simulink library "outp"  (R2021b)
settings: Solver=VariableStepAuto  StartTime=0.0  StopTime=10.0  RelTol=1e-3
undefined symbols (not defined in the file or in its folder): ENUM_PMMMODE_CHARGE, ENUM_PMMMODE_IDLE, ENUM_PMMMODE_INITIALIZE, ENUM_PMMMODE_POWERDOWN, ENUM_PMMMODE_SLEEP, Left, outp, slcm, TRUE
libraries: FVT_lib x736, hcu_lib x4, simulink x1
(part 2 of 8)

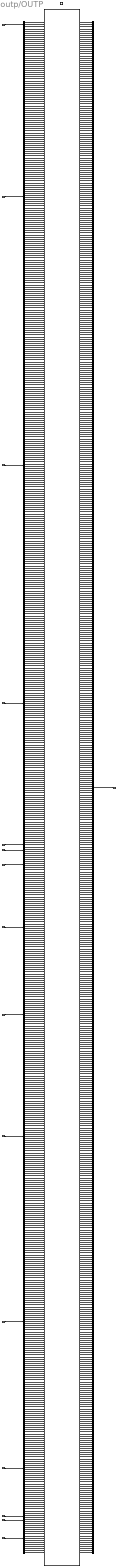
== system outp/OUTP ==
  BACC_outputs : Inport  OutDataTypeStr=Bus: BACC_outputs
  BAPM_outputs : Inport  Port=2  OutDataTypeStr=Bus: BAPM_outputs
  BBCM_outputs : Inport  Port=3  OutDataTypeStr=Bus: BBCM_outputs
  BDDM_outputs : Inport  Port=4  OutDataTypeStr=Bus: BDDM_outputs
  BDHP_outputs : Inport  Port=5  OutDataTypeStr=Bus: BDHP_outputs
  BDKC_outputs : Inport  Port=6  OutDataTypeStr=Bus: BDKC_outputs
  BNMM_outputs : Inport  Port=7  OutDataTypeStr=Bus: BNMM_outputs
  BPMM_outputs : Inport  Port=8  OutDataTypeStr=Bus: BPMM_outputs
  BSYS_outputs : Inport  Port=9  OutDataTypeStr=Bus: BSYS_outputs
  BTHC_outputs : Inport  Port=10  OutDataTypeStr=Bus: BTHC_outputs
  BTPM_outputs : Inport  Port=11  OutDataTypeStr=Bus: BTPM_outputs
  BTQD_outputs : Inport  Port=12  OutDataTypeStr=Bus: BTQD_outputs
  BTQR_outputs : Inport  Port=13  OutDataTypeStr=Bus: BTQR_outputs
  BV2L_outputs : Inport  Port=14  OutDataTypeStr=Bus: BV2L_outputs
  BVMC_outputs : Inport  Port=15  OutDataTypeStr=Bus: BVMC_outputs
  trig_OUTP : TriggerPort  TriggerType=function-call  VariantControl=(inherit)
  bus_creator : BusCreator  Inputs=736
  bus_selector1 : BusSelector  OutputSignals=VACC_HVTHCMSysAvail_enum,VACC_LVBattVoltSta_enum,VACC_VehHVPwrAvail4THCM_W
  bus_selector10 : BusSelector  OutputSignals=VTHC_FDCompCmd_rpm,VTHC_FDSOV1Cmd_flg,VTHC_FDSOV2Cmd_flg,VTHC_FDSOV3Cmd_flg,VTHC_FDEXV1Cmd_step,VTHC_FDEXV2Cmd_step,VTHC_FDSOTXVCmd_flg,VTHC_FDFWVCmd_flg,VTHC_FDTWVCmd_pct,VTHC_FDFrWPTCHeatPwrCmd_W,VTHC_CoolgFanActDuty_pct,VTHC_FDAGSCmd_enum,VTHC_FDEWP1Cmd_enum,VTHC_FDEWP2Cmd_enum,VTHC_FDEWP3Cmd_enum,VTHC_FDFrLeAPTCHeatPwrCmd_W,VTHC_FDFrRiAPTCHeatPwrCmd_W,VTHC_FDRrAPTCHeatPwrCmd_W,VTHC_FDBlowerCmd_pct,VTHC_BatteryMode_enum,VTHC_EDriveMode_enum,VTHC_CabinMode_enum,VTHC_CCUACLampSts_flg,VTHC_CCUAutoLampSts_flg,VTHC_CCUACMaxLampSts_flg,VTHC_CCUSyncLampSts_flg,VTHC_sigAirIntenZon1St_enum,VTHC_sigWindDirZon1St_enum,VTHC_sigRecircSt_flg,VTHC_sigSetTempZon1St_C,VTHC_sigSetTempZon2St_C,VTHC_sigClntTHvBattOut_C,VTHC_sigCbnSolarLeft_W,VTHC_sigClntTHvBattIn_C,VTHC_sigCbnSolarRight_W,VTHC_sigAmbAirT_C,VTHC_sigCbnAirT_C,VTHC_ACSubMode_enum,VTHC_FDRecyAutoCmd_enum,VTHC_ACModeMem_enum,VTHC_Face_flg,VTHC_Foot_flg,VTHC_Frost_flg,VTHC_FaceM_flg,VTHC_FootM_flg,VTHC_CCUSyncSts_flg,VTHC_ACForceOFF_flg,VTHC_RecAutoFlg_flg,VTHC_AirIntenZone1M_enum,VTHC_fdefog_flg,VTHC_sigSetTempZon2StM_C,VTHC_sigDfrstSt_flg,VTHC_FDCTHCAirIntZ3Sta_enum,VTHC_FDCTHCDrEVentModeSta_enum,VTHC_FDCTHCPsEVentModeSta_enum,VTHC_FDCTHCDrEVentZSta_enum,VTHC_FDCTHCCLEVentZSta_enum,VTHC_FDCTHCPsEVentZSta_enum,VTHC_FDCTHCCREVentZSta_enum,VTHC_FDCTHCDrEVentYSta_enum,VTHC_FDCTHCDrVentENSta_flg,VTHC_FDCTHCCLEVentYSta_enum,VTHC_FDCTHCCLVentENSta_flg,VTHC_FDCTHCPsEVentYSta_enum,VTHC_FDCTHCPsVentENSta_flg,VTHC_FDCTHCCREVentYSta_enum,VTHC_FDCTHCCRVentENSta_flg,VTHC_FDCTHCMAPTCForceOFFSta_flg,VTHC_DrVentEN_flg,VTHC_CLVentEN_flg,VTHC_PsVentEN_flg,VTHC_CRVentEN_flg,VTHC_FDCFGSAirIntSta_enum,VTHC_FDCFGSChSta_enum,VTHC_FDCFGSAirIntCmd_enum,VTHC_FDCFGSFuncSta_flg,VTHC_FDCFGSChCmd_enum,VTHC_FDCFGSIONSWSta_flg,VTHC_FDCFGSIONCmd_flg,VTHC_FDCFGSLearnCmd_enum,VTHC_FDCTHCMPreWPTCHeatSta_enum
  bus_selector11 : BusSelector  OutputSignals=VTPM_LFBatWarn_flg,VTPM_RFBatWarn_flg,VTPM_LRBatWarn_flg,VTPM_RRBatWarn_flg,VTPM_LFWheelPress_raw8,VTPM_RFWheelPress_raw8,VTPM_LRWheelPress_raw8,VTPM_RRWheelPress_raw8,VTPM_LFWheelTemp_C,VTPM_RFWheelTemp_C,VTPM_LRWheelTemp_C,VTPM_RRWheelTemp_C,VTPM_LFSensorFail_flg,VTPM_RFSensorFail_flg,VTPM_LRSensorFail_flg,VTPM_RRSensorFail_flg,VTPM_LFWheelDebug_flg,VTPM_LRWheelDebug_flg,VTPM_RFWheelDebug_flg,VTPM_RRWheelDebug_flg,VTPM_TPMSResButtAllow_flg,VTPM_TPMSCaliButtAllow_flg,VTPM_LFPressIndi_enum,VTPM_RFPressIndi_enum,VTPM_LRPressIndi_enum,VTPM_RRPressIndi_enum,VTPM_TPMSWarnIndi_enum,VTPM_LFWheelTmpIndi_flg,VTPM_RFWheelTmpIndi_flg,VTPM_LRWheelTmpIndi_flg,VTPM_RRWheelTmpIndi_flg,VTPM_LFWheelPSW_raw8,VTPM_LRWheelPSW_raw8,VTPM_RFWheelPSW_raw8,VTPM_RRWheelPSW_raw8,VTPM_CWheelTips_enum,VTPM_AutoLTips_enum,VTPM_LFSensorMode_flg,VTPM_RFSensorMode_flg,VTPM_LRSensorMode_flg,VTPM_RRSensorMode_flg,VTPM_S1ID_raw32,VTPM_S2ID_raw32,VTPM_S3ID_raw32,VTPM_S4ID_raw32,VTPM_S1L_enum,VTPM_S2L_enum,VTPM_S3L_enum,VTPM_S4L_enum,VTPM_ALFin_flg,VTPM_LFP20_raw8,VTPM_RFP20_raw8,VTPM_LRP20_raw8,VTPM_RRP20_raw8,VTPM_FAT_flg,VTPM_IDin_raw32,VTPM_S1WheelDebugALTU_pct,VTPM_S2WheelDebugALTU_pct,VTPM_S3WheelDebugALTU_pct,VTPM_S4WheelDebugALTU_pct,VTPM_ID1messageALTU_raw8,VTPM_ID2messageALTU_raw8,VTPM_ID3messageALTU_raw8,VTPM_ID4messageALTU_raw8,VTPM_Chkfin_flg,VTPM_SetIDLoc_flg,VTPM_TPMSStorge_flg,VTPM_ChkStorge_flg,VTPM_TPMSResButt_flg,VTPM_LFPindi_enum,VTPM_RFPind_enum,VTPM_LRPindi_enum,VTPM_RRPindi_enum,VTPM_WriteChkLFID_raw,VTPM_WriteChkRFID_raw,VTPM_WriteChkLRID_raw,VTPM_WriteChkRRID_raw,VTPM_WriteChkfinLFID_raw,VTPM_WriteChkfinRFID_raw,VTPM_WriteChkfinLRID_raw,VTPM_WriteChkfinRRID_raw,VTPM_Flashchkdatavalid_enum,VTPM_Flashdatavalid_enum,VTPM_unlearnSfali_flg,VTPM_unlearnSfailvalid_enum,VTPM_Prepresstempvalid_enum,VTPM_FlashS1ID_raw,VTPM_FlashS2ID_raw,VTPM_FlashS3ID_raw,VTPM_FlashS4ID_raw,VTPM_FlashIDvalid_enum,VTPM_WritingCnt_enum,VTPM_TPMSTLCmd_flg,VTPM_LProgress_enum,VTPM_TPMSSensorIDRegStart_flg,VTPM_ModelVersion_raw,VTPM_ModelVersionChksum_raw
  bus_selector12 : BusSelector  OutputSignals=VTQD_ParkRequest_flg,VTQD_TqSourceFr_enum,VTQD_TqSourceRr_enum,VTQD_FrEDUAvailBrkRgnTq_Nm,VTQD_RrEDUAvailBrkRgnTq_Nm,VTQD_EVDriveMode_enum,VTQD_ShiftGearPosn_enum,VTQD_PButtonSta_enum,VTQD_FrActvDmpDisabReq_flg,VTQD_RrActvDmpDisabReq_flg,VTQD_FrRgnDecrSta_flg,VTQD_RrRgnDecrSta_flg,VTQD_DriverWhlTqDemFr_Nm,VTQD_DriverWhlTqDemRr_Nm,VTQD_FrEDUActTq_Nm,VTQD_RrEDUActTq_Nm,VTQD_FrEDURolRgnTq_Nm,VTQD_RrEDURolRgnTq_Nm,VTQD_FrEDUSpd_rpm,VTQD_RrEDUSpd_rpm,VTQD_FrEDUSpdValid_flg,VTQD_FrEDUAvailBrkRgnTqV_flg,VTQD_RrEDUSpdValid_flg,VTQD_RrEDUAvailBrkRgnTqV_flg,VTQD_RgnAbnorSta_flg,VTQD_PTCSPermSta_flg,VTQD_FrRgnPermSta_flg,VTQD_RrRgnPermSta_flg,VTQD_FrIdcMin_A,VTQD_FrIdcMax_A,VTQD_FrUdcMin_V,VTQD_FrUdcMax_V,VTQD_RrIdcMin_A,VTQD_RrIdcMax_A,VTQD_RrUdcMin_V,VTQD_RrUdcMax_V,VTQD_ReBrakeLPReq_flg,VTQD_CreepON_flg,VTQD_EquivAccPedalSWSta_flg,VTQD_DriveProtEn_flg,VTQD_ActParkRequest_flg,VTQD_IVIPwrLockSta_enum,VTQD_OPDHoldLamp_flg,VTQD_VehActSpd_kph
  bus_selector13 : BusSelector  OutputSignals=VTQR_FrTMTqReq_Nm,VTQR_RrTMTqReq_Nm
  bus_selector14 : BusSelector  OutputSignals=VV2L_ReqOBCV2LEna_enum,VV2L_ReqV2LIVIPopup_enum
  bus_selector15 : BusSelector  OutputSignals=VVMC_ACCCtrlAvail_flg,VVMC_ACCPedalOvrd_flg,VVMC_CCCtrlSta_enum,VVMC_CCMSASpdWar_flg,VVMC_MSACtrlSta_enum,VVMC_APSCtrlAvail_flg,VVMC_APSActive_flg,VVMC_APSStaSys_enum,VVMC_APSDecReqA_flg,VVMC_APSDecReq_mps2,VVMC_APSReq_enum,VVMC_IMUEnaCmd_flg,VVMC_CAASCtrlAvail_flg,VVMC_CAASActive_flg,VVMC_ExtraMSACtrlSta_enum
  bus_selector2 : BusSelector  OutputSignals=VAPM_VehSpeed_kph,VAPM_VehSpeedTimeOut_flg,VAPM_FSOffSw_enum,VAPM_FSOffSwTimeOut_flg,VAPM_ChrgPlugSta_enum,VAPM_PASDRMR_cm,VAPM_PASDRML_cm,VAPM_PASDRCR_cm,VAPM_PASDRCL_cm,VAPM_PASDFMR_cm,VAPM_PASDFML_cm,VAPM_PASDFCR_cm,VAPM_PASDFCL_cm,VAPM_APSDRLR_cm,VAPM_APSDRLL_cm,VAPM_APSDFLR_cm,VAPM_APSDFLL_cm,VAPM_PASAFCL_enum,VAPM_PASARMR_enum,VAPM_PASARML_enum,VAPM_PASARCR_enum,VAPM_PASARCL_enum,VAPM_PASAFMR_enum,VAPM_PASAFML_enum,VAPM_PASAFCR_enum,VAPM_USSStaRMR_flg,VAPM_USSStaRML_flg,VAPM_USSStaRLR_flg,VAPM_USSStaRLL_flg,VAPM_USSStaRCR_flg,VAPM_USSStaRCL_flg,VAPM_USSStaFMR_flg,VAPM_USSStaFML_flg,VAPM_USSStaFLR_flg,VAPM_USSStaFLL_flg,VAPM_USSStaFCR_flg,VAPM_USSStaFCL_flg,VAPM_Chime_enum,VAPM_SNSRLayout_enum,VAPM_StaFSya_flg,VAPM_ModOperation_enum,VAPM_BrkPedalPos_pct,VAPM_BrkPedalPosTimeOut_flg,VAPM_LFRawWhlSpeed_kph,VAPM_LFRawWhlSpeedTimeOut_flg,VAPM_RFRawWhlSpeed_kph,VAPM_RFRawWhlSpeedTimeOut_flg,VAPM_LRRawWhlSpeed_kph,VAPM_LRRawWhlSpeedTimeOut_flg,VAPM_RRRawWhlSpeed_kph,VAPM_RRRawWhlSpeedTimeOut_flg,VAPM_LFRawWhlSpeedV_flg,VAPM_LFRawWhlSpeedVTimeOut_flg,VAPM_RFRawWhlSpeedV_flg,VAPM_RFRawWhlSpeedVTimeOut_flg,VAPM_LRRawWhlSpeedV_flg,VAPM_LRRawWhlSpeedVTimeOut_flg,VAPM_RRRawWhlSpeedV_flg,VAPM_RRRawWhlSpeedVTimeOut_flg,VAPM_LFWhlRotDir_enum,VAPM_LFWhlRotDirTimeOut_flg,VAPM_RFWhlRotDir_enum,VAPM_RFWhlRotDirTimeOut_flg,VAPM_LRWhlRotDir_enum,VAPM_LRWhlRotDirTimeOut_flg,VAPM_RRWhlRotDir_enum,VAPM_RRWhlRotDirTimeOut_flg,VAPM_LFPulseCountV_flg,VAPM_LFPulseCountVTimeOut_flg,VAPM_RFPulseCountV_flg,VAPM_RFPulseCountVTimeOut_flg,VAPM_LRPulseCountV_flg,VAPM_LRPulseCountVTimeOut_flg,VAPM_RRPulseCountV_flg,VAPM_RRPulseCountVTimeOut_flg,VAPM_LFPulseCount_enum,VAPM_LFPulseCountTimeOut_flg,VAPM_RFPulseCount_enum,VAPM_RFPulseCountTimeOut_flg,VAPM_LRPulseCount_enum,VAPM_LRPulseCountTimeOut_flg,VAPM_RRPulseCount_enum,VAPM_RRPulseCountTimeOut_flg,VAPM_ShifterHandleCmd_enum,VAPM_ShifterHandleCmdTimeOut_flg,VAPM_DriIntend_enum,VAPM_DriIntendTimeOut_flg,VAPM_EPSAOIControl_enum,VAPM_EPSAOIControlTimeOut_flg,VAPM_SASAngle_Deg,VAPM_SASAngleTimeOut_flg,VAPM_SASSpeed_degps,VAPM_SASSpeedTimeOut_flg,VAPM_SASSpeedValid_flg,VAPM_SASSpeedValidTimeOut_flg,VAPM_SASCAL_flg,VAPM_SASCALTimeOut_flg,VAPM_SASV_flg,VAPM_SASVTimeOut_flg,VAPM_GRADE_Deg,VAPM_GRADETimeOut_flg,VAPM_YawRate_degps,VAPM_YawRateTimeOut_flg,VAPM_LatAccel_Gps,VAPM_LatAccelTimeOut_flg,VAPM_LongAccel_Gps,VAPM_LongAccelTimeOut_flg,VAPM_MCPressure_bar,VAPM_MCPressureTimeOut_flg,VAPM_YawRateV_flg,VAPM_YawRateVTimeOut_flg,VAPM_LatAccelV_flg,VAPM_LatAccelVTimeOut_flg,VAPM_LongAccelV_flg,VAPM_LongAccelVTimeOut_flg,VAPM_MCPressureV_bar,VAPM_MCPressureVTimeOut_flg,VAPM_BrkSwSta_flg,VAPM_BrkSwStaTimeOut_flg,VAPM_BrkSwV_flg,VAPM_BrkSwVTimeOut_flg,VAPM_ESCStandstill_flg,VAPM_ESCStandstillTimeOut_flg,VAPM_ESCAPSSta_enum,VAPM_ESCAPSStaTimeOut_flg,VAPM_EPBExtReleaseAvail_flg,VAPM_EPBExtReleaseAvailTimeOut_flg,VAPM_EPBExtApplyAvail_flg,VAPM_EPBExtApplyAvailTimeOut_flg,VAPM_EPBErrSta_enum,VAPM_EPBErrStaTimeOut_flg,VAPM_EPBSta_enum,VAPM_EPBStaTimeOut_flg,VAPM_AVMparkingcancel_enum,VAPM_AVMparkingcancelTimeOut_flg,VAPM_AVMparkingexcute_enum,VAPM_AVMparkingexcuteTimeOut_flg,VAPM_AVMParkingmode_enum,VAPM_AVMParkingmodeTimeOut_flg,VAPM_AVMErrSTA_flg,VAPM_AVMErrSTATimeOut_flg,VAPM_IVIStatus_flg,VAPM_IVIStatusTimeOut_flg,VAPM_CAASSw_enum,VAPM_CAASSwTimeOut_flg,VAPM_IVIScreen_enum,VAPM_IVIScreenTimeOut_flg,VAPM_ABSActive_flg,VAPM_ABSActiveTimeOut_flg,VAPM_TCSActive_flg,VAPM_TCSActiveTimeOut_flg,VAPM_DriverSeatBeltCmd_flg,VAPM_DriverSeatBeltCmdTimeOut_flg,VAPM_APSProgressPCT_pct,VAPM_APSRQDisplay_enum,VAPM_APSSWVer_enum,VAPM_APSHWVer_enum,VAPM_APSExitCondition_enum,VAPM_APSAngleTarget_Deg,VAPM_APSVRqEPASCtrl_flg,VAPM_APSRqEPASCtrl_flg,VAPM_CAASSta_enum
  bus_selector3 : BusSelector  OutputSignals=VBCM_AntitheftSta_enum,VBCM_TailgateRemote_enum,VBCM_HornCtrl_flg,VBCM_AllDoorSW_flg,VBCM_BCMDoorLockSta_flg,VBCM_AntitheftSeatFlod_flg,VBCM_HoodSW_flg,VBCM_TailgateSW_flg,VBCM_DrDoorSW_flg,VBCM_PsDoorSW_flg,VBCM_RLDoorSW_flg,VBCM_RRDoorSW_flg,VBCM_LockSetting_flg,VBCM_FrChargingDoorCtrl_enum,VBCM_RrChargingDoorCtrl_enum,VBCM_CrashDetd_flg,VBCM_CTDCtrl_enum,VBCM_DoorLockIND_flg,VBCM_CTDLockSW_flg,VBCM_Dimmer_pct,VBCM_DimmerEN_flg,VBCM_PosLamp_flg,VBCM_LBeam_flg,VBCM_HBeam_flg,VBCM_RrFogLamp_flg,VBCM_BrakeLamp_flg,VBCM_ReverseLamp_flg,VBCM_LDRL_flg,VBCM_RDRL_flg,VBCM_LBSD_flg,VBCM_RBSD_flg,VBCM_HazardSW_flg,VBCM_LTurnLP_flg,VBCM_RTurnLP_flg,VBCM_BCMBuzzerReq_flg,VBCM_MirrorCtrl_enum,VBCM_MirrorDefog_flg,VBCM_RrDefog_flg,VBCM_RoomLampH_flg,VBCM_RoomLampL_flg,VBCM_TrunkRel_flg,VBCM_TailgateHDSW_flg,VBCM_FrWiperL_flg,VBCM_FrWiperH_flg,VBCM_RrWiper_flg,VBCM_WasherCtrl_enum,VBCM_WiperFixMode_flg,VBCM_User1DrAmbLightBrightness_enum,VBCM_User1IPAmbLightBrightness_enum,VBCM_User2DrAmbLightBrightness_enum,VBCM_User2IPAmbLightBrightness_enum,VBCM_User3DrAmbLightBrightness_enum,VBCM_User3IPAmbLightBrightness_enum,VBCM_User4DrAmbLightBrightness_enum,VBCM_User4IPAmbLightBrightness_enum,VBCM_User5DrAmbLightBrightness_enum,VBCM_User5IPAmbLightBrightness_enum,VBCM_User6DrAmbLightBrightness_enum,VBCM_User6IPAmbLightBrightness_enum,VBCM_User1AmbLightColor_enum,VBCM_User2AmbLightColor_enum,VBCM_User3AmbLightColor_enum,VBCM_User4AmbLightColor_enum,VBCM_User5AmbLightColor_enum,VBCM_User6AmbLightColor_enum,VBCM_AmbLightBreath1_flg,VBCM_AmbLightBreath2_flg,VBCM_AmbLightBreath3_flg,VBCM_AmbLightBrightness1_enum,VBCM_AmbLightBrightness2_enum,VBCM_AmbLightBrightness3_enum,VBCM_AmbLightColor1_enum,VBCM_AmbLightColor2_enum,VBCM_AmbLightColor3_enum,VBCM_LampPwr_flg,VBCM_SPTGDet_flg,VBCM_APSOpenPTG_flg,VBCM_FollowMe_flg,VBCM_IVIRST_flg,VBCM_CountAlarm_enum,VBCM_MFSWTri_flg,VBCM_MirrorFlodPos_flg,VBCM_FuelDoorPos_flg,VBCM_MFRDNBrightReq_pct,VBCM_RoomLampMode_flg,VBCM_IVIPTGUSStaSW_flg,VBCM_PTGInnerSW2_enum,VBCM_LDrvCtrlCmd_pct,VBCM_LPasCtrlCmd_pct,VBCM_LRLDCtrlCmd_pct,VBCM_LRRDCtrlCmd_pct,VBCM_APMDoorControlSta_flg,VBCM_LockAlarm_enum,VBCM_ATCtrl_enum,VBCM_fUnlockSingle_flg,VBCM_OutMode_enum
  bus_selector4 : BusSelector  OutputSignals=VDDM_C3BMS6RCDTC_raw32,VDDM_C3BMS6CSDTC_raw32,VDDM_C3BMS6LCDTC_raw32,VDDM_C3BMS1RCDTC_raw32,VDDM_C3BMS1CSDTC_raw32,VDDM_C3BMS1LCDTC_raw32,VDDM_C3CCU1RCDTC_raw32,VDDM_C3CCU1CSDTC_raw32,VDDM_C3CCU1LCDTC_raw32,VDDM_C3CCU2RCDTC_raw32,VDDM_C3CCU2CSDTC_raw32,VDDM_C3CCU2LCDTC_raw32,VDDM_C1ABM1RCDTC_raw32,VDDM_C1ABM1CSDTC_raw32,VDDM_C1ABM1LCDTC_raw32,VDDM_Lv1ErrDTC_raw32,VDDM_Lv2ErrDTC_raw32,VDDM_Lv3ErrDTC_raw32,VDDM_Lv4ErrDTC_raw32,VDDM_BrkSWErrDTC_raw32,VDDM_BrkSWNoBacDTC_raw32,VDDM_KeyAuthDTC_raw32,VDDM_ONtoRdyDTC_raw32,VDDM_HVB4PreDTC_raw32,VDDM_MCU4PreDTC_raw32,VDDM_DCDC4PreDTC_raw32,VDDM_HVRlyCloDTC_raw32,VDDM_BMSRdyDTC_raw32,VDDM_DCDCEnaDTC_raw32,VDDM_HiLvSaChkDTC_raw32,VDDM_MidLvSaChkDTC_raw32,VDDM_MCUDisDTC_raw32,VDDM_DCDCDisDTC_raw32,VDDM_HVRlyOpDTC_raw32,VDDM_MCUActDTC_raw32,VDDM_OBC4PreDTC_raw32,VDDM_IniLVLoDTC_raw32,VDDM_LVSupLoDTC_raw32,VDDM_LVSupHiDTC_raw32,VDDM_DrStSWDTC_raw32,VDDM_FLDoorSWDTC_raw32,VDDM_RLDoorSWDTC_raw32,VDDM_FRDoorSWDTC_raw32,VDDM_RRDoorSWDTC_raw32,VDDM_HoodSWDTC_raw32,VDDM_TailgaSWDTC_raw32,VDDM_VehMalfunLevel_enum,VDDM_APS1SigOoRDTC_raw32,VDDM_APS2SigOoRDTC_raw32,VDDM_APSCorrErrDTC_raw32,VDDM_MCUF1NoComDTC_raw32,VDDM_MCUR1NoComDTC_raw32,VDDM_Shifter1NoComDTC_raw32,VDDM_ESC7NoComDTC_raw32,VDDM_ESC1NoComDTC_raw32,VDDM_ESC5NoComDTC_raw32,VDDM_EnterNewOperCyc_flg,VDDM_DiagHCrashDTC_raw32,VDDM_DiagFLTSDTC_raw32,VDDM_DiagFRTSDTC_raw32,VDDM_DiagRLTSDTC_raw32,VDDM_DiagRRTSDTC_raw32,VDDM_FCLUSSDTC_raw32,VDDM_FMLUSSDTC_raw32,VDDM_FMRUSSDTC_raw32,VDDM_FCRUSSDTC_raw32,VDDM_RCLUSSDTC_raw32,VDDM_RMLUSSDTC_raw32,VDDM_RMRUSSDTC_raw32,VDDM_RCRUSSDTC_raw32,VDDM_FLLUSSDTC_raw32,VDDM_FLRUSSDTC_raw32,VDDM_RLLUSSDTC_raw32,VDDM_RLRUSSDTC_raw32,VDDM_FCM2NoComDTC_raw32,VDDM_FCM2RCErrDTC_raw32,VDDM_FCM2CSErrDTC_raw32,VDDM_FCM3NoComDTC_raw32,VDDM_FCM3RCErrDTC_raw32,VDDM_FCM3CSErrDTC_raw32,VDDM_FCM4NoComDTC_raw32,VDDM_FCM4CSErrDTC_raw32,VDDM_FCM5NoComDTC_raw32,VDDM_FCM5CSErrDTC_raw32,VDDM_ZoneSCPNoComDTC_raw32,VDDM_BMSSigErrDetDTC_raw32,VDDM_FCMACCSigErrDetDTC_raw32,VDDM_FrMCUSigErrDetDTC_raw32,VDDM_RrMCUSigErrDetDTC_raw32,VDDM_CCUSigErrDetDTC_raw32,VDDM_ACCAccelCmdErrDetDTC_raw32,VDDM_ACCMalfuncDetDTC_raw32,VDDM_CCMalfuncDetDTC_raw32,VDDM_MSAMalfuncDetDTC_raw32,VDDM_ISAMalfuncDetDTC_raw32,VDDM_MCUF1RCErrDTC_raw32,VDDM_MCUR1RCErrDTC_raw32,VDDM_MCUF1CSErrDTC_raw32,VDDM_MCUR1CSErrDTC_raw32,VDDM_Shifter1RCErrDTC_raw32,VDDM_Shifter1CSErrDTC_raw32,VDDM_ESC7RCErrDTC_raw32,VDDM_ESC7CSErrDTC_raw32,VDDM_ESC1RCErrDTC_raw32,VDDM_ESC1CSErrDTC_raw32,VDDM_ESC5RCErrDTC_raw32,VDDM_ESC5CSErrDTC_raw32,VDDM_FrMCUTqErrDTC_raw32,VDDM_RrMCUTqErrDTC_raw32,VDDM_LFBatwarnDTC_raw32,VDDM_RFBatwarnDTC_raw32,VDDM_LRBatwarnDTC_raw32,VDDM_RRBatwarnDTC_raw32,VDDM_LFPressIndiDTC_raw32,VDDM_RFPressIndiDTC_raw32,VDDM_LRPressIndiDTC_raw32,VDDM_RRPressIndiDTC_raw32,VDDM_LFWheelTmpHighDTC_raw32,VDDM_RFWheelTmpHighDTC_raw32,VDDM_LRWheelTmpHighDTC_raw32,VDDM_RRWheelTmpHighDTC_raw32,VDDM_LFSensorFailDTC_raw32,VDDM_RFSensorFailDTC_raw32,VDDM_LRSensorFailDTC_raw32,VDDM_RRSensorFailDTC_raw32,VDDM_C1EPAS2LCDTC_raw32,VDDM_5vAPS1PwrErrDTC_raw32,VDDM_5vAPS2PwrErrDTC_raw32,VDDM_EPBLockTODTC_raw32,VDDM_EPBUnlockTODTC_raw32,VDDM_THCMAPTCWarning_raw32,VDDM_LimpHomeActTmp_flg,VDDM_EDriveSysErr_VCUErrTmp_flg
  bus_selector5 : BusSelector  OutputSignals=VDHP_ActAPSPosn_pct,VDHP_EAPS1MIN_pct,VDHP_EAPS2MIN_pct
  bus_selector6 : BusSelector  OutputSignals=VDKC_DKCTimeSN_cnt,VDKC_DKCAuthSta_enum
  bus_selector7 : BusSelector  OutputSignals=VNMM_AllCANTxReq_flg,VNMM_NMmTxReq_flg,VNMM_Awake_enum,VNMM_CSB_flg,VNMM_ErrorState_enum,VNMM_NodeID_enum,VNMM_PNI_flg,VNMM_RptMsgReq_flg,VNMM_WakeUp_enum,VNMM_ActiveWU_flg,VNMM_SysNMmSta_enum,VNMM_NetworkReq_flg
  bus_selector8 : BusSelector  OutputSignals=VPMM_PowerUpState_enum,VPMM_PowerDownState_enum,VPMM_PowerUpFault_enum,VPMM_PowerDownFault_enum,VPMM_ActiveDischargeReq_flg,VPMM_DCDCEnaReq_flg,VPMM_DCDCVoltSetpoint_V,VPMM_HVBatCnctReq_flg,VPMM_HVSysReadyToCharge_enum,VPMM_PowerSta_enum,VPMM_LVPwrSta_flg,VPMM_HVPwrSta_flg,VPMM_SysPowerMode_enum,VPMM_FrMCUEnaReq_flg,VPMM_RrMCUEnaReq_flg,VPMM_DrivetrainSelect_enum,VPMM_DrSeatSta_enum,VPMM_PwrStaSelect_enum,VPMM_PwrStaConstraint_enum,VPMM_TCountSta_enum,VPMM_PwrUpReq_enum,VPMM_PwrDownReq_enum,VPMM_LowSOCWarn_enum,VPMM_ReVehThdChkSta_enum,VPMM_LVSysErrPwrOutErr_flg,VPMM_EvccAplusPwrUpReq_flg,VPMM_PwrStaONTOPopReq_flg,VPMM_IVIPwrStaONTOPopT_s,VPMM_LVChrgHoldTtimer_s,VPMM_LVBattChrgTimeCnt_s,VPMM_SilentChkAllowSleep_flg,VPMM_TimerAllowSleep_flg,VPMM_FDADC12VDetAvg_mV,VPMM_PMMAllowECUSleep_flg,VPMM_LVSilentChrgSta_enum,VPMM_LVSilentChrgReq_flg,VPMM_LVSilentChrgLv_enum,VPMM_CtrlFrPwrStbA1P_flg,VPMM_CtrlFrRC1_flg,VPMM_CtrlFrBMSCCUCIR_flg,VPMM_CtrlFrEDUINVERTER_flg,VPMM_HWResetSta_enum,VPMM_CtrlDrPwrStbA2_flg,VPMM_PwrStaTOSta_enum,VPMM_Sched_ChgTOSta_enum,VPMM_PwrReq_OTA_enum,VPMM_OTAPwrReqOFFChkSta_enum,VPMM_OTAPwrReqStdChkSta_enum
  bus_selector9 : BusSelector  OutputSignals=VSYS_HWVer1_cnt,VSYS_HWVer2_cnt,VSYS_HWVer3_cnt,VSYS_CarModel1_cnt,VSYS_CarModel2_cnt,VSYS_CarModel3_cnt,VSYS_ECU1_cnt,VSYS_ECU2_cnt,VSYS_Major1_cnt,VSYS_Major2_cnt,VSYS_Minor1_cnt,VSYS_Minor2_cnt,VSYS_Patch1_cnt,VSYS_Patch2_cnt,VSYS_Country1_cnt,VSYS_Country2_cnt,VSYS_Variation_cnt,VSYS_Dash1_cnt,VSYS_Change1_cnt,VSYS_Change2_cnt,VSYS_Dash2_cnt,VSYS_SHA1_cnt,VSYS_SHA2_cnt,VSYS_SHA3_cnt,VSYS_SHA4_cnt,VSYS_SHA5_cnt,VSYS_SHA6_cnt,VSYS_SHA7_cnt,VSYS_SHA8_cnt,VSYS_NvWriteReqRisingEdge_flg,VSYS_FdcSlpReqRisingEdge_flg,VSYS_FdcSlpTime_sec,VSYS_PmicBootReason_enum,VSYS_WisrBootReason_raw32,VSYS_AcoreRebootCmdACK_flg,VSYS_CurrentNmState_enum
  outpmodule : Subsystem
  BOUTP_outputs : Outport  OutDataTypeStr=Bus: BOUTP_outputs
  wires:
  outpmodule/279(VOUTP_Lv3ErrDTC_raw32) -> bus_creator/279
  outpmodule/275(VOUTP_C1ABM1CSDTC_raw32) -> bus_creator/275
  outpmodule/274(VOUTP_C1ABM1RCDTC_raw32) -> bus_creator/274
  outpmodule/272(VOUTP_C3CCU2CSDTC_raw32) -> bus_creator/272
  outpmodule/269(VOUTP_C3CCU1CSDTC_raw32) -> bus_creator/269
  outpmodule/266(VOUTP_C3BMS1CSDTC_raw32) -> bus_creator/266
  outpmodule/265(VOUTP_C3BMS1RCDTC_raw32) -> bus_creator/265
  outpmodule/263(VOUTP_C3BMS6CSDTC_raw32) -> bus_creator/263
  outpmodule/260(VOUTP_fUnlockSingle_flg) -> bus_creator/260
  outpmodule/261(VOUTP_OutMode_enum) -> bus_creator/261
  outpmodule/259(VOUTP_ATCtrl_enum) -> bus_creator/259
  outpmodule/258(VOUTP_LockAlarm_enum) -> bus_creator/258
  outpmodule/257(VOUTP_APMDoorControlSta_flg) -> bus_creator/257
  outpmodule/256(VOUTP_LRRDCtrlCmd_pct) -> bus_creator/256
  outpmodule/255(VOUTP_LRLDCtrlCmd_pct) -> bus_creator/255
  outpmodule/251(VOUTP_IVIPTGUSStaSW_flg) -> bus_creator/251
  outpmodule/253(VOUTP_LDrvCtrlCmd_pct) -> bus_creator/253
  outpmodule/252(VOUTP_PTGInnerSW2_enum) -> bus_creator/252
  outpmodule/249(VOUTP_MFRDNBrightReq_pct) -> bus_creator/249
  outpmodule/246(VOUTP_MFSWTri_flg) -> bus_creator/246
  outpmodule/243(VOUTP_FollowMe_flg) -> bus_creator/243
  outpmodule/242(VOUTP_APSOpenPTG_flg) -> bus_creator/242
  outpmodule/241(VOUTP_SPTGDet_flg) -> bus_creator/241
  outpmodule/238(VOUTP_AmbLightColor2_enum) -> bus_creator/238
  outpmodule/237(VOUTP_AmbLightColor1_enum) -> bus_creator/237
  outpmodule/236(VOUTP_AmbLightBrightness3_enum) -> bus_creator/236
  outpmodule/234(VOUTP_AmbLightBrightness1_enum) -> bus_creator/234
  outpmodule/232(VOUTP_AmbLightBreath2_flg) -> bus_creator/232
  bus_selector2/54 -> outpmodule/57(VAPM_RFRawWhlSpeedV_flg)  "<VAPM_RFRawWhlSpeedV_flg>"
  bus_selector2/33 -> outpmodule/36(VAPM_USSStaFML_flg)  "<VAPM_USSStaFML_flg>"
  bus_selector2/47 -> outpmodule/50(VAPM_RFRawWhlSpeedTimeOut_flg)  "<VAPM_RFRawWhlSpeedTimeOut_flg>"
  bus_selector2/41 -> outpmodule/44(VAPM_ModOperation_enum)  "<VAPM_ModOperation_enum>"
  bus_selector3/14 -> outpmodule/179(VBCM_FrChargingDoorCtrl_enum)  "<VBCM_FrChargingDoorCtrl_enum>"
  bus_selector3/15 -> outpmodule/180(VBCM_RrChargingDoorCtrl_enum)  "<VBCM_RrChargingDoorCtrl_enum>"
  bus_selector3/11 -> outpmodule/176(VBCM_RLDoorSW_flg)  "<VBCM_RLDoorSW_flg>"
  bus_selector3/9 -> outpmodule/174(VBCM_DrDoorSW_flg)  "<VBCM_DrDoorSW_flg>"
  bus_selector3/8 -> outpmodule/173(VBCM_TailgateSW_flg)  "<VBCM_TailgateSW_flg>"
  bus_selector3/10 -> outpmodule/175(VBCM_PsDoorSW_flg)  "<VBCM_PsDoorSW_flg>"
  bus_selector3/7 -> outpmodule/172(VBCM_HoodSW_flg)  "<VBCM_HoodSW_flg>"
  bus_selector3/2 -> outpmodule/167(VBCM_TailgateRemote_enum)  "<VBCM_TailgateRemote_enum>"
  bus_selector3/4 -> outpmodule/169(VBCM_AllDoorSW_flg)  "<VBCM_AllDoorSW_flg>"
  bus_selector3/5 -> outpmodule/170(VBCM_BCMDoorLockSta_flg)  "<VBCM_BCMDoorLockSta_flg>"
  bus_selector3/3 -> outpmodule/168(VBCM_HornCtrl_flg)  "<VBCM_HornCtrl_flg>"
  bus_selector4/115 -> outpmodule/376(VDDM_RFPressIndiDTC_raw32)  "<VDDM_RFPressIndiDTC_raw32>"
  bus_selector3/72 -> outpmodule/237(VBCM_AmbLightColor1_enum)  "<VBCM_AmbLightColor1_enum>"
  bus_selector3/66 -> outpmodule/231(VBCM_AmbLightBreath1_flg)  "<VBCM_AmbLightBreath1_flg>"
  bus_selector3/61 -> outpmodule/226(VBCM_User2AmbLightColor_enum)  "<VBCM_User2AmbLightColor_enum>"
  bus_selector3/59 -> outpmodule/224(VBCM_User6IPAmbLightBrightness_enum)  "<VBCM_User6IPAmbLightBrightness_enum>"
  bus_selector3/52 -> outpmodule/217(VBCM_User3DrAmbLightBrightness_enum)  "<VBCM_User3DrAmbLightBrightness_enum>"
  bus_selector3/51 -> outpmodule/216(VBCM_User2IPAmbLightBrightness_enum)  "<VBCM_User2IPAmbLightBrightness_enum>"
  bus_selector3/50 -> outpmodule/215(VBCM_User2DrAmbLightBrightness_enum)  "<VBCM_User2DrAmbLightBrightness_enum>"
  bus_selector3/47 -> outpmodule/212(VBCM_WiperFixMode_flg)  "<VBCM_WiperFixMode_flg>"
  bus_selector3/46 -> outpmodule/211(VBCM_WasherCtrl_enum)  "<VBCM_WasherCtrl_enum>"
  bus_selector3/48 -> outpmodule/213(VBCM_User1DrAmbLightBrightness_enum)  "<VBCM_User1DrAmbLightBrightness_enum>"
  bus_selector3/44 -> outpmodule/209(VBCM_FrWiperH_flg)  "<VBCM_FrWiperH_flg>"
  bus_selector3/42 -> outpmodule/207(VBCM_TailgateHDSW_flg)  "<VBCM_TailgateHDSW_flg>"
  bus_selector3/41 -> outpmodule/206(VBCM_TrunkRel_flg)  "<VBCM_TrunkRel_flg>"
  bus_selector3/39 -> outpmodule/204(VBCM_RoomLampH_flg)  "<VBCM_RoomLampH_flg>"
  bus_selector3/40 -> outpmodule/205(VBCM_RoomLampL_flg)  "<VBCM_RoomLampL_flg>"
  bus_selector3/37 -> outpmodule/202(VBCM_MirrorDefog_flg)  "<VBCM_MirrorDefog_flg>"
  bus_selector3/35 -> outpmodule/200(VBCM_BCMBuzzerReq_flg)  "<VBCM_BCMBuzzerReq_flg>"
  bus_selector3/36 -> outpmodule/201(VBCM_MirrorCtrl_enum)  "<VBCM_MirrorCtrl_enum>"
  bus_selector3/32 -> outpmodule/197(VBCM_HazardSW_flg)  "<VBCM_HazardSW_flg>"
  bus_selector3/30 -> outpmodule/195(VBCM_LBSD_flg)  "<VBCM_LBSD_flg>"
  bus_selector3/29 -> outpmodule/194(VBCM_RDRL_flg)  "<VBCM_RDRL_flg>"
  bus_selector3/26 -> outpmodule/191(VBCM_BrakeLamp_flg)  "<VBCM_BrakeLamp_flg>"
  bus_selector3/25 -> outpmodule/190(VBCM_RrFogLamp_flg)  "<VBCM_RrFogLamp_flg>"
  bus_selector3/24 -> outpmodule/189(VBCM_HBeam_flg)  "<VBCM_HBeam_flg>"
  bus_selector3/18 -> outpmodule/183(VBCM_DoorLockIND_flg)  "<VBCM_DoorLockIND_flg>"
  bus_selector3/22 -> outpmodule/187(VBCM_PosLamp_flg)  "<VBCM_PosLamp_flg>"
  bus_selector3/23 -> outpmodule/188(VBCM_LBeam_flg)  "<VBCM_LBeam_flg>"
  bus_selector3/16 -> outpmodule/181(VBCM_CrashDetd_flg)  "<VBCM_CrashDetd_flg>"
  bus_selector2/133 -> outpmodule/136(VAPM_EPBStaTimeOut_flg)  "<VAPM_EPBStaTimeOut_flg>"
  bus_selector2/61 -> outpmodule/64(VAPM_LFWhlRotDirTimeOut_flg)  "<VAPM_LFWhlRotDirTimeOut_flg>"
  bus_selector2/48 -> outpmodule/51(VAPM_LRRawWhlSpeed_kph)  "<VAPM_LRRawWhlSpeed_kph>"
  bus_selector2/60 -> outpmodule/63(VAPM_LFWhlRotDir_enum)  "<VAPM_LFWhlRotDir_enum>"
  outpmodule/553(VOUTP_FDCTHCPsEVentZSta_enum) -> bus_creator/553
  bus_selector3/53 -> outpmodule/218(VBCM_User3IPAmbLightBrightness_enum)  "<VBCM_User3IPAmbLightBrightness_enum>"
  outpmodule/552(VOUTP_FDCTHCCLEVentZSta_enum) -> bus_creator/552
  outpmodule/548(VOUTP_FDCTHCAirIntZ3Sta_enum) -> bus_creator/548
  outpmodule/549(VOUTP_FDCTHCDrEVentModeSta_enum) -> bus_creator/549
  outpmodule/547(VOUTP_sigDfrstSt_flg) -> bus_creator/547
  outpmodule/546(VOUTP_sigSetTempZon2StM_C) -> bus_creator/546
  outpmodule/544(VOUTP_AirIntenZone1M_enum) -> bus_creator/544
  outpmodule/542(VOUTP_ACForceOFF_flg) -> bus_creator/542
  outpmodule/539(VOUTP_FaceM_flg) -> bus_creator/539
  outpmodule/537(VOUTP_Foot_flg) -> bus_creator/537
  outpmodule/536(VOUTP_Face_flg) -> bus_creator/536
  outpmodule/535(VOUTP_ACModeMem_enum) -> bus_creator/535
  outpmodule/532(VOUTP_sigCbnAirT_C) -> bus_creator/532
  outpmodule/527(VOUTP_sigClntTHvBattOut_C) -> bus_creator/527
  outpmodule/524(VOUTP_sigRecircSt_flg) -> bus_creator/524
  outpmodule/523(VOUTP_sigWindDirZon1St_enum) -> bus_creator/523
  outpmodule/560(VOUTP_FDCTHCPsVentENSta_flg) -> bus_creator/560
  outpmodule/556(VOUTP_FDCTHCDrVentENSta_flg) -> bus_creator/556
  bus_selector8/42 -> outpmodule/453(VPMM_HWResetSta_enum)  "<VPMM_HWResetSta_enum>"
  bus_selector8/44 -> outpmodule/455(VPMM_PwrStaTOSta_enum)  "<VPMM_PwrStaTOSta_enum>"
  bus_selector8/40 -> outpmodule/451(VPMM_CtrlFrBMSCCUCIR_flg)  "<VPMM_CtrlFrBMSCCUCIR_flg>"
  bus_selector8/38 -> outpmodule/449(VPMM_CtrlFrPwrStbA1P_flg)  "<VPMM_CtrlFrPwrStbA1P_flg>"
  bus_selector8/34 -> outpmodule/445(VPMM_PMMAllowECUSleep_flg)  "<VPMM_PMMAllowECUSleep_flg>"
  bus_selector8/29 -> outpmodule/440(VPMM_LVChrgHoldTtimer_s)  "<VPMM_LVChrgHoldTtimer_s>"
  bus_selector8/21 -> outpmodule/432(VPMM_PwrUpReq_enum)  "<VPMM_PwrUpReq_enum>"
  bus_selector8/18 -> outpmodule/429(VPMM_PwrStaSelect_enum)  "<VPMM_PwrStaSelect_enum>"
  bus_selector3/54 -> outpmodule/219(VBCM_User4DrAmbLightBrightness_enum)  "<VBCM_User4DrAmbLightBrightness_enum>"
  bus_selector8/17 -> outpmodule/428(VPMM_DrSeatSta_enum)  "<VPMM_DrSeatSta_enum>"
  BPMM_outputs/1 -> bus_selector8/1
  bus_selector8/10 -> outpmodule/421(VPMM_PowerSta_enum)  "<VPMM_PowerSta_enum>"
  bus_selector8/11 -> outpmodule/422(VPMM_LVPwrSta_flg)  "<VPMM_LVPwrSta_flg>"
  outpmodule/399(VOUTP_DKCAuthSta_enum) -> bus_creator/399
  outpmodule/395(VOUTP_ActAPSPosn_pct) -> bus_creator/395
  bus_selector8/33 -> outpmodule/444(VPMM_FDADC12VDetAvg_mV)  "<VPMM_FDADC12VDetAvg_mV>"
  outpmodule/525(VOUTP_sigSetTempZon1St_C) -> bus_creator/525
  outpmodule/396(VOUTP_EAPS1MIN_pct) -> bus_creator/396
  bus_selector8/28 -> outpmodule/439(VPMM_IVIPwrStaONTOPopT_s)  "<VPMM_IVIPwrStaONTOPopT_s>"
  outpmodule/394(VOUTP_EDriveSysErr_VCUErrTmp_flg) -> bus_creator/394
  outpmodule/411(VOUTP_NetworkReq_flg) -> bus_creator/411
  outpmodule/231(VOUTP_AmbLightBreath1_flg) -> bus_creator/231
  outpmodule/228(VOUTP_User4AmbLightColor_enum) -> bus_creator/228
  outpmodule/264(VOUTP_C3BMS6LCDTC_raw32) -> bus_creator/264
  outpmodule/227(VOUTP_User3AmbLightColor_enum) -> bus_creator/227
  bus_selector3/21 -> outpmodule/186(VBCM_DimmerEN_flg)  "<VBCM_DimmerEN_flg>"
  outpmodule/226(VOUTP_User2AmbLightColor_enum) -> bus_creator/226
  bus_selector3/6 -> outpmodule/171(VBCM_AntitheftSeatFlod_flg)  "<VBCM_AntitheftSeatFlod_flg>"
  outpmodule/224(VOUTP_User6IPAmbLightBrightness_enum) -> bus_creator/224
  bus_selector3/56 -> outpmodule/221(VBCM_User5DrAmbLightBrightness_enum)  "<VBCM_User5DrAmbLightBrightness_enum>"
  outpmodule/223(VOUTP_User6DrAmbLightBrightness_enum) -> bus_creator/223
  outpmodule/225(VOUTP_User1AmbLightColor_enum) -> bus_creator/225
  bus_selector2/56 -> outpmodule/59(VAPM_LRRawWhlSpeedV_flg)  "<VAPM_LRRawWhlSpeedV_flg>"
  bus_selector2/95 -> outpmodule/98(VAPM_SASSpeedValidTimeOut_flg)  "<VAPM_SASSpeedValidTimeOut_flg>"
  bus_selector14/2 -> outpmodule/721(VV2L_ReqV2LIVIPopup_enum)  "<VV2L_ReqV2LIVIPopup_enum>"
  bus_selector14/1 -> outpmodule/720(VV2L_ReqOBCV2LEna_enum)  "<VV2L_ReqOBCV2LEna_enum>"
  bus_selector2/110 -> outpmodule/113(VAPM_YawRateV_flg)  "<VAPM_YawRateV_flg>"
  bus_selector2/109 -> outpmodule/112(VAPM_MCPressureTimeOut_flg)  "<VAPM_MCPressureTimeOut_flg>"
  bus_selector2/121 -> outpmodule/124(VAPM_BrkSwVTimeOut_flg)  "<VAPM_BrkSwVTimeOut_flg>"
  bus_selector2/106 -> outpmodule/109(VAPM_LongAccel_Gps)  "<VAPM_LongAccel_Gps>"
  bus_selector2/108 -> outpmodule/111(VAPM_MCPressure_bar)  "<VAPM_MCPressure_bar>"
  bus_selector2/115 -> outpmodule/118(VAPM_LongAccelVTimeOut_flg)  "<VAPM_LongAccelVTimeOut_flg>"
  bus_selector2/111 -> outpmodule/114(VAPM_YawRateVTimeOut_flg)  "<VAPM_YawRateVTimeOut_flg>"
  bus_selector2/113 -> outpmodule/116(VAPM_LatAccelVTimeOut_flg)  "<VAPM_LatAccelVTimeOut_flg>"
  outpmodule/245(VOUTP_CountAlarm_enum) -> bus_creator/245
  bus_selector11/67 -> outpmodule/643(VTPM_TPMSStorge_flg)  "<VTPM_TPMSStorge_flg>"
  bus_selector2/131 -> outpmodule/134(VAPM_EPBErrStaTimeOut_flg)  "<VAPM_EPBErrStaTimeOut_flg>"
  bus_selector2/129 -> outpmodule/132(VAPM_EPBExtApplyAvailTimeOut_flg)  "<VAPM_EPBExtApplyAvailTimeOut_flg>"
  bus_selector2/159 -> outpmodule/162(VAPM_APSAngleTarget_Deg)  "<VAPM_APSAngleTarget_Deg>"
  bus_selector2/154 -> outpmodule/157(VAPM_APSProgressPCT_pct)  "<VAPM_APSProgressPCT_pct>"
  bus_selector3/79 -> outpmodule/244(VBCM_IVIRST_flg)  "<VBCM_IVIRST_flg>"
  bus_selector3/78 -> outpmodule/243(VBCM_FollowMe_flg)  "<VBCM_FollowMe_flg>"
  bus_selector3/77 -> outpmodule/242(VBCM_APSOpenPTG_flg)  "<VBCM_APSOpenPTG_flg>"
  outpmodule/543(VOUTP_RecAutoFlg_flg) -> bus_creator/543
  bus_selector3/76 -> outpmodule/241(VBCM_SPTGDet_flg)  "<VBCM_SPTGDet_flg>"
  bus_selector3/75 -> outpmodule/240(VBCM_LampPwr_flg)  "<VBCM_LampPwr_flg>"
  bus_selector2/160 -> outpmodule/163(VAPM_APSVRqEPASCtrl_flg)  "<VAPM_APSVRqEPASCtrl_flg>"
  bus_selector4/21 -> outpmodule/282(VDDM_BrkSWNoBacDTC_raw32)  "<VDDM_BrkSWNoBacDTC_raw32>"
  bus_selector4/17 -> outpmodule/278(VDDM_Lv2ErrDTC_raw32)  "<VDDM_Lv2ErrDTC_raw32>"
  bus_selector4/19 -> outpmodule/280(VDDM_Lv4ErrDTC_raw32)  "<VDDM_Lv4ErrDTC_raw32>"
  bus_selector4/25 -> outpmodule/286(VDDM_MCU4PreDTC_raw32)  "<VDDM_MCU4PreDTC_raw32>"
  bus_selector8/20 -> outpmodule/431(VPMM_TCountSta_enum)  "<VPMM_TCountSta_enum>"
  bus_selector4/22 -> outpmodule/283(VDDM_KeyAuthDTC_raw32)  "<VDDM_KeyAuthDTC_raw32>"
  bus_selector2/45 -> outpmodule/48(VAPM_LFRawWhlSpeedTimeOut_flg)  "<VAPM_LFRawWhlSpeedTimeOut_flg>"
  bus_selector2/101 -> outpmodule/104(VAPM_GRADETimeOut_flg)  "<VAPM_GRADETimeOut_flg>"
  bus_selector2/91 -> outpmodule/94(VAPM_SASAngleTimeOut_flg)  "<VAPM_SASAngleTimeOut_flg>"
  bus_selector2/93 -> outpmodule/96(VAPM_SASSpeedTimeOut_flg)  "<VAPM_SASSpeedTimeOut_flg>"
  bus_selector2/86 -> outpmodule/89(VAPM_DriIntend_enum)  "<VAPM_DriIntend_enum>"
  bus_selector2/89 -> outpmodule/92(VAPM_EPSAOIControlTimeOut_flg)  "<VAPM_EPSAOIControlTimeOut_flg>"
  bus_selector2/84 -> outpmodule/87(VAPM_ShifterHandleCmd_enum)  "<VAPM_ShifterHandleCmd_enum>"
  bus_selector2/80 -> outpmodule/83(VAPM_LRPulseCount_enum)  "<VAPM_LRPulseCount_enum>"
  bus_selector2/75 -> outpmodule/78(VAPM_RRPulseCountVTimeOut_flg)  "<VAPM_RRPulseCountVTimeOut_flg>"
  bus_selector2/78 -> outpmodule/81(VAPM_RFPulseCount_enum)  "<VAPM_RFPulseCount_enum>"
  bus_selector2/77 -> outpmodule/80(VAPM_LFPulseCountTimeOut_flg)  "<VAPM_LFPulseCountTimeOut_flg>"
  bus_selector2/76 -> outpmodule/79(VAPM_LFPulseCount_enum)  "<VAPM_LFPulseCount_enum>"
  bus_selector2/72 -> outpmodule/75(VAPM_LRPulseCountV_flg)  "<VAPM_LRPulseCountV_flg>"
  bus_selector2/71 -> outpmodule/74(VAPM_RFPulseCountVTimeOut_flg)  "<VAPM_RFPulseCountVTimeOut_flg>"
  outpmodule/529(VOUTP_sigClntTHvBattIn_C) -> bus_creator/529
  bus_selector2/70 -> outpmodule/73(VAPM_RFPulseCountV_flg)  "<VAPM_RFPulseCountV_flg>"
  bus_selector2/69 -> outpmodule/72(VAPM_LFPulseCountVTimeOut_flg)  "<VAPM_LFPulseCountVTimeOut_flg>"
  bus_selector2/67 -> outpmodule/70(VAPM_RRWhlRotDirTimeOut_flg)  "<VAPM_RRWhlRotDirTimeOut_flg>"
  bus_selector2/68 -> outpmodule/71(VAPM_LFPulseCountV_flg)  "<VAPM_LFPulseCountV_flg>"
  bus_selector2/64 -> outpmodule/67(VAPM_LRWhlRotDir_enum)  "<VAPM_LRWhlRotDir_enum>"
  bus_selector10/63 -> outpmodule/558(VTHC_FDCTHCCLVentENSta_flg)  "<VTHC_FDCTHCCLVentENSta_flg>"
  bus_selector10/62 -> outpmodule/557(VTHC_FDCTHCCLEVentYSta_enum)  "<VTHC_FDCTHCCLEVentYSta_enum>"
  bus_selector10/59 -> outpmodule/554(VTHC_FDCTHCCREVentZSta_enum)  "<VTHC_FDCTHCCREVentZSta_enum>"
  bus_selector10/61 -> outpmodule/556(VTHC_FDCTHCDrVentENSta_flg)  "<VTHC_FDCTHCDrVentENSta_flg>"
  bus_selector10/55 -> outpmodule/550(VTHC_FDCTHCPsEVentModeSta_enum)  "<VTHC_FDCTHCPsEVentModeSta_enum>"
  bus_selector10/56 -> outpmodule/551(VTHC_FDCTHCDrEVentZSta_enum)  "<VTHC_FDCTHCDrEVentZSta_enum>"
  outpmodule/562(VOUTP_FDCTHCCRVentENSta_flg) -> bus_creator/562
  bus_selector10/57 -> outpmodule/552(VTHC_FDCTHCCLEVentZSta_enum)  "<VTHC_FDCTHCCLEVentZSta_enum>"
  bus_selector10/51 -> outpmodule/546(VTHC_sigSetTempZon2StM_C)  "<VTHC_sigSetTempZon2StM_C>"
  bus_selector10/54 -> outpmodule/549(VTHC_FDCTHCDrEVentModeSta_enum)  "<VTHC_FDCTHCDrEVentModeSta_enum>"
  bus_selector8/45 -> outpmodule/456(VPMM_Sched_ChgTOSta_enum)  "<VPMM_Sched_ChgTOSta_enum>"
  bus_selector10/53 -> outpmodule/548(VTHC_FDCTHCAirIntZ3Sta_enum)  "<VTHC_FDCTHCAirIntZ3Sta_enum>"
  bus_selector10/50 -> outpmodule/545(VTHC_fdefog_flg)  "<VTHC_fdefog_flg>"
  bus_selector10/46 -> outpmodule/541(VTHC_CCUSyncSts_flg)  "<VTHC_CCUSyncSts_flg>"
  bus_selector10/48 -> outpmodule/543(VTHC_RecAutoFlg_flg)  "<VTHC_RecAutoFlg_flg>"
  bus_selector10/45 -> outpmodule/540(VTHC_FootM_flg)  "<VTHC_FootM_flg>"
  outpmodule/271(VOUTP_C3CCU2RCDTC_raw32) -> bus_creator/271
  bus_selector10/42 -> outpmodule/537(VTHC_Foot_flg)  "<VTHC_Foot_flg>"
  bus_selector10/43 -> outpmodule/538(VTHC_Frost_flg)  "<VTHC_Frost_flg>"
  bus_selector10/40 -> outpmodule/535(VTHC_ACModeMem_enum)  "<VTHC_ACModeMem_enum>"
  bus_selector10/41 -> outpmodule/536(VTHC_Face_flg)  "<VTHC_Face_flg>"
  outpmodule/248(VOUTP_FuelDoorPos_flg) -> bus_creator/248
  bus_selector10/36 -> outpmodule/531(VTHC_sigAmbAirT_C)  "<VTHC_sigAmbAirT_C>"
  bus_selector10/35 -> outpmodule/530(VTHC_sigCbnSolarRight_W)  "<VTHC_sigCbnSolarRight_W>"
  bus_selector10/37 -> outpmodule/532(VTHC_sigCbnAirT_C)  "<VTHC_sigCbnAirT_C>"
  bus_selector10/38 -> outpmodule/533(VTHC_ACSubMode_enum)  "<VTHC_ACSubMode_enum>"
  bus_selector2/81 -> outpmodule/84(VAPM_LRPulseCountTimeOut_flg)  "<VAPM_LRPulseCountTimeOut_flg>"
  bus_selector10/32 -> outpmodule/527(VTHC_sigClntTHvBattOut_C)  "<VTHC_sigClntTHvBattOut_C>"
  bus_selector10/33 -> outpmodule/528(VTHC_sigCbnSolarLeft_W)  "<VTHC_sigCbnSolarLeft_W>"
  bus_selector10/30 -> outpmodule/525(VTHC_sigSetTempZon1St_C)  "<VTHC_sigSetTempZon1St_C>"
  bus_selector10/28 -> outpmodule/523(VTHC_sigWindDirZon1St_enum)  "<VTHC_sigWindDirZon1St_enum>"
  bus_selector10/29 -> outpmodule/524(VTHC_sigRecircSt_flg)  "<VTHC_sigRecircSt_flg>"
  bus_selector10/27 -> outpmodule/522(VTHC_sigAirIntenZon1St_enum)  "<VTHC_sigAirIntenZon1St_enum>"
  bus_selector10/24 -> outpmodule/519(VTHC_CCUAutoLampSts_flg)  "<VTHC_CCUAutoLampSts_flg>"
  bus_selector10/25 -> outpmodule/520(VTHC_CCUACMaxLampSts_flg)  "<VTHC_CCUACMaxLampSts_flg>"
  bus_selector10/20 -> outpmodule/515(VTHC_BatteryMode_enum)  "<VTHC_BatteryMode_enum>"
  bus_selector10/21 -> outpmodule/516(VTHC_EDriveMode_enum)  "<VTHC_EDriveMode_enum>"
  outpmodule/402(VOUTP_Awake_enum) -> bus_creator/402
  bus_selector10/22 -> outpmodule/517(VTHC_CabinMode_enum)  "<VTHC_CabinMode_enum>"
  bus_selector10/19 -> outpmodule/514(VTHC_FDBlowerCmd_pct)  "<VTHC_FDBlowerCmd_pct>"
  bus_selector10/17 -> outpmodule/512(VTHC_FDFrRiAPTCHeatPwrCmd_W)  "<VTHC_FDFrRiAPTCHeatPwrCmd_W>"
  bus_selector10/18 -> outpmodule/513(VTHC_FDRrAPTCHeatPwrCmd_W)  "<VTHC_FDRrAPTCHeatPwrCmd_W>"
  outpmodule/250(VOUTP_RoomLampMode_flg) -> bus_creator/250
  bus_selector10/14 -> outpmodule/509(VTHC_FDEWP2Cmd_enum)  "<VTHC_FDEWP2Cmd_enum>"
  bus_selector10/15 -> outpmodule/510(VTHC_FDEWP3Cmd_enum)  "<VTHC_FDEWP3Cmd_enum>"
  bus_selector10/13 -> outpmodule/508(VTHC_FDEWP1Cmd_enum)  "<VTHC_FDEWP1Cmd_enum>"
  bus_selector10/16 -> outpmodule/511(VTHC_FDFrLeAPTCHeatPwrCmd_W)  "<VTHC_FDFrLeAPTCHeatPwrCmd_W>"
  bus_selector10/11 -> outpmodule/506(VTHC_CoolgFanActDuty_pct)  "<VTHC_CoolgFanActDuty_pct>"
  bus_selector10/12 -> outpmodule/507(VTHC_FDAGSCmd_enum)  "<VTHC_FDAGSCmd_enum>"
  bus_selector10/10 -> outpmodule/505(VTHC_FDFrWPTCHeatPwrCmd_W)  "<VTHC_FDFrWPTCHeatPwrCmd_W>"
  bus_selector4/18 -> outpmodule/279(VDDM_Lv3ErrDTC_raw32)  "<VDDM_Lv3ErrDTC_raw32>"
  bus_selector10/8 -> outpmodule/503(VTHC_FDFWVCmd_flg)  "<VTHC_FDFWVCmd_flg>"
  bus_selector10/6 -> outpmodule/501(VTHC_FDEXV2Cmd_step)  "<VTHC_FDEXV2Cmd_step>"
  bus_selector10/7 -> outpmodule/502(VTHC_FDSOTXVCmd_flg)  "<VTHC_FDSOTXVCmd_flg>"
  bus_selector10/2 -> outpmodule/497(VTHC_FDSOV1Cmd_flg)  "<VTHC_FDSOV1Cmd_flg>"
  bus_selector10/3 -> outpmodule/498(VTHC_FDSOV2Cmd_flg)  "<VTHC_FDSOV2Cmd_flg>"
  bus_selector10/4 -> outpmodule/499(VTHC_FDSOV3Cmd_flg)  "<VTHC_FDSOV3Cmd_flg>"
  bus_selector11/64 -> outpmodule/640(VTPM_ID4messageALTU_raw8)  "<VTPM_ID4messageALTU_raw8>"
  outpmodule/254(VOUTP_LPasCtrlCmd_pct) -> bus_creator/254
  BTHC_outputs/1 -> bus_selector10/1
  bus_selector10/81 -> outpmodule/576(VTHC_FDCTHCMPreWPTCHeatSta_enum)  "<VTHC_FDCTHCMPreWPTCHeatSta_enum>"
  bus_selector10/80 -> outpmodule/575(VTHC_FDCFGSLearnCmd_enum)  "<VTHC_FDCFGSLearnCmd_enum>"
  outpmodule/554(VOUTP_FDCTHCCREVentZSta_enum) -> bus_creator/554
  bus_selector10/77 -> outpmodule/572(VTHC_FDCFGSChCmd_enum)  "<VTHC_FDCFGSChCmd_enum>"
  bus_selector10/75 -> outpmodule/570(VTHC_FDCFGSAirIntCmd_enum)  "<VTHC_FDCFGSAirIntCmd_enum>"
  bus_selector10/73 -> outpmodule/568(VTHC_FDCFGSAirIntSta_enum)  "<VTHC_FDCFGSAirIntSta_enum>"
  bus_selector10/70 -> outpmodule/565(VTHC_CLVentEN_flg)  "<VTHC_CLVentEN_flg>"
  bus_selector10/69 -> outpmodule/564(VTHC_DrVentEN_flg)  "<VTHC_DrVentEN_flg>"
  bus_selector10/67 -> outpmodule/562(VTHC_FDCTHCCRVentENSta_flg)  "<VTHC_FDCTHCCRVentENSta_flg>"
  bus_selector10/66 -> outpmodule/561(VTHC_FDCTHCCREVentYSta_enum)  "<VTHC_FDCTHCCREVentYSta_enum>"
  bus_selector2/87 -> outpmodule/90(VAPM_DriIntendTimeOut_flg)  "<VAPM_DriIntendTimeOut_flg>"
  bus_selector8/22 -> outpmodule/433(VPMM_PwrDownReq_enum)  "<VPMM_PwrDownReq_enum>"
  bus_selector10/65 -> outpmodule/560(VTHC_FDCTHCPsVentENSta_flg)  "<VTHC_FDCTHCPsVentENSta_flg>"
  bus_selector4/89 -> outpmodule/350(VDDM_RrMCUSigErrDetDTC_raw32)  "<VDDM_RrMCUSigErrDetDTC_raw32>"
  bus_selector10/39 -> outpmodule/534(VTHC_FDRecyAutoCmd_enum)  "<VTHC_FDRecyAutoCmd_enum>"
  bus_selector4/86 -> outpmodule/347(VDDM_BMSSigErrDetDTC_raw32)  "<VDDM_BMSSigErrDetDTC_raw32>"
  bus_selector4/84 -> outpmodule/345(VDDM_FCM5CSErrDTC_raw32)  "<VDDM_FCM5CSErrDTC_raw32>"
  bus_selector4/85 -> outpmodule/346(VDDM_ZoneSCPNoComDTC_raw32)  "<VDDM_ZoneSCPNoComDTC_raw32>"
  bus_selector4/83 -> outpmodule/344(VDDM_FCM5NoComDTC_raw32)  "<VDDM_FCM5NoComDTC_raw32>"
  bus_selector4/79 -> outpmodule/340(VDDM_FCM3RCErrDTC_raw32)  "<VDDM_FCM3RCErrDTC_raw32>"
  bus_selector4/77 -> outpmodule/338(VDDM_FCM2CSErrDTC_raw32)  "<VDDM_FCM2CSErrDTC_raw32>"
  bus_selector4/78 -> outpmodule/339(VDDM_FCM3NoComDTC_raw32)  "<VDDM_FCM3NoComDTC_raw32>"
  bus_selector4/75 -> outpmodule/336(VDDM_FCM2NoComDTC_raw32)  "<VDDM_FCM2NoComDTC_raw32>"
  bus_selector4/74 -> outpmodule/335(VDDM_RLRUSSDTC_raw32)  "<VDDM_RLRUSSDTC_raw32>"
  bus_selector4/73 -> outpmodule/334(VDDM_RLLUSSDTC_raw32)  "<VDDM_RLLUSSDTC_raw32>"
  bus_selector8/24 -> outpmodule/435(VPMM_ReVehThdChkSta_enum)  "<VPMM_ReVehThdChkSta_enum>"
  bus_selector4/70 -> outpmodule/331(VDDM_RCRUSSDTC_raw32)  "<VDDM_RCRUSSDTC_raw32>"
  bus_selector4/68 -> outpmodule/329(VDDM_RMLUSSDTC_raw32)  "<VDDM_RMLUSSDTC_raw32>"
  bus_selector10/71 -> outpmodule/566(VTHC_PsVentEN_flg)  "<VTHC_PsVentEN_flg>"
  bus_selector4/66 -> outpmodule/327(VDDM_FCRUSSDTC_raw32)  "<VDDM_FCRUSSDTC_raw32>"
  bus_selector4/109 -> outpmodule/370(VDDM_RrMCUTqErrDTC_raw32)  "<VDDM_RrMCUTqErrDTC_raw32>"
  bus_selector4/110 -> outpmodule/371(VDDM_LFBatwarnDTC_raw32)  "<VDDM_LFBatwarnDTC_raw32>"
  bus_selector4/108 -> outpmodule/369(VDDM_FrMCUTqErrDTC_raw32)  "<VDDM_FrMCUTqErrDTC_raw32>"
  bus_selector10/44 -> outpmodule/539(VTHC_FaceM_flg)  "<VTHC_FaceM_flg>"
  bus_selector4/106 -> outpmodule/367(VDDM_ESC5RCErrDTC_raw32)  "<VDDM_ESC5RCErrDTC_raw32>"
  bus_selector10/49 -> outpmodule/544(VTHC_AirIntenZone1M_enum)  "<VTHC_AirIntenZone1M_enum>"
  bus_selector4/107 -> outpmodule/368(VDDM_ESC5CSErrDTC_raw32)  "<VDDM_ESC5CSErrDTC_raw32>"
  bus_selector4/105 -> outpmodule/366(VDDM_ESC1CSErrDTC_raw32)  "<VDDM_ESC1CSErrDTC_raw32>"
  bus_selector4/104 -> outpmodule/365(VDDM_ESC1RCErrDTC_raw32)  "<VDDM_ESC1RCErrDTC_raw32>"
  bus_selector4/103 -> outpmodule/364(VDDM_ESC7CSErrDTC_raw32)  "<VDDM_ESC7CSErrDTC_raw32>"
  bus_selector4/102 -> outpmodule/363(VDDM_ESC7RCErrDTC_raw32)  "<VDDM_ESC7RCErrDTC_raw32>"
  bus_selector4/101 -> outpmodule/362(VDDM_Shifter1CSErrDTC_raw32)  "<VDDM_Shifter1CSErrDTC_raw32>"
  bus_selector4/94 -> outpmodule/355(VDDM_MSAMalfuncDetDTC_raw32)  "<VDDM_MSAMalfuncDetDTC_raw32>"
  bus_selector4/96 -> outpmodule/357(VDDM_MCUF1RCErrDTC_raw32)  "<VDDM_MCUF1RCErrDTC_raw32>"
  bus_selector4/97 -> outpmodule/358(VDDM_MCUR1RCErrDTC_raw32)  "<VDDM_MCUR1RCErrDTC_raw32>"
  bus_selector4/98 -> outpmodule/359(VDDM_MCUF1CSErrDTC_raw32)  "<VDDM_MCUF1CSErrDTC_raw32>"
  outpmodule/247(VOUTP_MirrorFlodPos_flg) -> bus_creator/247
  bus_selector2/36 -> outpmodule/39(VAPM_USSStaFCR_flg)  "<VAPM_USSStaFCR_flg>"
  outpmodule/278(VOUTP_Lv2ErrDTC_raw32) -> bus_creator/278
  bus_selector2/34 -> outpmodule/37(VAPM_USSStaFLR_flg)  "<VAPM_USSStaFLR_flg>"
  bus_selector2/114 -> outpmodule/117(VAPM_LongAccelV_flg)  "<VAPM_LongAccelV_flg>"
  bus_selector2/104 -> outpmodule/107(VAPM_LatAccel_Gps)  "<VAPM_LatAccel_Gps>"
  bus_selector8/37 -> outpmodule/448(VPMM_LVSilentChrgLv_enum)  "<VPMM_LVSilentChrgLv_enum>"
  bus_selector2/59 -> outpmodule/62(VAPM_RRRawWhlSpeedVTimeOut_flg)  "<VAPM_RRRawWhlSpeedVTimeOut_flg>"
  outpmodule/550(VOUTP_FDCTHCPsEVentModeSta_enum) -> bus_creator/550
  bus_selector2/58 -> outpmodule/61(VAPM_RRRawWhlSpeedV_flg)  "<VAPM_RRRawWhlSpeedV_flg>"
  bus_selector2/51 -> outpmodule/54(VAPM_RRRawWhlSpeedTimeOut_flg)  "<VAPM_RRRawWhlSpeedTimeOut_flg>"
  bus_selector2/9 -> outpmodule/12(VAPM_PASDRCL_cm)  "<VAPM_PASDRCL_cm>"
  bus_selector2/8 -> outpmodule/11(VAPM_PASDRCR_cm)  "<VAPM_PASDRCR_cm>"
  outpmodule/522(VOUTP_sigAirIntenZon1St_enum) -> bus_creator/522
  bus_selector2/7 -> outpmodule/10(VAPM_PASDRML_cm)  "<VAPM_PASDRML_cm>"
  bus_selector2/4 -> outpmodule/7(VAPM_FSOffSwTimeOut_flg)  "<VAPM_FSOffSwTimeOut_flg>"
  bus_selector2/6 -> outpmodule/9(VAPM_PASDRMR_cm)  "<VAPM_PASDRMR_cm>"
  bus_selector10/1 -> outpmodule/496(VTHC_FDCompCmd_rpm)  "<VTHC_FDCompCmd_rpm>"
  bus_selector2/3 -> outpmodule/6(VAPM_FSOffSw_enum)  "<VAPM_FSOffSw_enum>"
  BACC_outputs/1 -> bus_selector1/1
  bus_selector1/2 -> outpmodule/2(VACC_LVBattVoltSta_enum)  "<VACC_LVBattVoltSta_enum>"
  bus_selector2/21 -> outpmodule/24(VAPM_PASARCR_enum)  "<VAPM_PASARCR_enum>"
  bus_selector2/16 -> outpmodule/19(VAPM_APSDFLR_cm)  "<VAPM_APSDFLR_cm>"
  bus_selector2/15 -> outpmodule/18(VAPM_APSDRLL_cm)  "<VAPM_APSDRLL_cm>"
  outpmodule/222(VOUTP_User5IPAmbLightBrightness_enum) -> bus_creator/222
  bus_selector8/46 -> outpmodule/457(VPMM_PwrReq_OTA_enum)  "<VPMM_PwrReq_OTA_enum>"
  bus_selector2/12 -> outpmodule/15(VAPM_PASDFCR_cm)  "<VAPM_PASDFCR_cm>"
  bus_selector9/34 -> outpmodule/493(VSYS_WisrBootReason_raw32)  "<VSYS_WisrBootReason_raw32>"
  bus_selector9/29 -> outpmodule/488(VSYS_SHA8_cnt)  "<VSYS_SHA8_cnt>"
  bus_selector9/26 -> outpmodule/485(VSYS_SHA5_cnt)  "<VSYS_SHA5_cnt>"
  bus_selector9/20 -> outpmodule/479(VSYS_Change2_cnt)  "<VSYS_Change2_cnt>"
  bus_selector9/21 -> outpmodule/480(VSYS_Dash2_cnt)  "<VSYS_Dash2_cnt>"
  bus_selector9/13 -> outpmodule/472(VSYS_Patch1_cnt)  "<VSYS_Patch1_cnt>"
  bus_selector9/12 -> outpmodule/471(VSYS_Minor2_cnt)  "<VSYS_Minor2_cnt>"
  bus_selector10/9 -> outpmodule/504(VTHC_FDTWVCmd_pct)  "<VTHC_FDTWVCmd_pct>"
  bus_selector9/6 -> outpmodule/465(VSYS_CarModel3_cnt)  "<VSYS_CarModel3_cnt>"
  bus_selector9/2 -> outpmodule/461(VSYS_HWVer2_cnt)  "<VSYS_HWVer2_cnt>"
  outpmodule/392(VOUTP_THCMAPTCWarning_raw32) -> bus_creator/392
  outpmodule/674(VOUTP_ParkRequest_flg) -> bus_creator/674
  outpmodule/673(VOUTP_ModelVersionChksum_raw) -> bus_creator/673
  outpmodule/670(VOUTP_LProgress_enum) -> bus_creator/670
  outpmodule/666(VOUTP_FlashS4ID_raw) -> bus_creator/666
  bus_selector8/30 -> outpmodule/441(VPMM_LVBattChrgTimeCnt_s)  "<VPMM_LVBattChrgTimeCnt_s>"
  outpmodule/668(VOUTP_WritingCnt_enum) -> bus_creator/668
  outpmodule/667(VOUTP_FlashIDvalid_enum) -> bus_creator/667
  outpmodule/661(VOUTP_unlearnSfailvalid_enum) -> bus_creator/661
  bus_selector4/99 -> outpmodule/360(VDDM_MCUR1CSErrDTC_raw32)  "<VDDM_MCUR1CSErrDTC_raw32>"
  bus_selector10/79 -> outpmodule/574(VTHC_FDCFGSIONCmd_flg)  "<VTHC_FDCFGSIONCmd_flg>"
  outpmodule/659(VOUTP_Flashdatavalid_enum) -> bus_creator/659
  bus_selector2/88 -> outpmodule/91(VAPM_EPSAOIControl_enum)  "<VAPM_EPSAOIControl_enum>"
  bus_selector9/30 -> outpmodule/489(VSYS_NvWriteReqRisingEdge_flg)  "<VSYS_NvWriteReqRisingEdge_flg>"
  outpmodule/660(VOUTP_unlearnSfali_flg) -> bus_creator/660
  outpmodule/656(VOUTP_WriteChkfinLRID_raw) -> bus_creator/656
  bus_selector4/20 -> outpmodule/281(VDDM_BrkSWErrDTC_raw32)  "<VDDM_BrkSWErrDTC_raw32>"
  outpmodule/649(VOUTP_RRPindi_enum) -> bus_creator/649
  bus_selector2/85 -> outpmodule/88(VAPM_ShifterHandleCmdTimeOut_flg)  "<VAPM_ShifterHandleCmdTimeOut_flg>"
  outpmodule/647(VOUTP_RFPind_enum) -> bus_creator/647
  outpmodule/645(VOUTP_TPMSResButt_flg) -> bus_creator/645
  outpmodule/643(VOUTP_TPMSStorge_flg) -> bus_creator/643
  outpmodule/277(VOUTP_Lv1ErrDTC_raw32) -> bus_creator/277
  bus_selector9/15 -> outpmodule/474(VSYS_Country1_cnt)  "<VSYS_Country1_cnt>"
  outpmodule/644(VOUTP_ChkStorge_flg) -> bus_creator/644
  outpmodule/679(VOUTP_EVDriveMode_enum) -> bus_creator/679
  bus_selector2/132 -> outpmodule/135(VAPM_EPBSta_enum)  "<VAPM_EPBSta_enum>"
  bus_selector2/30 -> outpmodule/33(VAPM_USSStaRCR_flg)  "<VAPM_USSStaRCR_flg>"
  outpmodule/347(VOUTP_BMSSigErrDetDTC_raw32) -> bus_creator/347
  outpmodule/348(VOUTP_FCMACCSigErrDetDTC_raw32) -> bus_creator/348
  outpmodule/343(VOUTP_FCM4CSErrDTC_raw32) -> bus_creator/343
  bus_selector3/57 -> outpmodule/222(VBCM_User5IPAmbLightBrightness_enum)  "<VBCM_User5IPAmbLightBrightness_enum>"
  outpmodule/342(VOUTP_FCM4NoComDTC_raw32) -> bus_creator/342
  outpmodule/341(VOUTP_FCM3CSErrDTC_raw32) -> bus_creator/341
  outpmodule/335(VOUTP_RLRUSSDTC_raw32) -> bus_creator/335
  outpmodule/336(VOUTP_FCM2NoComDTC_raw32) -> bus_creator/336
  outpmodule/332(VOUTP_FLLUSSDTC_raw32) -> bus_creator/332
  outpmodule/331(VOUTP_RCRUSSDTC_raw32) -> bus_creator/331
  outpmodule/329(VOUTP_RMLUSSDTC_raw32) -> bus_creator/329
  outpmodule/328(VOUTP_RCLUSSDTC_raw32) -> bus_creator/328
  outpmodule/325(VOUTP_FMLUSSDTC_raw32) -> bus_creator/325
  outpmodule/326(VOUTP_FMRUSSDTC_raw32) -> bus_creator/326
  outpmodule/321(VOUTP_DiagFRTSDTC_raw32) -> bus_creator/321
  bus_selector2/79 -> outpmodule/82(VAPM_RFPulseCountTimeOut_flg)  "<VAPM_RFPulseCountTimeOut_flg>"
  outpmodule/318(VOUTP_EnterNewOperCyc_flg) -> bus_creator/318
  outpmodule/320(VOUTP_DiagFLTSDTC_raw32) -> bus_creator/320
  outpmodule/319(VOUTP_DiagHCrashDTC_raw32) -> bus_creator/319
  outpmodule/316(VOUTP_ESC1NoComDTC_raw32) -> bus_creator/316
  outpmodule/314(VOUTP_Shifter1NoComDTC_raw32) -> bus_creator/314
  outpmodule/304(VOUTP_FRDoorSWDTC_raw32) -> bus_creator/304
  bus_selector3/27 -> outpmodule/192(VBCM_ReverseLamp_flg)  "<VBCM_ReverseLamp_flg>"
  outpmodule/297(VOUTP_OBC4PreDTC_raw32) -> bus_creator/297
  outpmodule/296(VOUTP_MCUActDTC_raw32) -> bus_creator/296
  outpmodule/291(VOUTP_HiLvSaChkDTC_raw32) -> bus_creator/291
  bus_selector8/35 -> outpmodule/446(VPMM_LVSilentChrgSta_enum)  "<VPMM_LVSilentChrgSta_enum>"
  outpmodule/293(VOUTP_MCUDisDTC_raw32) -> bus_creator/293
  outpmodule/292(VOUTP_MidLvSaChkDTC_raw32) -> bus_creator/292
  bus_selector2/65 -> outpmodule/68(VAPM_LRWhlRotDirTimeOut_flg)  "<VAPM_LRWhlRotDirTimeOut_flg>"
  outpmodule/284(VOUTP_ONtoRdyDTC_raw32) -> bus_creator/284
  outpmodule/282(VOUTP_BrkSWNoBacDTC_raw32) -> bus_creator/282
  outpmodule/658(VOUTP_Flashchkdatavalid_enum) -> bus_creator/658
  outpmodule/413(VOUTP_PowerDownState_enum) -> bus_creator/413
  bus_selector10/26 -> outpmodule/521(VTHC_CCUSyncLampSts_flg)  "<VTHC_CCUSyncLampSts_flg>"
  outpmodule/280(VOUTP_Lv4ErrDTC_raw32) -> bus_creator/280
  outpmodule/221(VOUTP_User5DrAmbLightBrightness_enum) -> bus_creator/221
  outpmodule/281(VOUTP_BrkSWErrDTC_raw32) -> bus_creator/281
  outpmodule/409(VOUTP_ActiveWU_flg) -> bus_creator/409
  outpmodule/355(VOUTP_MSAMalfuncDetDTC_raw32) -> bus_creator/355
  outpmodule/285(VOUTP_HVB4PreDTC_raw32) -> bus_creator/285
  bus_selector4/24 -> outpmodule/285(VDDM_HVB4PreDTC_raw32)  "<VDDM_HVB4PreDTC_raw32>"
  outpmodule/354(VOUTP_CCMalfuncDetDTC_raw32) -> bus_creator/354
  outpmodule/352(VOUTP_ACCAccelCmdErrDetDTC_raw32) -> bus_creator/352
  outpmodule/307(VOUTP_TailgaSWDTC_raw32) -> bus_creator/307
  outpmodule/350(VOUTP_RrMCUSigErrDetDTC_raw32) -> bus_creator/350
  bus_creator/1 -> BOUTP_outputs/1
  outpmodule/89(VOUTP_DriIntend_enum) -> bus_creator/89
  outpmodule/295(VOUTP_HVRlyOpDTC_raw32) -> bus_creator/295
  bus_selector2/19 -> outpmodule/22(VAPM_PASARMR_enum)  "<VAPM_PASARMR_enum>"
  outpmodule/87(VOUTP_ShifterHandleCmd_enum) -> bus_creator/87
  outpmodule/393(VOUTP_LimpHomeActTmp_flg) -> bus_creator/393
  outpmodule/88(VOUTP_ShifterHandleCmdTimeOut_flg) -> bus_creator/88
  outpmodule/298(VOUTP_IniLVLoDTC_raw32) -> bus_creator/298
  outpmodule/84(VOUTP_LRPulseCountTimeOut_flg) -> bus_creator/84
  bus_selector8/15 -> outpmodule/426(VPMM_RrMCUEnaReq_flg)  "<VPMM_RrMCUEnaReq_flg>"
  outpmodule/81(VOUTP_RFPulseCount_enum) -> bus_creator/81
  outpmodule/83(VOUTP_LRPulseCount_enum) -> bus_creator/83
  outpmodule/79(VOUTP_LFPulseCount_enum) -> bus_creator/79
  outpmodule/80(VOUTP_LFPulseCountTimeOut_flg) -> bus_creator/80
  outpmodule/78(VOUTP_RRPulseCountVTimeOut_flg) -> bus_creator/78
  outpmodule/76(VOUTP_LRPulseCountVTimeOut_flg) -> bus_creator/76
  outpmodule/74(VOUTP_RFPulseCountVTimeOut_flg) -> bus_creator/74
  outpmodule/75(VOUTP_LRPulseCountV_flg) -> bus_creator/75
  outpmodule/344(VOUTP_FCM5NoComDTC_raw32) -> bus_creator/344
  outpmodule/72(VOUTP_LFPulseCountVTimeOut_flg) -> bus_creator/72
  outpmodule/73(VOUTP_RFPulseCountV_flg) -> bus_creator/73
  outpmodule/69(VOUTP_RRWhlRotDir_enum) -> bus_creator/69
  bus_selector2/105 -> outpmodule/108(VAPM_LatAccelTimeOut_flg)  "<VAPM_LatAccelTimeOut_flg>"
  outpmodule/66(VOUTP_RFWhlRotDirTimeOut_flg) -> bus_creator/66
  outpmodule/67(VOUTP_LRWhlRotDir_enum) -> bus_creator/67
  outpmodule/68(VOUTP_LRWhlRotDirTimeOut_flg) -> bus_creator/68
  outpmodule/64(VOUTP_LFWhlRotDirTimeOut_flg) -> bus_creator/64
  outpmodule/65(VOUTP_RFWhlRotDir_enum) -> bus_creator/65
  outpmodule/61(VOUTP_RRRawWhlSpeedV_flg) -> bus_creator/61
  bus_selector4/100 -> outpmodule/361(VDDM_Shifter1RCErrDTC_raw32)  "<VDDM_Shifter1RCErrDTC_raw32>"
  outpmodule/62(VOUTP_RRRawWhlSpeedVTimeOut_flg) -> bus_creator/62
  outpmodule/63(VOUTP_LFWhlRotDir_enum) -> bus_creator/63
  outpmodule/59(VOUTP_LRRawWhlSpeedV_flg) -> bus_creator/59
  outpmodule/57(VOUTP_RFRawWhlSpeedV_flg) -> bus_creator/57
  outpmodule/654(VOUTP_WriteChkfinLFID_raw) -> bus_creator/654
  outpmodule/55(VOUTP_LFRawWhlSpeedV_flg) -> bus_creator/55
  bus_selector4/64 -> outpmodule/325(VDDM_FMLUSSDTC_raw32)  "<VDDM_FMLUSSDTC_raw32>"
  outpmodule/53(VOUTP_RRRawWhlSpeed_kph) -> bus_creator/53
  outpmodule/91(VOUTP_EPSAOIControl_enum) -> bus_creator/91
  outpmodule/49(VOUTP_RFRawWhlSpeed_kph) -> bus_creator/49
  outpmodule/50(VOUTP_RFRawWhlSpeedTimeOut_flg) -> bus_creator/50
  bus_selector8/31 -> outpmodule/442(VPMM_SilentChkAllowSleep_flg)  "<VPMM_SilentChkAllowSleep_flg>"
  outpmodule/47(VOUTP_LFRawWhlSpeed_kph) -> bus_creator/47
  outpmodule/310(VOUTP_APS2SigOoRDTC_raw32) -> bus_creator/310
  outpmodule/46(VOUTP_BrkPedalPosTimeOut_flg) -> bus_creator/46
  outpmodule/45(VOUTP_BrkPedalPos_pct) -> bus_creator/45
  bus_selector8/26 -> outpmodule/437(VPMM_EvccAplusPwrUpReq_flg)  "<VPMM_EvccAplusPwrUpReq_flg>"
  outpmodule/41(VOUTP_Chime_enum) -> bus_creator/41
  outpmodule/37(VOUTP_USSStaFLR_flg) -> bus_creator/37
  outpmodule/38(VOUTP_USSStaFLL_flg) -> bus_creator/38
  outpmodule/110(VOUTP_LongAccelTimeOut_flg) -> bus_creator/110
  outpmodule/107(VOUTP_LatAccel_Gps) -> bus_creator/107
  outpmodule/102(VOUTP_SASVTimeOut_flg) -> bus_creator/102
  outpmodule/103(VOUTP_GRADE_Deg) -> bus_creator/103
  outpmodule/104(VOUTP_GRADETimeOut_flg) -> bus_creator/104
  outpmodule/100(VOUTP_SASCALTimeOut_flg) -> bus_creator/100
  outpmodule/97(VOUTP_SASSpeedValid_flg) -> bus_creator/97
  bus_selector4/76 -> outpmodule/337(VDDM_FCM2RCErrDTC_raw32)  "<VDDM_FCM2RCErrDTC_raw32>"
  bus_selector9/27 -> outpmodule/486(VSYS_SHA6_cnt)  "<VSYS_SHA6_cnt>"
  outpmodule/94(VOUTP_SASAngleTimeOut_flg) -> bus_creator/94
  bus_selector4/72 -> outpmodule/333(VDDM_FLRUSSDTC_raw32)  "<VDDM_FLRUSSDTC_raw32>"
  outpmodule/93(VOUTP_SASAngle_Deg) -> bus_creator/93
  outpmodule/92(VOUTP_EPSAOIControlTimeOut_flg) -> bus_creator/92
  outpmodule/540(VOUTP_FootM_flg) -> bus_creator/540
  bus_selector4/133 -> outpmodule/394(VDDM_EDriveSysErr_VCUErrTmp_flg)  "<VDDM_EDriveSysErr_VCUErrTmp_flg>"
  bus_selector4/129 -> outpmodule/390(VDDM_EPBLockTODTC_raw32)  "<VDDM_EPBLockTODTC_raw32>"
  bus_selector4/130 -> outpmodule/391(VDDM_EPBUnlockTODTC_raw32)  "<VDDM_EPBUnlockTODTC_raw32>"
  bus_selector8/43 -> outpmodule/454(VPMM_CtrlDrPwrStbA2_flg)  "<VPMM_CtrlDrPwrStbA2_flg>"
  bus_selector4/131 -> outpmodule/392(VDDM_THCMAPTCWarning_raw32)  "<VDDM_THCMAPTCWarning_raw32>"
  bus_selector4/132 -> outpmodule/393(VDDM_LimpHomeActTmp_flg)  "<VDDM_LimpHomeActTmp_flg>"
  bus_selector4/127 -> outpmodule/388(VDDM_5vAPS1PwrErrDTC_raw32)  "<VDDM_5vAPS1PwrErrDTC_raw32>"
  bus_selector4/128 -> outpmodule/389(VDDM_5vAPS2PwrErrDTC_raw32)  "<VDDM_5vAPS2PwrErrDTC_raw32>"
  bus_selector4/125 -> outpmodule/386(VDDM_RRSensorFailDTC_raw32)  "<VDDM_RRSensorFailDTC_raw32>"
  bus_selector4/124 -> outpmodule/385(VDDM_LRSensorFailDTC_raw32)  "<VDDM_LRSensorFailDTC_raw32>"
  bus_selector4/121 -> outpmodule/382(VDDM_RRWheelTmpHighDTC_raw32)  "<VDDM_RRWheelTmpHighDTC_raw32>"
  outpmodule/317(VOUTP_ESC5NoComDTC_raw32) -> bus_creator/317
  bus_selector4/116 -> outpmodule/377(VDDM_LRPressIndiDTC_raw32)  "<VDDM_LRPressIndiDTC_raw32>"
  bus_selector4/119 -> outpmodule/380(VDDM_RFWheelTmpHighDTC_raw32)  "<VDDM_RFWheelTmpHighDTC_raw32>"
  bus_selector5/1 -> outpmodule/395(VDHP_ActAPSPosn_pct)  "<VDHP_ActAPSPosn_pct>"
  outpmodule/289(VOUTP_BMSRdyDTC_raw32) -> bus_creator/289
  bus_selector5/2 -> outpmodule/396(VDHP_EAPS1MIN_pct)  "<VDHP_EAPS1MIN_pct>"
  bus_selector4/36 -> outpmodule/297(VDDM_OBC4PreDTC_raw32)  "<VDDM_OBC4PreDTC_raw32>"
  bus_selector4/34 -> outpmodule/295(VDDM_HVRlyOpDTC_raw32)  "<VDDM_HVRlyOpDTC_raw32>"
  bus_selector4/35 -> outpmodule/296(VDDM_MCUActDTC_raw32)  "<VDDM_MCUActDTC_raw32>"
  bus_selector4/31 -> outpmodule/292(VDDM_MidLvSaChkDTC_raw32)  "<VDDM_MidLvSaChkDTC_raw32>"
  bus_selector4/29 -> outpmodule/290(VDDM_DCDCEnaDTC_raw32)  "<VDDM_DCDCEnaDTC_raw32>"
  bus_selector4/27 -> outpmodule/288(VDDM_HVRlyCloDTC_raw32)  "<VDDM_HVRlyCloDTC_raw32>"
  bus_selector3/94 -> outpmodule/259(VBCM_ATCtrl_enum)  "<VBCM_ATCtrl_enum>"
  bus_selector3/93 -> outpmodule/258(VBCM_LockAlarm_enum)  "<VBCM_LockAlarm_enum>"
  bus_selector3/92 -> outpmodule/257(VBCM_APMDoorControlSta_flg)  "<VBCM_APMDoorControlSta_flg>"
  bus_selector3/91 -> outpmodule/256(VBCM_LRRDCtrlCmd_pct)  "<VBCM_LRRDCtrlCmd_pct>"
  bus_selector3/88 -> outpmodule/253(VBCM_LDrvCtrlCmd_pct)  "<VBCM_LDrvCtrlCmd_pct>"
  bus_selector3/90 -> outpmodule/255(VBCM_LRLDCtrlCmd_pct)  "<VBCM_LRLDCtrlCmd_pct>"
  bus_selector3/87 -> outpmodule/252(VBCM_PTGInnerSW2_enum)  "<VBCM_PTGInnerSW2_enum>"
  bus_selector3/83 -> outpmodule/248(VBCM_FuelDoorPos_flg)  "<VBCM_FuelDoorPos_flg>"
  bus_selector3/84 -> outpmodule/249(VBCM_MFRDNBrightReq_pct)  "<VBCM_MFRDNBrightReq_pct>"
  bus_selector3/82 -> outpmodule/247(VBCM_MirrorFlodPos_flg)  "<VBCM_MirrorFlodPos_flg>"
  bus_selector4/48 -> outpmodule/309(VDDM_APS1SigOoRDTC_raw32)  "<VDDM_APS1SigOoRDTC_raw32>"
  bus_selector4/45 -> outpmodule/306(VDDM_HoodSWDTC_raw32)  "<VDDM_HoodSWDTC_raw32>"
  bus_selector8/13 -> outpmodule/424(VPMM_SysPowerMode_enum)  "<VPMM_SysPowerMode_enum>"
  bus_selector4/44 -> outpmodule/305(VDDM_RRDoorSWDTC_raw32)  "<VDDM_RRDoorSWDTC_raw32>"
  bus_selector4/41 -> outpmodule/302(VDDM_FLDoorSWDTC_raw32)  "<VDDM_FLDoorSWDTC_raw32>"
  bus_selector4/43 -> outpmodule/304(VDDM_FRDoorSWDTC_raw32)  "<VDDM_FRDoorSWDTC_raw32>"
  outpmodule/309(VOUTP_APS1SigOoRDTC_raw32) -> bus_creator/309
  bus_selector4/40 -> outpmodule/301(VDDM_DrStSWDTC_raw32)  "<VDDM_DrStSWDTC_raw32>"
  bus_selector4/38 -> outpmodule/299(VDDM_LVSupLoDTC_raw32)  "<VDDM_LVSupLoDTC_raw32>"
  bus_selector4/37 -> outpmodule/298(VDDM_IniLVLoDTC_raw32)  "<VDDM_IniLVLoDTC_raw32>"
  bus_selector8/19 -> outpmodule/430(VPMM_PwrStaConstraint_enum)  "<VPMM_PwrStaConstraint_enum>"
  bus_selector4/1 -> outpmodule/262(VDDM_C3BMS6RCDTC_raw32)  "<VDDM_C3BMS6RCDTC_raw32>"
  bus_selector4/3 -> outpmodule/264(VDDM_C3BMS6LCDTC_raw32)  "<VDDM_C3BMS6LCDTC_raw32>"
  bus_selector4/114 -> outpmodule/375(VDDM_LFPressIndiDTC_raw32)  "<VDDM_LFPressIndiDTC_raw32>"
  outpmodule/538(VOUTP_Frost_flg) -> bus_creator/538
  bus_selector4/2 -> outpmodule/263(VDDM_C3BMS6CSDTC_raw32)  "<VDDM_C3BMS6CSDTC_raw32>"
  bus_selector4/60 -> outpmodule/321(VDDM_DiagFRTSDTC_raw32)  "<VDDM_DiagFRTSDTC_raw32>"
  bus_selector4/61 -> outpmodule/322(VDDM_DiagRLTSDTC_raw32)  "<VDDM_DiagRLTSDTC_raw32>"
  bus_selector10/5 -> outpmodule/500(VTHC_FDEXV1Cmd_step)  "<VTHC_FDEXV1Cmd_step>"
  bus_selector4/49 -> outpmodule/310(VDDM_APS2SigOoRDTC_raw32)  "<VDDM_APS2SigOoRDTC_raw32>"
  bus_selector4/14 -> outpmodule/275(VDDM_C1ABM1CSDTC_raw32)  "<VDDM_C1ABM1CSDTC_raw32>"
  outpmodule/418(VOUTP_DCDCVoltSetpoint_V) -> bus_creator/418
  bus_selector4/13 -> outpmodule/274(VDDM_C1ABM1RCDTC_raw32)  "<VDDM_C1ABM1RCDTC_raw32>"
  outpmodule/676(VOUTP_TqSourceRr_enum) -> bus_creator/676
  bus_selector10/72 -> outpmodule/567(VTHC_CRVentEN_flg)  "<VTHC_CRVentEN_flg>"
  bus_selector4/15 -> outpmodule/276(VDDM_C1ABM1LCDTC_raw32)  "<VDDM_C1ABM1LCDTC_raw32>"
  bus_selector4/11 -> outpmodule/272(VDDM_C3CCU2CSDTC_raw32)  "<VDDM_C3CCU2CSDTC_raw32>"
  bus_selector4/5 -> outpmodule/266(VDDM_C3BMS1CSDTC_raw32)  "<VDDM_C3BMS1CSDTC_raw32>"
  bus_selector4/6 -> outpmodule/267(VDDM_C3BMS1LCDTC_raw32)  "<VDDM_C3BMS1LCDTC_raw32>"
  outpmodule/665(VOUTP_FlashS3ID_raw) -> bus_creator/665
  bus_selector15/10 -> outpmodule/731(VVMC_APSDecReq_mps2)  "<VVMC_APSDecReq_mps2>"
  bus_selector15/8 -> outpmodule/729(VVMC_APSStaSys_enum)  "<VVMC_APSStaSys_enum>"
  outpmodule/239(VOUTP_AmbLightColor3_enum) -> bus_creator/239
  bus_selector4/42 -> outpmodule/303(VDDM_RLDoorSWDTC_raw32)  "<VDDM_RLDoorSWDTC_raw32>"
  bus_selector15/5 -> outpmodule/726(VVMC_MSACtrlSta_enum)  "<VVMC_MSACtrlSta_enum>"
  bus_selector15/2 -> outpmodule/723(VVMC_ACCPedalOvrd_flg)  "<VVMC_ACCPedalOvrd_flg>"
  outpmodule/135(VOUTP_EPBSta_enum) -> bus_creator/135
  outpmodule/133(VOUTP_EPBErrSta_enum) -> bus_creator/133
  outpmodule/131(VOUTP_EPBExtApplyAvail_flg) -> bus_creator/131
  outpmodule/132(VOUTP_EPBExtApplyAvailTimeOut_flg) -> bus_creator/132
  outpmodule/128(VOUTP_ESCAPSStaTimeOut_flg) -> bus_creator/128
  bus_selector3/19 -> outpmodule/184(VBCM_CTDLockSW_flg)  "<VBCM_CTDLockSW_flg>"
  outpmodule/123(VOUTP_BrkSwV_flg) -> bus_creator/123
  outpmodule/124(VOUTP_BrkSwVTimeOut_flg) -> bus_creator/124
  outpmodule/121(VOUTP_BrkSwSta_flg) -> bus_creator/121
  outpmodule/118(VOUTP_LongAccelVTimeOut_flg) -> bus_creator/118
  outpmodule/116(VOUTP_LatAccelVTimeOut_flg) -> bus_creator/116
  outpmodule/115(VOUTP_LatAccelV_flg) -> bus_creator/115
  outpmodule/114(VOUTP_YawRateVTimeOut_flg) -> bus_creator/114
  bus_selector15/13 -> outpmodule/734(VVMC_CAASCtrlAvail_flg)  "<VVMC_CAASCtrlAvail_flg>"
  bus_selector3/43 -> outpmodule/208(VBCM_FrWiperL_flg)  "<VBCM_FrWiperL_flg>"
  bus_selector15/15 -> outpmodule/736(VVMC_ExtraMSACtrlSta_enum)  "<VVMC_ExtraMSACtrlSta_enum>"
  bus_selector15/12 -> outpmodule/733(VVMC_IMUEnaCmd_flg)  "<VVMC_IMUEnaCmd_flg>"
  bus_selector4/80 -> outpmodule/341(VDDM_FCM3CSErrDTC_raw32)  "<VDDM_FCM3CSErrDTC_raw32>"
  outpmodule/339(VOUTP_FCM3NoComDTC_raw32) -> bus_creator/339
  bus_selector15/14 -> outpmodule/735(VVMC_CAASActive_flg)  "<VVMC_CAASActive_flg>"
  bus_selector15/11 -> outpmodule/732(VVMC_APSReq_enum)  "<VVMC_APSReq_enum>"
  outpmodule/493(VOUTP_WisrBootReason_raw32) -> bus_creator/493
  outpmodule/416(VOUTP_ActiveDischargeReq_flg) -> bus_creator/416
  bus_selector3/64 -> outpmodule/229(VBCM_User5AmbLightColor_enum)  "<VBCM_User5AmbLightColor_enum>"
  bus_selector2/148 -> outpmodule/151(VAPM_ABSActive_flg)  "<VAPM_ABSActive_flg>"
  bus_selector2/152 -> outpmodule/155(VAPM_DriverSeatBeltCmd_flg)  "<VAPM_DriverSeatBeltCmd_flg>"
  outpmodule/496(VOUTP_FDCompCmd_rpm) -> bus_creator/496
  outpmodule/340(VOUTP_FCM3RCErrDTC_raw32) -> bus_creator/340
  outpmodule/563(VOUTP_FDCTHCMAPTCForceOFFSta_flg) -> bus_creator/563
  outpmodule/561(VOUTP_FDCTHCCREVentYSta_enum) -> bus_creator/561
  bus_selector9/3 -> outpmodule/462(VSYS_HWVer3_cnt)  "<VSYS_HWVer3_cnt>"
  bus_selector4/23 -> outpmodule/284(VDDM_ONtoRdyDTC_raw32)  "<VDDM_ONtoRdyDTC_raw32>"
  outpmodule/521(VOUTP_CCUSyncLampSts_flg) -> bus_creator/521
  outpmodule/520(VOUTP_CCUACMaxLampSts_flg) -> bus_creator/520
  outpmodule/519(VOUTP_CCUAutoLampSts_flg) -> bus_creator/519
  outpmodule/86(VOUTP_RRPulseCountTimeOut_flg) -> bus_creator/86
  outpmodule/518(VOUTP_CCUACLampSts_flg) -> bus_creator/518
  bus_selector9/33 -> outpmodule/492(VSYS_PmicBootReason_enum)  "<VSYS_PmicBootReason_enum>"
  outpmodule/517(VOUTP_CabinMode_enum) -> bus_creator/517
  outpmodule/220(VOUTP_User4IPAmbLightBrightness_enum) -> bus_creator/220
  outpmodule/515(VOUTP_BatteryMode_enum) -> bus_creator/515
  outpmodule/514(VOUTP_FDBlowerCmd_pct) -> bus_creator/514
  outpmodule/510(VOUTP_FDEWP3Cmd_enum) -> bus_creator/510
  outpmodule/509(VOUTP_FDEWP2Cmd_enum) -> bus_creator/509
  bus_selector15/1 -> outpmodule/722(VVMC_ACCCtrlAvail_flg)  "<VVMC_ACCCtrlAvail_flg>"
  outpmodule/505(VOUTP_FDFrWPTCHeatPwrCmd_W) -> bus_creator/505
  bus_selector3/65 -> outpmodule/230(VBCM_User6AmbLightColor_enum)  "<VBCM_User6AmbLightColor_enum>"
  outpmodule/504(VOUTP_FDTWVCmd_pct) -> bus_creator/504
  bus_selector1/3 -> outpmodule/3(VACC_VehHVPwrAvail4THCM_W)  "<VACC_VehHVPwrAvail4THCM_W>"
  outpmodule/134(VOUTP_EPBErrStaTimeOut_flg) -> bus_creator/134
  outpmodule/503(VOUTP_FDFWVCmd_flg) -> bus_creator/503
  outpmodule/502(VOUTP_FDSOTXVCmd_flg) -> bus_creator/502
  outpmodule/501(VOUTP_FDEXV2Cmd_step) -> bus_creator/501
  bus_selector2/2 -> outpmodule/5(VAPM_VehSpeedTimeOut_flg)  "<VAPM_VehSpeedTimeOut_flg>"
  outpmodule/500(VOUTP_FDEXV1Cmd_step) -> bus_creator/500
  outpmodule/207(VOUTP_TailgateHDSW_flg) -> bus_creator/207
  outpmodule/338(VOUTP_FCM2CSErrDTC_raw32) -> bus_creator/338
  outpmodule/202(VOUTP_MirrorDefog_flg) -> bus_creator/202
  bus_selector10/52 -> outpmodule/547(VTHC_sigDfrstSt_flg)  "<VTHC_sigDfrstSt_flg>"
  outpmodule/203(VOUTP_RrDefog_flg) -> bus_creator/203
  outpmodule/497(VOUTP_FDSOV1Cmd_flg) -> bus_creator/497
  bus_selector4/16 -> outpmodule/277(VDDM_Lv1ErrDTC_raw32)  "<VDDM_Lv1ErrDTC_raw32>"
  outpmodule/201(VOUTP_MirrorCtrl_enum) -> bus_creator/201
  outpmodule/198(VOUTP_LTurnLP_flg) -> bus_creator/198
  outpmodule/200(VOUTP_BCMBuzzerReq_flg) -> bus_creator/200
  bus_selector3/33 -> outpmodule/198(VBCM_LTurnLP_flg)  "<VBCM_LTurnLP_flg>"
  outpmodule/356(VOUTP_ISAMalfuncDetDTC_raw32) -> bus_creator/356
  outpmodule/197(VOUTP_HazardSW_flg) -> bus_creator/197
  outpmodule/194(VOUTP_RDRL_flg) -> bus_creator/194
  outpmodule/189(VOUTP_HBeam_flg) -> bus_creator/189
  outpmodule/188(VOUTP_LBeam_flg) -> bus_creator/188
  outpmodule/648(VOUTP_LRPindi_enum) -> bus_creator/648
  outpmodule/184(VOUTP_CTDLockSW_flg) -> bus_creator/184
  bus_selector3/96 -> outpmodule/261(VBCM_OutMode_enum)  "<VBCM_OutMode_enum>"
  outpmodule/183(VOUTP_DoorLockIND_flg) -> bus_creator/183
  outpmodule/557(VOUTP_FDCTHCCLEVentYSta_enum) -> bus_creator/557
  outpmodule/182(VOUTP_CTDCtrl_enum) -> bus_creator/182
  outpmodule/180(VOUTP_RrChargingDoorCtrl_enum) -> bus_creator/180
  outpmodule/178(VOUTP_LockSetting_flg) -> bus_creator/178
  outpmodule/177(VOUTP_RRDoorSW_flg) -> bus_creator/177
  outpmodule/176(VOUTP_RLDoorSW_flg) -> bus_creator/176
  outpmodule/173(VOUTP_TailgateSW_flg) -> bus_creator/173
  outpmodule/172(VOUTP_HoodSW_flg) -> bus_creator/172
  outpmodule/171(VOUTP_AntitheftSeatFlod_flg) -> bus_creator/171
  outpmodule/169(VOUTP_AllDoorSW_flg) -> bus_creator/169
  bus_selector2/66 -> outpmodule/69(VAPM_RRWhlRotDir_enum)  "<VAPM_RRWhlRotDir_enum>"
  outpmodule/168(VOUTP_HornCtrl_flg) -> bus_creator/168
  outpmodule/167(VOUTP_TailgateRemote_enum) -> bus_creator/167
  outpmodule/267(VOUTP_C3BMS1LCDTC_raw32) -> bus_creator/267
  outpmodule/166(VOUTP_AntitheftSta_enum) -> bus_creator/166
  bus_selector2/161 -> outpmodule/164(VAPM_APSRqEPASCtrl_flg)  "<VAPM_APSRqEPASCtrl_flg>"
  outpmodule/217(VOUTP_User3DrAmbLightBrightness_enum) -> bus_creator/217
  bus_selector4/82 -> outpmodule/343(VDDM_FCM4CSErrDTC_raw32)  "<VDDM_FCM4CSErrDTC_raw32>"
  outpmodule/216(VOUTP_User2IPAmbLightBrightness_enum) -> bus_creator/216
  outpmodule/215(VOUTP_User2DrAmbLightBrightness_enum) -> bus_creator/215
  bus_selector4/47 -> outpmodule/308(VDDM_VehMalfunLevel_enum)  "<VDDM_VehMalfunLevel_enum>"
  outpmodule/214(VOUTP_User1IPAmbLightBrightness_enum) -> bus_creator/214
  outpmodule/213(VOUTP_User1DrAmbLightBrightness_enum) -> bus_creator/213
  bus_selector3/45 -> outpmodule/210(VBCM_RrWiper_flg)  "<VBCM_RrWiper_flg>"
  outpmodule/211(VOUTP_WasherCtrl_enum) -> bus_creator/211
  bus_selector4/111 -> outpmodule/372(VDDM_RFBatwarnDTC_raw32)  "<VDDM_RFBatwarnDTC_raw32>"
  outpmodule/733(VOUTP_IMUEnaCmd_flg) -> bus_creator/733
  outpmodule/735(VOUTP_CAASActive_flg) -> bus_creator/735
  outpmodule/731(VOUTP_APSDecReq_mps2) -> bus_creator/731
  outpmodule/729(VOUTP_APSStaSys_enum) -> bus_creator/729
  outpmodule/678(VOUTP_RrEDUAvailBrkRgnTq_Nm) -> bus_creator/678
  outpmodule/42(VOUTP_SNSRLayout_enum) -> bus_creator/42
  outpmodule/727(VOUTP_APSCtrlAvail_flg) -> bus_creator/727
  outpmodule/90(VOUTP_DriIntendTimeOut_flg) -> bus_creator/90
  outpmodule/726(VOUTP_MSACtrlSta_enum) -> bus_creator/726
  outpmodule/722(VOUTP_ACCCtrlAvail_flg) -> bus_creator/722
  outpmodule/720(VOUTP_ReqOBCV2LEna_enum) -> bus_creator/720
  bus_selector10/34 -> outpmodule/529(VTHC_sigClntTHvBattIn_C)  "<VTHC_sigClntTHvBattIn_C>"
  outpmodule/718(VOUTP_FrTMTqReq_Nm) -> bus_creator/718
  outpmodule/719(VOUTP_RrTMTqReq_Nm) -> bus_creator/719
  outpmodule/716(VOUTP_OPDHoldLamp_flg) -> bus_creator/716
  bus_selector10/78 -> outpmodule/573(VTHC_FDCFGSIONSWSta_flg)  "<VTHC_FDCFGSIONSWSta_flg>"
  outpmodule/105(VOUTP_YawRate_degps) -> bus_creator/105
  outpmodule/714(VOUTP_ActParkRequest_flg) -> bus_creator/714
  outpmodule/71(VOUTP_LFPulseCountV_flg) -> bus_creator/71
  outpmodule/711(VOUTP_CreepON_flg) -> bus_creator/711
  outpmodule/713(VOUTP_DriveProtEn_flg) -> bus_creator/713
  outpmodule/710(VOUTP_ReBrakeLPReq_flg) -> bus_creator/710
  outpmodule/707(VOUTP_RrIdcMax_A) -> bus_creator/707
  outpmodule/706(VOUTP_RrIdcMin_A) -> bus_creator/706
  outpmodule/195(VOUTP_LBSD_flg) -> bus_creator/195
  outpmodule/708(VOUTP_RrUdcMin_V) -> bus_creator/708
  outpmodule/671(VOUTP_TPMSSensorIDRegStart_flg) -> bus_creator/671
  bus_selector3/80 -> outpmodule/245(VBCM_CountAlarm_enum)  "<VBCM_CountAlarm_enum>"
  outpmodule/704(VOUTP_FrUdcMin_V) -> bus_creator/704
  outpmodule/705(VOUTP_FrUdcMax_V) -> bus_creator/705
  outpmodule/99(VOUTP_SASCAL_flg) -> bus_creator/99
  outpmodule/703(VOUTP_FrIdcMax_A) -> bus_creator/703
  outpmodule/699(VOUTP_PTCSPermSta_flg) -> bus_creator/699
  outpmodule/696(VOUTP_RrEDUSpdValid_flg) -> bus_creator/696
  outpmodule/698(VOUTP_RgnAbnorSta_flg) -> bus_creator/698
  outpmodule/113(VOUTP_YawRateV_flg) -> bus_creator/113
  outpmodule/694(VOUTP_FrEDUSpdValid_flg) -> bus_creator/694
  bus_selector4/63 -> outpmodule/324(VDDM_FCLUSSDTC_raw32)  "<VDDM_FCLUSSDTC_raw32>"
  bus_selector15/9 -> outpmodule/730(VVMC_APSDecReqA_flg)  "<VVMC_APSDecReqA_flg>"
  outpmodule/691(VOUTP_RrEDURolRgnTq_Nm) -> bus_creator/691
  outpmodule/305(VOUTP_RRDoorSWDTC_raw32) -> bus_creator/305
  outpmodule/690(VOUTP_FrEDURolRgnTq_Nm) -> bus_creator/690
  outpmodule/125(VOUTP_ESCStandstill_flg) -> bus_creator/125
  outpmodule/687(VOUTP_DriverWhlTqDemRr_Nm) -> bus_creator/687
  outpmodule/684(VOUTP_FrRgnDecrSta_flg) -> bus_creator/684
  outpmodule/136(VOUTP_EPBStaTimeOut_flg) -> bus_creator/136
  outpmodule/683(VOUTP_RrActvDmpDisabReq_flg) -> bus_creator/683
  outpmodule/682(VOUTP_FrActvDmpDisabReq_flg) -> bus_creator/682
  bus_selector3/58 -> outpmodule/223(VBCM_User6DrAmbLightBrightness_enum)  "<VBCM_User6DrAmbLightBrightness_enum>"
  outpmodule/422(VOUTP_LVPwrSta_flg) -> bus_creator/422
  outpmodule/681(VOUTP_PButtonSta_enum) -> bus_creator/681
  bus_selector11/78 -> outpmodule/654(VTPM_WriteChkfinLFID_raw)  "<VTPM_WriteChkfinLFID_raw>"
  bus_selector11/77 -> outpmodule/653(VTPM_WriteChkRRID_raw)  "<VTPM_WriteChkRRID_raw>"
  bus_selector11/74 -> outpmodule/650(VTPM_WriteChkLFID_raw)  "<VTPM_WriteChkLFID_raw>"
  bus_selector11/76 -> outpmodule/652(VTPM_WriteChkLRID_raw)  "<VTPM_WriteChkLRID_raw>"
  bus_selector4/30 -> outpmodule/291(VDDM_HiLvSaChkDTC_raw32)  "<VDDM_HiLvSaChkDTC_raw32>"
  bus_selector11/70 -> outpmodule/646(VTPM_LFPindi_enum)  "<VTPM_LFPindi_enum>"
  bus_selector11/71 -> outpmodule/647(VTPM_RFPind_enum)  "<VTPM_RFPind_enum>"
  bus_selector11/69 -> outpmodule/645(VTPM_TPMSResButt_flg)  "<VTPM_TPMSResButt_flg>"
  bus_selector11/97 -> outpmodule/673(VTPM_ModelVersionChksum_raw)  "<VTPM_ModelVersionChksum_raw>"
  bus_selector8/27 -> outpmodule/438(VPMM_PwrStaONTOPopReq_flg)  "<VPMM_PwrStaONTOPopReq_flg>"
  bus_selector11/68 -> outpmodule/644(VTPM_ChkStorge_flg)  "<VTPM_ChkStorge_flg>"
  outpmodule/175(VOUTP_PsDoorSW_flg) -> bus_creator/175
  bus_selector11/93 -> outpmodule/669(VTPM_TPMSTLCmd_flg)  "<VTPM_TPMSTLCmd_flg>"
  bus_selector11/95 -> outpmodule/671(VTPM_TPMSSensorIDRegStart_flg)  "<VTPM_TPMSSensorIDRegStart_flg>"
  bus_selector11/92 -> outpmodule/668(VTPM_WritingCnt_enum)  "<VTPM_WritingCnt_enum>"
  outpmodule/270(VOUTP_C3CCU1LCDTC_raw32) -> bus_creator/270
  bus_selector11/88 -> outpmodule/664(VTPM_FlashS2ID_raw)  "<VTPM_FlashS2ID_raw>"
  bus_selector11/89 -> outpmodule/665(VTPM_FlashS3ID_raw)  "<VTPM_FlashS3ID_raw>"
  bus_selector11/86 -> outpmodule/662(VTPM_Prepresstempvalid_enum)  "<VTPM_Prepresstempvalid_enum>"
  bus_selector8/1 -> outpmodule/412(VPMM_PowerUpState_enum)  "<VPMM_PowerUpState_enum>"
  bus_selector9/32 -> outpmodule/491(VSYS_FdcSlpTime_sec)  "<VSYS_FdcSlpTime_sec>"
  bus_selector7/10 -> outpmodule/409(VNMM_ActiveWU_flg)  "<VNMM_ActiveWU_flg>"
  bus_selector7/12 -> outpmodule/411(VNMM_NetworkReq_flg)  "<VNMM_NetworkReq_flg>"
  outpmodule/120(VOUTP_MCPressureVTimeOut_flg) -> bus_creator/120
  outpmodule/323(VOUTP_DiagRRTSDTC_raw32) -> bus_creator/323
  bus_selector4/126 -> outpmodule/387(VDDM_C1EPAS2LCDTC_raw32)  "<VDDM_C1EPAS2LCDTC_raw32>"
  bus_selector7/8 -> outpmodule/407(VNMM_RptMsgReq_flg)  "<VNMM_RptMsgReq_flg>"
  bus_selector7/7 -> outpmodule/406(VNMM_PNI_flg)  "<VNMM_PNI_flg>"
  bus_selector8/8 -> outpmodule/419(VPMM_HVBatCnctReq_flg)  "<VPMM_HVBatCnctReq_flg>"
  bus_selector10/76 -> outpmodule/571(VTHC_FDCFGSFuncSta_flg)  "<VTHC_FDCFGSFuncSta_flg>"
  bus_selector2/22 -> outpmodule/25(VAPM_PASARCL_enum)  "<VAPM_PASARCL_enum>"
  outpmodule/498(VOUTP_FDSOV2Cmd_flg) -> bus_creator/498
  BVMC_outputs/1 -> bus_selector15/1
  bus_selector2/24 -> outpmodule/27(VAPM_PASAFML_enum)  "<VAPM_PASAFML_enum>"
  outpmodule/672(VOUTP_ModelVersion_raw) -> bus_creator/672
  bus_selector2/25 -> outpmodule/28(VAPM_PASAFCR_enum)  "<VAPM_PASAFCR_enum>"
  bus_selector2/1 -> outpmodule/4(VAPM_VehSpeed_kph)  "<VAPM_VehSpeed_kph>"
  outpmodule/475(VOUTP_Country2_cnt) -> bus_creator/475
  bus_selector4/50 -> outpmodule/311(VDDM_APSCorrErrDTC_raw32)  "<VDDM_APSCorrErrDTC_raw32>"
  outpmodule/470(VOUTP_Minor1_cnt) -> bus_creator/470
  outpmodule/469(VOUTP_Major2_cnt) -> bus_creator/469
  outpmodule/715(VOUTP_IVIPwrLockSta_enum) -> bus_creator/715
  outpmodule/465(VOUTP_CarModel3_cnt) -> bus_creator/465
  outpmodule/461(VOUTP_HWVer2_cnt) -> bus_creator/461
  bus_selector2/20 -> outpmodule/23(VAPM_PASARML_enum)  "<VAPM_PASARML_enum>"
  outpmodule/450(VOUTP_CtrlFrRC1_flg) -> bus_creator/450
  bus_selector11/81 -> outpmodule/657(VTPM_WriteChkfinRRID_raw)  "<VTPM_WriteChkfinRRID_raw>"
  bus_selector2/116 -> outpmodule/119(VAPM_MCPressureV_bar)  "<VAPM_MCPressureV_bar>"
  outpmodule/451(VOUTP_CtrlFrBMSCCUCIR_flg) -> bus_creator/451
  outpmodule/449(VOUTP_CtrlFrPwrStbA1P_flg) -> bus_creator/449
  bus_selector4/26 -> outpmodule/287(VDDM_DCDC4PreDTC_raw32)  "<VDDM_DCDC4PreDTC_raw32>"
  outpmodule/445(VOUTP_PMMAllowECUSleep_flg) -> bus_creator/445
  outpmodule/230(VOUTP_User6AmbLightColor_enum) -> bus_creator/230
  outpmodule/446(VOUTP_LVSilentChrgSta_enum) -> bus_creator/446
  bus_selector3/49 -> outpmodule/214(VBCM_User1IPAmbLightBrightness_enum)  "<VBCM_User1IPAmbLightBrightness_enum>"
  outpmodule/444(VOUTP_FDADC12VDetAvg_mV) -> bus_creator/444
  bus_selector3/62 -> outpmodule/227(VBCM_User3AmbLightColor_enum)  "<VBCM_User3AmbLightColor_enum>"
  outpmodule/193(VOUTP_LDRL_flg) -> bus_creator/193
  outpmodule/443(VOUTP_TimerAllowSleep_flg) -> bus_creator/443
  bus_selector4/112 -> outpmodule/373(VDDM_LRBatwarnDTC_raw32)  "<VDDM_LRBatwarnDTC_raw32>"
  outpmodule/181(VOUTP_CrashDetd_flg) -> bus_creator/181
  outpmodule/442(VOUTP_SilentChkAllowSleep_flg) -> bus_creator/442
  outpmodule/686(VOUTP_DriverWhlTqDemFr_Nm) -> bus_creator/686
  outpmodule/119(VOUTP_MCPressureV_bar) -> bus_creator/119
  outpmodule/435(VOUTP_ReVehThdChkSta_enum) -> bus_creator/435
  bus_selector9/18 -> outpmodule/477(VSYS_Dash1_cnt)  "<VSYS_Dash1_cnt>"
  outpmodule/430(VOUTP_PwrStaConstraint_enum) -> bus_creator/430
  bus_selector11/75 -> outpmodule/651(VTPM_WriteChkRFID_raw)  "<VTPM_WriteChkRFID_raw>"
  bus_selector4/4 -> outpmodule/265(VDDM_C3BMS1RCDTC_raw32)  "<VDDM_C3BMS1RCDTC_raw32>"
  outpmodule/431(VOUTP_TCountSta_enum) -> bus_creator/431
  outpmodule/429(VOUTP_PwrStaSelect_enum) -> bus_creator/429
  bus_selector2/96 -> outpmodule/99(VAPM_SASCAL_flg)  "<VAPM_SASCAL_flg>"
  bus_selector8/41 -> outpmodule/452(VPMM_CtrlFrEDUINVERTER_flg)  "<VPMM_CtrlFrEDUINVERTER_flg>"
  outpmodule/494(VOUTP_AcoreRebootCmdACK_flg) -> bus_creator/494
  outpmodule/337(VOUTP_FCM2RCErrDTC_raw32) -> bus_creator/337
  outpmodule/664(VOUTP_FlashS2ID_raw) -> bus_creator/664
  outpmodule/204(VOUTP_RoomLampH_flg) -> bus_creator/204
  outpmodule/426(VOUTP_RrMCUEnaReq_flg) -> bus_creator/426
  outpmodule/427(VOUTP_DrivetrainSelect_enum) -> bus_creator/427
  outpmodule/551(VOUTP_FDCTHCDrEVentZSta_enum) -> bus_creator/551
  outpmodule/734(VOUTP_CAASCtrlAvail_flg) -> bus_creator/734
  outpmodule/491(VOUTP_FdcSlpTime_sec) -> bus_creator/491
  bus_selector2/49 -> outpmodule/52(VAPM_LRRawWhlSpeedTimeOut_flg)  "<VAPM_LRRawWhlSpeedTimeOut_flg>"
  outpmodule/490(VOUTP_FdcSlpReqRisingEdge_flg) -> bus_creator/490
  outpmodule/303(VOUTP_RLDoorSWDTC_raw32) -> bus_creator/303
  bus_selector11/91 -> outpmodule/667(VTPM_FlashIDvalid_enum)  "<VTPM_FlashIDvalid_enum>"
  outpmodule/669(VOUTP_TPMSTLCmd_flg) -> bus_creator/669
  outpmodule/723(VOUTP_ACCPedalOvrd_flg) -> bus_creator/723
  outpmodule/675(VOUTP_TqSourceFr_enum) -> bus_creator/675
  outpmodule/191(VOUTP_BrakeLamp_flg) -> bus_creator/191
  outpmodule/487(VOUTP_SHA7_cnt) -> bus_creator/487
  outpmodule/481(VOUTP_SHA1_cnt) -> bus_creator/481
  outpmodule/480(VOUTP_Dash2_cnt) -> bus_creator/480
  outpmodule/477(VOUTP_Dash1_cnt) -> bus_creator/477
  outpmodule/476(VOUTP_Variation_cnt) -> bus_creator/476
  outpmodule/31(VOUTP_USSStaRLR_flg) -> bus_creator/31
  bus_selector2/156 -> outpmodule/159(VAPM_APSSWVer_enum)  "<VAPM_APSSWVer_enum>"
  outpmodule/456(VOUTP_Sched_ChgTOSta_enum) -> bus_creator/456
  outpmodule/32(VOUTP_USSStaRLL_flg) -> bus_creator/32
  outpmodule/30(VOUTP_USSStaRML_flg) -> bus_creator/30
  outpmodule/28(VOUTP_PASAFCR_enum) -> bus_creator/28
  outpmodule/26(VOUTP_PASAFMR_enum) -> bus_creator/26
  outpmodule/44(VOUTP_ModOperation_enum) -> bus_creator/44
  outpmodule/25(VOUTP_PASARCL_enum) -> bus_creator/25
  outpmodule/452(VOUTP_CtrlFrEDUINVERTER_flg) -> bus_creator/452
  bus_selector2/112 -> outpmodule/115(VAPM_LatAccelV_flg)  "<VAPM_LatAccelV_flg>"
  outpmodule/20(VOUTP_APSDFLL_cm) -> bus_creator/20
  bus_selector4/65 -> outpmodule/326(VDDM_FMRUSSDTC_raw32)  "<VDDM_FMRUSSDTC_raw32>"
  bus_selector2/27 -> outpmodule/30(VAPM_USSStaRML_flg)  "<VAPM_USSStaRML_flg>"
  outpmodule/48(VOUTP_LFRawWhlSpeedTimeOut_flg) -> bus_creator/48
  outpmodule/483(VOUTP_SHA3_cnt) -> bus_creator/483
  bus_selector8/4 -> outpmodule/415(VPMM_PowerDownFault_enum)  "<VPMM_PowerDownFault_enum>"
  outpmodule/19(VOUTP_APSDFLR_cm) -> bus_creator/19
  outpmodule/18(VOUTP_APSDRLL_cm) -> bus_creator/18
  outpmodule/508(VOUTP_FDEWP1Cmd_enum) -> bus_creator/508
  outpmodule/11(VOUTP_PASDRCR_cm) -> bus_creator/11
  bus_selector9/8 -> outpmodule/467(VSYS_ECU2_cnt)  "<VSYS_ECU2_cnt>"
  outpmodule/10(VOUTP_PASDRML_cm) -> bus_creator/10
  bus_selector3/1 -> outpmodule/166(VBCM_AntitheftSta_enum)  "<VBCM_AntitheftSta_enum>"
  bus_selector11/73 -> outpmodule/649(VTPM_RRPindi_enum)  "<VTPM_RRPindi_enum>"
  outpmodule/190(VOUTP_RrFogLamp_flg) -> bus_creator/190
  outpmodule/9(VOUTP_PASDRMR_cm) -> bus_creator/9
  bus_selector4/91 -> outpmodule/352(VDDM_ACCAccelCmdErrDetDTC_raw32)  "<VDDM_ACCAccelCmdErrDetDTC_raw32>"
  outpmodule/724(VOUTP_CCCtrlSta_enum) -> bus_creator/724
  outpmodule/106(VOUTP_YawRateTimeOut_flg) -> bus_creator/106
  outpmodule/495(VOUTP_CurrentNmState_enum) -> bus_creator/495
  bus_selector2/40 -> outpmodule/43(VAPM_StaFSya_flg)  "<VAPM_StaFSya_flg>"
  outpmodule/7(VOUTP_FSOffSwTimeOut_flg) -> bus_creator/7
  outpmodule/5(VOUTP_VehSpeedTimeOut_flg) -> bus_creator/5
  bus_selector2/162 -> outpmodule/165(VAPM_CAASSta_enum)  "<VAPM_CAASSta_enum>"
  outpmodule/6(VOUTP_FSOffSw_enum) -> bus_creator/6
  outpmodule/657(VOUTP_WriteChkfinRRID_raw) -> bus_creator/657
  outpmodule/1(VOUTP_HVTHCMSysAvail_enum) -> bus_creator/1
  bus_selector11/72 -> outpmodule/648(VTPM_LRPindi_enum)  "<VTPM_LRPindi_enum>"
  outpmodule/555(VOUTP_FDCTHCDrEVentYSta_enum) -> bus_creator/555
  outpmodule/464(VOUTP_CarModel2_cnt) -> bus_creator/464
  outpmodule/35(VOUTP_USSStaFMR_flg) -> bus_creator/35
  outpmodule/448(VOUTP_LVSilentChrgLv_enum) -> bus_creator/448
  outpmodule/351(VOUTP_CCUSigErrDetDTC_raw32) -> bus_creator/351
  outpmodule/36(VOUTP_USSStaFML_flg) -> bus_creator/36
  outpmodule/545(VOUTP_fdefog_flg) -> bus_creator/545
  bus_selector2/145 -> outpmodule/148(VAPM_CAASSwTimeOut_flg)  "<VAPM_CAASSwTimeOut_flg>"
  bus_selector11/82 -> outpmodule/658(VTPM_Flashchkdatavalid_enum)  "<VTPM_Flashchkdatavalid_enum>"
  bus_selector2/153 -> outpmodule/156(VAPM_DriverSeatBeltCmdTimeOut_flg)  "<VAPM_DriverSeatBeltCmdTimeOut_flg>"
  bus_selector2/140 -> outpmodule/143(VAPM_AVMErrSTA_flg)  "<VAPM_AVMErrSTA_flg>"
  bus_selector4/9 -> outpmodule/270(VDDM_C3CCU1LCDTC_raw32)  "<VDDM_C3CCU1LCDTC_raw32>"
  outpmodule/95(VOUTP_SASSpeed_degps) -> bus_creator/95
  outpmodule/466(VOUTP_ECU1_cnt) -> bus_creator/466
  bus_selector4/123 -> outpmodule/384(VDDM_RFSensorFailDTC_raw32)  "<VDDM_RFSensorFailDTC_raw32>"
  outpmodule/130(VOUTP_EPBExtReleaseAvailTimeOut_flg) -> bus_creator/130
  bus_selector2/151 -> outpmodule/154(VAPM_TCSActiveTimeOut_flg)  "<VAPM_TCSActiveTimeOut_flg>"
  outpmodule/433(VOUTP_PwrDownReq_enum) -> bus_creator/433
  bus_selector2/136 -> outpmodule/139(VAPM_AVMparkingexcute_enum)  "<VAPM_AVMparkingexcute_enum>"
  bus_selector2/146 -> outpmodule/149(VAPM_IVIScreen_enum)  "<VAPM_IVIScreen_enum>"
  outpmodule/24(VOUTP_PASARCR_enum) -> bus_creator/24
  bus_selector8/3 -> outpmodule/414(VPMM_PowerUpFault_enum)  "<VPMM_PowerUpFault_enum>"
  bus_selector2/147 -> outpmodule/150(VAPM_IVIScreenTimeOut_flg)  "<VAPM_IVIScreenTimeOut_flg>"
  outpmodule/573(VOUTP_FDCFGSIONSWSta_flg) -> bus_creator/573
  outpmodule/572(VOUTP_FDCFGSChCmd_enum) -> bus_creator/572
  outpmodule/571(VOUTP_FDCFGSFuncSta_flg) -> bus_creator/571
  bus_selector11/79 -> outpmodule/655(VTPM_WriteChkfinRFID_raw)  "<VTPM_WriteChkfinRFID_raw>"
  outpmodule/499(VOUTP_FDSOV3Cmd_flg) -> bus_creator/499
  outpmodule/569(VOUTP_FDCFGSChSta_enum) -> bus_creator/569
  outpmodule/568(VOUTP_FDCFGSAirIntSta_enum) -> bus_creator/568
  bus_selector4/39 -> outpmodule/300(VDDM_LVSupHiDTC_raw32)  "<VDDM_LVSupHiDTC_raw32>"
  outpmodule/566(VOUTP_PsVentEN_flg) -> bus_creator/566
  outpmodule/642(VOUTP_SetIDLoc_flg) -> bus_creator/642
  bus_selector4/95 -> outpmodule/356(VDDM_ISAMalfuncDetDTC_raw32)  "<VDDM_ISAMalfuncDetDTC_raw32>"
  outpmodule/334(VOUTP_RLLUSSDTC_raw32) -> bus_creator/334
  outpmodule/697(VOUTP_RrEDUAvailBrkRgnTqV_flg) -> bus_creator/697
  outpmodule/111(VOUTP_MCPressure_bar) -> bus_creator/111
  outpmodule/567(VOUTP_CRVentEN_flg) -> bus_creator/567
  bus_selector2/117 -> outpmodule/120(VAPM_MCPressureVTimeOut_flg)  "<VAPM_MCPressureVTimeOut_flg>"
  outpmodule/471(VOUTP_Minor2_cnt) -> bus_creator/471
  outpmodule/56(VOUTP_LFRawWhlSpeedVTimeOut_flg) -> bus_creator/56
  outpmodule/565(VOUTP_CLVentEN_flg) -> bus_creator/565
  bus_selector2/144 -> outpmodule/147(VAPM_CAASSw_enum)  "<VAPM_CAASSw_enum>"
  bus_selector3/89 -> outpmodule/254(VBCM_LPasCtrlCmd_pct)  "<VBCM_LPasCtrlCmd_pct>"
  outpmodule/641(VOUTP_Chkfin_flg) -> bus_creator/641
  outpmodule/640(VOUTP_ID4messageALTU_raw8) -> bus_creator/640
  outpmodule/54(VOUTP_RRRawWhlSpeedTimeOut_flg) -> bus_creator/54
  outpmodule/637(VOUTP_ID1messageALTU_raw8) -> bus_creator/637
  bus_selector3/31 -> outpmodule/196(VBCM_RBSD_flg)  "<VBCM_RBSD_flg>"
  outpmodule/635(VOUTP_S3WheelDebugALTU_pct) -> bus_creator/635
  outpmodule/633(VOUTP_S1WheelDebugALTU_pct) -> bus_creator/633
  outpmodule/428(VOUTP_DrSeatSta_enum) -> bus_creator/428
  bus_selector10/47 -> outpmodule/542(VTHC_ACForceOFF_flg)  "<VTHC_ACForceOFF_flg>"
  bus_selector1/1 -> outpmodule/1(VACC_HVTHCMSysAvail_enum)  "<VACC_HVTHCMSysAvail_enum>"
  outpmodule/634(VOUTP_S2WheelDebugALTU_pct) -> bus_creator/634
  outpmodule/12(VOUTP_PASDRCL_cm) -> bus_creator/12
  outpmodule/630(VOUTP_RRP20_raw8) -> bus_creator/630
  outpmodule/398(VOUTP_DKCTimeSN_cnt) -> bus_creator/398
  outpmodule/628(VOUTP_RFP20_raw8) -> bus_creator/628
  outpmodule/8(VOUTP_ChrgPlugSta_enum) -> bus_creator/8
  outpmodule/629(VOUTP_LRP20_raw8) -> bus_creator/629
  outpmodule/165(VOUTP_CAASSta_enum) -> bus_creator/165
  outpmodule/627(VOUTP_LFP20_raw8) -> bus_creator/627
  bus_selector10/23 -> outpmodule/518(VTHC_CCUACLampSts_flg)  "<VTHC_CCUACLampSts_flg>"
  outpmodule/438(VOUTP_PwrStaONTOPopReq_flg) -> bus_creator/438
  outpmodule/621(VOUTP_S4ID_raw32) -> bus_creator/621
  bus_selector7/3 -> outpmodule/402(VNMM_Awake_enum)  "<VNMM_Awake_enum>"
  bus_selector2/17 -> outpmodule/20(VAPM_APSDFLL_cm)  "<VAPM_APSDFLL_cm>"
  outpmodule/39(VOUTP_USSStaFCR_flg) -> bus_creator/39
  outpmodule/622(VOUTP_S1L_enum) -> bus_creator/622
  outpmodule/235(VOUTP_AmbLightBrightness2_enum) -> bus_creator/235
  outpmodule/620(VOUTP_S3ID_raw32) -> bus_creator/620
  outpmodule/618(VOUTP_S1ID_raw32) -> bus_creator/618
  outpmodule/22(VOUTP_PASARMR_enum) -> bus_creator/22
  outpmodule/460(VOUTP_HWVer1_cnt) -> bus_creator/460
  bus_selector3/86 -> outpmodule/251(VBCM_IVIPTGUSStaSW_flg)  "<VBCM_IVIPTGUSStaSW_flg>"
  outpmodule/615(VOUTP_RFSensorMode_flg) -> bus_creator/615
  bus_selector7/9 -> outpmodule/408(VNMM_WakeUp_enum)  "<VNMM_WakeUp_enum>"
  outpmodule/663(VOUTP_FlashS1ID_raw) -> bus_creator/663
  outpmodule/614(VOUTP_LFSensorMode_flg) -> bus_creator/614
  bus_selector2/122 -> outpmodule/125(VAPM_ESCStandstill_flg)  "<VAPM_ESCStandstill_flg>"
  bus_selector9/22 -> outpmodule/481(VSYS_SHA1_cnt)  "<VSYS_SHA1_cnt>"
  outpmodule/612(VOUTP_CWheelTips_enum) -> bus_creator/612
  bus_selector7/11 -> outpmodule/410(VNMM_SysNMmSta_enum)  "<VNMM_SysNMmSta_enum>"
  outpmodule/611(VOUTP_RRWheelPSW_raw8) -> bus_creator/611
  outpmodule/488(VOUTP_SHA8_cnt) -> bus_creator/488
  outpmodule/610(VOUTP_RFWheelPSW_raw8) -> bus_creator/610
  outpmodule/609(VOUTP_LRWheelPSW_raw8) -> bus_creator/609
  outpmodule/603(VOUTP_TPMSWarnIndi_enum) -> bus_creator/603
  outpmodule/244(VOUTP_IVIRST_flg) -> bus_creator/244
  bus_selector11/90 -> outpmodule/666(VTPM_FlashS4ID_raw)  "<VTPM_FlashS4ID_raw>"
  bus_selector2/158 -> outpmodule/161(VAPM_APSExitCondition_enum)  "<VAPM_APSExitCondition_enum>"
  bus_selector8/16 -> outpmodule/427(VPMM_DrivetrainSelect_enum)  "<VPMM_DrivetrainSelect_enum>"
  outpmodule/604(VOUTP_LFWheelTmpIndi_flg) -> bus_creator/604
  outpmodule/219(VOUTP_User4DrAmbLightBrightness_enum) -> bus_creator/219
  outpmodule/701(VOUTP_RrRgnPermSta_flg) -> bus_creator/701
  outpmodule/192(VOUTP_ReverseLamp_flg) -> bus_creator/192
  outpmodule/602(VOUTP_RRPressIndi_enum) -> bus_creator/602
  BSYS_outputs/1 -> bus_selector9/1
  outpmodule/485(VOUTP_SHA5_cnt) -> bus_creator/485
  outpmodule/601(VOUTP_LRPressIndi_enum) -> bus_creator/601
  bus_selector2/62 -> outpmodule/65(VAPM_RFWhlRotDir_enum)  "<VAPM_RFWhlRotDir_enum>"
  bus_selector9/11 -> outpmodule/470(VSYS_Minor1_cnt)  "<VSYS_Minor1_cnt>"
  BBCM_outputs/1 -> bus_selector3/1
  outpmodule/600(VOUTP_RFPressIndi_enum) -> bus_creator/600
  bus_selector9/17 -> outpmodule/476(VSYS_Variation_cnt)  "<VSYS_Variation_cnt>"
  outpmodule/632(VOUTP_IDin_raw32) -> bus_creator/632
  outpmodule/597(VOUTP_TPMSResButtAllow_flg) -> bus_creator/597
  outpmodule/489(VOUTP_NvWriteReqRisingEdge_flg) -> bus_creator/489
  outpmodule/595(VOUTP_RFWheelDebug_flg) -> bus_creator/595
  outpmodule/592(VOUTP_RRSensorFail_flg) -> bus_creator/592
  outpmodule/702(VOUTP_FrIdcMin_A) -> bus_creator/702
  outpmodule/82(VOUTP_RFPulseCountTimeOut_flg) -> bus_creator/82
  outpmodule/590(VOUTP_RFSensorFail_flg) -> bus_creator/590
  outpmodule/117(VOUTP_LongAccelV_flg) -> bus_creator/117
  outpmodule/589(VOUTP_LFSensorFail_flg) -> bus_creator/589
  outpmodule/662(VOUTP_Prepresstempvalid_enum) -> bus_creator/662
  outpmodule/586(VOUTP_RFWheelTemp_C) -> bus_creator/586
  outpmodule/34(VOUTP_USSStaRCL_flg) -> bus_creator/34
  outpmodule/585(VOUTP_LFWheelTemp_C) -> bus_creator/585
  outpmodule/440(VOUTP_LVChrgHoldTtimer_s) -> bus_creator/440
  outpmodule/582(VOUTP_RFWheelPress_raw8) -> bus_creator/582
  outpmodule/315(VOUTP_ESC7NoComDTC_raw32) -> bus_creator/315
  outpmodule/4(VOUTP_VehSpeed_kph) -> bus_creator/4
  outpmodule/229(VOUTP_User5AmbLightColor_enum) -> bus_creator/229
  outpmodule/583(VOUTP_LRWheelPress_raw8) -> bus_creator/583
  outpmodule/308(VOUTP_VehMalfunLevel_enum) -> bus_creator/308
  outpmodule/43(VOUTP_StaFSya_flg) -> bus_creator/43
  bus_selector2/141 -> outpmodule/144(VAPM_AVMErrSTATimeOut_flg)  "<VAPM_AVMErrSTATimeOut_flg>"
  outpmodule/580(VOUTP_RRBatWarn_flg) -> bus_creator/580
  bus_selector2/32 -> outpmodule/35(VAPM_USSStaFMR_flg)  "<VAPM_USSStaFMR_flg>"
  outpmodule/210(VOUTP_RrWiper_flg) -> bus_creator/210
  outpmodule/576(VOUTP_FDCTHCMPreWPTCHeatSta_enum) -> bus_creator/576
  outpmodule/23(VOUTP_PASARML_enum) -> bus_creator/23
  outpmodule/577(VOUTP_LFBatWarn_flg) -> bus_creator/577
  outpmodule/578(VOUTP_RFBatWarn_flg) -> bus_creator/578
  outpmodule/646(VOUTP_LFPindi_enum) -> bus_creator/646
  outpmodule/575(VOUTP_FDCFGSLearnCmd_enum) -> bus_creator/575
  BV2L_outputs/1 -> bus_selector14/1
  outpmodule/288(VOUTP_HVRlyCloDTC_raw32) -> bus_creator/288
  outpmodule/164(VOUTP_APSRqEPASCtrl_flg) -> bus_creator/164
  bus_selector2/150 -> outpmodule/153(VAPM_TCSActive_flg)  "<VAPM_TCSActive_flg>"
  outpmodule/17(VOUTP_APSDRLR_cm) -> bus_creator/17
  outpmodule/397(VOUTP_EAPS2MIN_pct) -> bus_creator/397
  outpmodule/333(VOUTP_FLRUSSDTC_raw32) -> bus_creator/333
  outpmodule/162(VOUTP_APSAngleTarget_Deg) -> bus_creator/162
  bus_selector2/14 -> outpmodule/17(VAPM_APSDRLR_cm)  "<VAPM_APSDRLR_cm>"
  outpmodule/21(VOUTP_PASAFCL_enum) -> bus_creator/21
  outpmodule/161(VOUTP_APSExitCondition_enum) -> bus_creator/161
  bus_selector4/46 -> outpmodule/307(VDDM_TailgaSWDTC_raw32)  "<VDDM_TailgaSWDTC_raw32>"
  outpmodule/159(VOUTP_APSSWVer_enum) -> bus_creator/159
  bus_selector2/42 -> outpmodule/45(VAPM_BrkPedalPos_pct)  "<VAPM_BrkPedalPos_pct>"
  outpmodule/732(VOUTP_APSReq_enum) -> bus_creator/732
  bus_selector3/85 -> outpmodule/250(VBCM_RoomLampMode_flg)  "<VBCM_RoomLampMode_flg>"
  outpmodule/596(VOUTP_RRWheelDebug_flg) -> bus_creator/596
  outpmodule/16(VOUTP_PASDFCL_cm) -> bus_creator/16
  outpmodule/158(VOUTP_APSRQDisplay_enum) -> bus_creator/158
  bus_selector4/117 -> outpmodule/378(VDDM_RRPressIndiDTC_raw32)  "<VDDM_RRPressIndiDTC_raw32>"
  outpmodule/155(VOUTP_DriverSeatBeltCmd_flg) -> bus_creator/155
  bus_selector2/83 -> outpmodule/86(VAPM_RRPulseCountTimeOut_flg)  "<VAPM_RRPulseCountTimeOut_flg>"
  BDDM_outputs/1 -> bus_selector4/1
  bus_selector10/60 -> outpmodule/555(VTHC_FDCTHCDrEVentYSta_enum)  "<VTHC_FDCTHCDrEVentYSta_enum>"
  outpmodule/403(VOUTP_CSB_flg) -> bus_creator/403
  outpmodule/564(VOUTP_DrVentEN_flg) -> bus_creator/564
  outpmodule/154(VOUTP_TCSActiveTimeOut_flg) -> bus_creator/154
  outpmodule/322(VOUTP_DiagRLTSDTC_raw32) -> bus_creator/322
  outpmodule/153(VOUTP_TCSActive_flg) -> bus_creator/153
  outpmodule/151(VOUTP_ABSActive_flg) -> bus_creator/151
  bus_selector2/74 -> outpmodule/77(VAPM_RRPulseCountV_flg)  "<VAPM_RRPulseCountV_flg>"
  outpmodule/152(VOUTP_ABSActiveTimeOut_flg) -> bus_creator/152
  outpmodule/150(VOUTP_IVIScreenTimeOut_flg) -> bus_creator/150
  outpmodule/149(VOUTP_IVIScreen_enum) -> bus_creator/149
  outpmodule/700(VOUTP_FrRgnPermSta_flg) -> bus_creator/700
  outpmodule/147(VOUTP_CAASSw_enum) -> bus_creator/147
  outpmodule/736(VOUTP_ExtraMSACtrlSta_enum) -> bus_creator/736
  outpmodule/146(VOUTP_IVIStatusTimeOut_flg) -> bus_creator/146
  outpmodule/148(VOUTP_CAASSwTimeOut_flg) -> bus_creator/148
  bus_selector4/120 -> outpmodule/381(VDDM_LRWheelTmpHighDTC_raw32)  "<VDDM_LRWheelTmpHighDTC_raw32>"
  outpmodule/143(VOUTP_AVMErrSTA_flg) -> bus_creator/143
  bus_selector2/138 -> outpmodule/141(VAPM_AVMParkingmode_enum)  "<VAPM_AVMParkingmode_enum>"
  outpmodule/651(VOUTP_WriteChkRFID_raw) -> bus_creator/651
  outpmodule/140(VOUTP_AVMparkingexcuteTimeOut_flg) -> bus_creator/140
  outpmodule/138(VOUTP_AVMparkingcancelTimeOut_flg) -> bus_creator/138
  bus_selector2/43 -> outpmodule/46(VAPM_BrkPedalPosTimeOut_flg)  "<VAPM_BrkPedalPosTimeOut_flg>"
  outpmodule/599(VOUTP_LFPressIndi_enum) -> bus_creator/599
  bus_selector12/7 -> outpmodule/680(VTQD_ShiftGearPosn_enum)  "<VTQD_ShiftGearPosn_enum>"
  outpmodule/345(VOUTP_FCM5CSErrDTC_raw32) -> bus_creator/345
  outpmodule/144(VOUTP_AVMErrSTATimeOut_flg) -> bus_creator/144
  bus_selector12/8 -> outpmodule/681(VTQD_PButtonSta_enum)  "<VTQD_PButtonSta_enum>"
  outpmodule/218(VOUTP_User3IPAmbLightBrightness_enum) -> bus_creator/218
  bus_selector12/6 -> outpmodule/679(VTQD_EVDriveMode_enum)  "<VTQD_EVDriveMode_enum>"
  outpmodule/474(VOUTP_Country1_cnt) -> bus_creator/474
  bus_selector9/9 -> outpmodule/468(VSYS_Major1_cnt)  "<VSYS_Major1_cnt>"
  bus_selector12/5 -> outpmodule/678(VTQD_RrEDUAvailBrkRgnTq_Nm)  "<VTQD_RrEDUAvailBrkRgnTq_Nm>"
  bus_selector2/139 -> outpmodule/142(VAPM_AVMParkingmodeTimeOut_flg)  "<VAPM_AVMParkingmodeTimeOut_flg>"
  bus_selector12/4 -> outpmodule/677(VTQD_FrEDUAvailBrkRgnTq_Nm)  "<VTQD_FrEDUAvailBrkRgnTq_Nm>"
  bus_selector8/23 -> outpmodule/434(VPMM_LowSOCWarn_enum)  "<VPMM_LowSOCWarn_enum>"
  outpmodule/631(VOUTP_FAT_flg) -> bus_creator/631
  bus_selector12/3 -> outpmodule/676(VTQD_TqSourceRr_enum)  "<VTQD_TqSourceRr_enum>"
  bus_selector12/43 -> outpmodule/716(VTQD_OPDHoldLamp_flg)  "<VTQD_OPDHoldLamp_flg>"
  outpmodule/728(VOUTP_APSActive_flg) -> bus_creator/728
  bus_selector4/69 -> outpmodule/330(VDDM_RMRUSSDTC_raw32)  "<VDDM_RMRUSSDTC_raw32>"
  outpmodule/594(VOUTP_LRWheelDebug_flg) -> bus_creator/594
  bus_selector10/74 -> outpmodule/569(VTHC_FDCFGSChSta_enum)  "<VTHC_FDCFGSChSta_enum>"
  outpmodule/129(VOUTP_EPBExtReleaseAvail_flg) -> bus_creator/129
  bus_selector12/40 -> outpmodule/713(VTQD_DriveProtEn_flg)  "<VTQD_DriveProtEn_flg>"
  bus_selector12/41 -> outpmodule/714(VTQD_ActParkRequest_flg)  "<VTQD_ActParkRequest_flg>"
  bus_selector12/44 -> outpmodule/717(VTQD_VehActSpd_kph)  "<VTQD_VehActSpd_kph>"
  outpmodule/141(VOUTP_AVMParkingmode_enum) -> bus_creator/141
  outpmodule/581(VOUTP_LFWheelPress_raw8) -> bus_creator/581
  bus_selector3/95 -> outpmodule/260(VBCM_fUnlockSingle_flg)  "<VBCM_fUnlockSingle_flg>"
  bus_selector8/9 -> outpmodule/420(VPMM_HVSysReadyToCharge_enum)  "<VPMM_HVSysReadyToCharge_enum>"
  bus_selector12/39 -> outpmodule/712(VTQD_EquivAccPedalSWSta_flg)  "<VTQD_EquivAccPedalSWSta_flg>"
  bus_selector3/34 -> outpmodule/199(VBCM_RTurnLP_flg)  "<VBCM_RTurnLP_flg>"
  outpmodule/472(VOUTP_Patch1_cnt) -> bus_creator/472
  bus_selector12/36 -> outpmodule/709(VTQD_RrUdcMax_V)  "<VTQD_RrUdcMax_V>"
  bus_selector12/34 -> outpmodule/707(VTQD_RrIdcMax_A)  "<VTQD_RrIdcMax_A>"
  bus_selector6/2 -> outpmodule/399(VDKC_DKCAuthSta_enum)  "<VDKC_DKCAuthSta_enum>"
  bus_selector12/33 -> outpmodule/706(VTQD_RrIdcMin_A)  "<VTQD_RrIdcMin_A>"
  outpmodule/652(VOUTP_WriteChkLRID_raw) -> bus_creator/652
  bus_selector8/5 -> outpmodule/416(VPMM_ActiveDischargeReq_flg)  "<VPMM_ActiveDischargeReq_flg>"
  bus_selector3/38 -> outpmodule/203(VBCM_RrDefog_flg)  "<VBCM_RrDefog_flg>"
  outpmodule/608(VOUTP_LFWheelPSW_raw8) -> bus_creator/608
  bus_selector12/32 -> outpmodule/705(VTQD_FrUdcMax_V)  "<VTQD_FrUdcMax_V>"
  outpmodule/437(VOUTP_EvccAplusPwrUpReq_flg) -> bus_creator/437
  bus_selector4/90 -> outpmodule/351(VDDM_CCUSigErrDetDTC_raw32)  "<VDDM_CCUSigErrDetDTC_raw32>"
  bus_selector12/31 -> outpmodule/704(VTQD_FrUdcMin_V)  "<VTQD_FrUdcMin_V>"
  bus_selector12/30 -> outpmodule/703(VTQD_FrIdcMax_A)  "<VTQD_FrIdcMax_A>"
  bus_selector12/29 -> outpmodule/702(VTQD_FrIdcMin_A)  "<VTQD_FrIdcMin_A>"
  bus_selector9/14 -> outpmodule/473(VSYS_Patch2_cnt)  "<VSYS_Patch2_cnt>"
  bus_selector12/26 -> outpmodule/699(VTQD_PTCSPermSta_flg)  "<VTQD_PTCSPermSta_flg>"
  bus_selector12/27 -> outpmodule/700(VTQD_FrRgnPermSta_flg)  "<VTQD_FrRgnPermSta_flg>"
  outpmodule/157(VOUTP_APSProgressPCT_pct) -> bus_creator/157
  bus_selector8/14 -> outpmodule/425(VPMM_FrMCUEnaReq_flg)  "<VPMM_FrMCUEnaReq_flg>"
  bus_selector9/16 -> outpmodule/475(VSYS_Country2_cnt)  "<VSYS_Country2_cnt>"
  bus_selector12/22 -> outpmodule/695(VTQD_FrEDUAvailBrkRgnTqV_flg)  "<VTQD_FrEDUAvailBrkRgnTqV_flg>"
  bus_selector3/13 -> outpmodule/178(VBCM_LockSetting_flg)  "<VBCM_LockSetting_flg>"
  outpmodule/233(VOUTP_AmbLightBreath3_flg) -> bus_creator/233
  bus_selector12/21 -> outpmodule/694(VTQD_FrEDUSpdValid_flg)  "<VTQD_FrEDUSpdValid_flg>"
  outpmodule/677(VOUTP_FrEDUAvailBrkRgnTq_Nm) -> bus_creator/677
  bus_selector12/23 -> outpmodule/696(VTQD_RrEDUSpdValid_flg)  "<VTQD_RrEDUSpdValid_flg>"
  outpmodule/432(VOUTP_PwrUpReq_enum) -> bus_creator/432
  bus_selector4/71 -> outpmodule/332(VDDM_FLLUSSDTC_raw32)  "<VDDM_FLLUSSDTC_raw32>"
  bus_selector12/24 -> outpmodule/697(VTQD_RrEDUAvailBrkRgnTqV_flg)  "<VTQD_RrEDUAvailBrkRgnTqV_flg>"
  outpmodule/208(VOUTP_FrWiperL_flg) -> bus_creator/208
  bus_selector12/17 -> outpmodule/690(VTQD_FrEDURolRgnTq_Nm)  "<VTQD_FrEDURolRgnTq_Nm>"
  outpmodule/689(VOUTP_RrEDUActTq_Nm) -> bus_creator/689
  bus_selector12/16 -> outpmodule/689(VTQD_RrEDUActTq_Nm)  "<VTQD_RrEDUActTq_Nm>"
  bus_selector12/19 -> outpmodule/692(VTQD_FrEDUSpd_rpm)  "<VTQD_FrEDUSpd_rpm>"
  bus_selector12/14 -> outpmodule/687(VTQD_DriverWhlTqDemRr_Nm)  "<VTQD_DriverWhlTqDemRr_Nm>"
  bus_selector2/73 -> outpmodule/76(VAPM_LRPulseCountVTimeOut_flg)  "<VAPM_LRPulseCountVTimeOut_flg>"
  bus_selector8/32 -> outpmodule/443(VPMM_TimerAllowSleep_flg)  "<VPMM_TimerAllowSleep_flg>"
  bus_selector12/12 -> outpmodule/685(VTQD_RrRgnDecrSta_flg)  "<VTQD_RrRgnDecrSta_flg>"
  outpmodule/240(VOUTP_LampPwr_flg) -> bus_creator/240
  bus_selector12/13 -> outpmodule/686(VTQD_DriverWhlTqDemFr_Nm)  "<VTQD_DriverWhlTqDemFr_Nm>"
  bus_selector4/7 -> outpmodule/268(VDDM_C3CCU1RCDTC_raw32)  "<VDDM_C3CCU1RCDTC_raw32>"
  BNMM_outputs/1 -> bus_selector7/1
  bus_selector8/25 -> outpmodule/436(VPMM_LVSysErrPwrOutErr_flg)  "<VPMM_LVSysErrPwrOutErr_flg>"
  bus_selector12/11 -> outpmodule/684(VTQD_FrRgnDecrSta_flg)  "<VTQD_FrRgnDecrSta_flg>"
  bus_selector7/2 -> outpmodule/401(VNMM_NMmTxReq_flg)  "<VNMM_NMmTxReq_flg>"
  bus_selector12/10 -> outpmodule/683(VTQD_RrActvDmpDisabReq_flg)  "<VTQD_RrActvDmpDisabReq_flg>"
  outpmodule/528(VOUTP_sigCbnSolarLeft_W) -> bus_creator/528
  bus_selector2/128 -> outpmodule/131(VAPM_EPBExtApplyAvail_flg)  "<VAPM_EPBExtApplyAvail_flg>"
  outpmodule/27(VOUTP_PASAFML_enum) -> bus_creator/27
  outpmodule/283(VOUTP_KeyAuthDTC_raw32) -> bus_creator/283
  outpmodule/613(VOUTP_AutoLTips_enum) -> bus_creator/613
  bus_selector2/127 -> outpmodule/130(VAPM_EPBExtReleaseAvailTimeOut_flg)  "<VAPM_EPBExtReleaseAvailTimeOut_flg>"
  outpmodule/639(VOUTP_ID3messageALTU_raw8) -> bus_creator/639
  bus_selector2/126 -> outpmodule/129(VAPM_EPBExtReleaseAvail_flg)  "<VAPM_EPBExtReleaseAvail_flg>"
  outpmodule/439(VOUTP_IVIPwrStaONTOPopT_s) -> bus_creator/439
  bus_selector9/25 -> outpmodule/484(VSYS_SHA4_cnt)  "<VSYS_SHA4_cnt>"
  outpmodule/447(VOUTP_LVSilentChrgReq_flg) -> bus_creator/447
  bus_selector2/125 -> outpmodule/128(VAPM_ESCAPSStaTimeOut_flg)  "<VAPM_ESCAPSStaTimeOut_flg>"
  outpmodule/693(VOUTP_RrEDUSpd_rpm) -> bus_creator/693
  bus_selector2/124 -> outpmodule/127(VAPM_ESCAPSSta_enum)  "<VAPM_ESCAPSSta_enum>"
  outpmodule/273(VOUTP_C3CCU2LCDTC_raw32) -> bus_creator/273
  outpmodule/467(VOUTP_ECU2_cnt) -> bus_creator/467
  bus_selector2/130 -> outpmodule/133(VAPM_EPBErrSta_enum)  "<VAPM_EPBErrSta_enum>"
  bus_selector2/94 -> outpmodule/97(VAPM_SASSpeedValid_flg)  "<VAPM_SASSpeedValid_flg>"
  bus_selector2/97 -> outpmodule/100(VAPM_SASCALTimeOut_flg)  "<VAPM_SASCALTimeOut_flg>"
  outpmodule/507(VOUTP_FDAGSCmd_enum) -> bus_creator/507
  outpmodule/77(VOUTP_RRPulseCountV_flg) -> bus_creator/77
  outpmodule/655(VOUTP_WriteChkfinRFID_raw) -> bus_creator/655
  bus_selector2/98 -> outpmodule/101(VAPM_SASV_flg)  "<VAPM_SASV_flg>"
  outpmodule/324(VOUTP_FCLUSSDTC_raw32) -> bus_creator/324
  bus_selector4/57 -> outpmodule/318(VDDM_EnterNewOperCyc_flg)  "<VDDM_EnterNewOperCyc_flg>"
  bus_selector2/57 -> outpmodule/60(VAPM_LRRawWhlSpeedVTimeOut_flg)  "<VAPM_LRRawWhlSpeedVTimeOut_flg>"
  outpmodule/108(VOUTP_LatAccelTimeOut_flg) -> bus_creator/108
  outpmodule/587(VOUTP_LRWheelTemp_C) -> bus_creator/587
  outpmodule/363(VOUTP_ESC7RCErrDTC_raw32) -> bus_creator/363
  outpmodule/364(VOUTP_ESC7CSErrDTC_raw32) -> bus_creator/364
  bus_selector12/1 -> outpmodule/674(VTQD_ParkRequest_flg)  "<VTQD_ParkRequest_flg>"
  outpmodule/362(VOUTP_Shifter1CSErrDTC_raw32) -> bus_creator/362
  outpmodule/361(VOUTP_Shifter1RCErrDTC_raw32) -> bus_creator/361
  outpmodule/605(VOUTP_RFWheelTmpIndi_flg) -> bus_creator/605
  outpmodule/127(VOUTP_ESCAPSSta_enum) -> bus_creator/127
  outpmodule/268(VOUTP_C3CCU1RCDTC_raw32) -> bus_creator/268
  bus_selector2/143 -> outpmodule/146(VAPM_IVIStatusTimeOut_flg)  "<VAPM_IVIStatusTimeOut_flg>"
  outpmodule/15(VOUTP_PASDFCR_cm) -> bus_creator/15
  outpmodule/358(VOUTP_MCUR1RCErrDTC_raw32) -> bus_creator/358
  bus_selector2/90 -> outpmodule/93(VAPM_SASAngle_Deg)  "<VAPM_SASAngle_Deg>"
  outpmodule/359(VOUTP_MCUF1CSErrDTC_raw32) -> bus_creator/359
  outpmodule/96(VOUTP_SASSpeedTimeOut_flg) -> bus_creator/96
  bus_selector4/67 -> outpmodule/328(VDDM_RCLUSSDTC_raw32)  "<VDDM_RCLUSSDTC_raw32>"
  outpmodule/420(VOUTP_HVSysReadyToCharge_enum) -> bus_creator/420
  bus_selector11/80 -> outpmodule/656(VTPM_WriteChkfinLRID_raw)  "<VTPM_WriteChkfinLRID_raw>"
  outpmodule/276(VOUTP_C1ABM1LCDTC_raw32) -> bus_creator/276
  outpmodule/376(VOUTP_RFPressIndiDTC_raw32) -> bus_creator/376
  outpmodule/375(VOUTP_LFPressIndiDTC_raw32) -> bus_creator/375
  outpmodule/511(VOUTP_FDFrLeAPTCHeatPwrCmd_W) -> bus_creator/511
  bus_selector9/19 -> outpmodule/478(VSYS_Change1_cnt)  "<VSYS_Change1_cnt>"
  outpmodule/374(VOUTP_RRBatwarnDTC_raw32) -> bus_creator/374
  outpmodule/373(VOUTP_LRBatwarnDTC_raw32) -> bus_creator/373
  bus_selector2/53 -> outpmodule/56(VAPM_LFRawWhlSpeedVTimeOut_flg)  "<VAPM_LFRawWhlSpeedVTimeOut_flg>"
  outpmodule/372(VOUTP_RFBatwarnDTC_raw32) -> bus_creator/372
  bus_selector15/3 -> outpmodule/724(VVMC_CCCtrlSta_enum)  "<VVMC_CCCtrlSta_enum>"
  outpmodule/436(VOUTP_LVSysErrPwrOutErr_flg) -> bus_creator/436
  outpmodule/112(VOUTP_MCPressureTimeOut_flg) -> bus_creator/112
  outpmodule/371(VOUTP_LFBatwarnDTC_raw32) -> bus_creator/371
  bus_selector12/28 -> outpmodule/701(VTQD_RrRgnPermSta_flg)  "<VTQD_RrRgnPermSta_flg>"
  bus_selector7/1 -> outpmodule/400(VNMM_AllCANTxReq_flg)  "<VNMM_AllCANTxReq_flg>"
  outpmodule/370(VOUTP_RrMCUTqErrDTC_raw32) -> bus_creator/370
  outpmodule/369(VOUTP_FrMCUTqErrDTC_raw32) -> bus_creator/369
  bus_selector9/24 -> outpmodule/483(VSYS_SHA3_cnt)  "<VSYS_SHA3_cnt>"
  outpmodule/512(VOUTP_FDFrRiAPTCHeatPwrCmd_W) -> bus_creator/512
  bus_selector4/33 -> outpmodule/294(VDDM_DCDCDisDTC_raw32)  "<VDDM_DCDCDisDTC_raw32>"
  outpmodule/366(VOUTP_ESC1CSErrDTC_raw32) -> bus_creator/366
  outpmodule/695(VOUTP_FrEDUAvailBrkRgnTqV_flg) -> bus_creator/695
  outpmodule/142(VOUTP_AVMParkingmodeTimeOut_flg) -> bus_creator/142
  outpmodule/365(VOUTP_ESC1RCErrDTC_raw32) -> bus_creator/365
  bus_selector4/55 -> outpmodule/316(VDDM_ESC1NoComDTC_raw32)  "<VDDM_ESC1NoComDTC_raw32>"
  bus_selector9/36 -> outpmodule/495(VSYS_CurrentNmState_enum)  "<VSYS_CurrentNmState_enum>"
  bus_selector6/1 -> outpmodule/398(VDKC_DKCTimeSN_cnt)  "<VDKC_DKCTimeSN_cnt>"
  BDHP_outputs/1 -> bus_selector5/1
  bus_selector2/119 -> outpmodule/122(VAPM_BrkSwStaTimeOut_flg)  "<VAPM_BrkSwStaTimeOut_flg>"
  outpmodule/137(VOUTP_AVMparkingcancel_enum) -> bus_creator/137
  outpmodule/33(VOUTP_USSStaRCR_flg) -> bus_creator/33
  bus_selector2/102 -> outpmodule/105(VAPM_YawRate_degps)  "<VAPM_YawRate_degps>"
  outpmodule/139(VOUTP_AVMparkingexcute_enum) -> bus_creator/139
  outpmodule/286(VOUTP_MCU4PreDTC_raw32) -> bus_creator/286
  bus_selector10/68 -> outpmodule/563(VTHC_FDCTHCMAPTCForceOFFSta_flg)  "<VTHC_FDCTHCMAPTCForceOFFSta_flg>"
  bus_selector2/118 -> outpmodule/121(VAPM_BrkSwSta_flg)  "<VAPM_BrkSwSta_flg>"
  outpmodule/353(VOUTP_ACCMalfuncDetDTC_raw32) -> bus_creator/353
  outpmodule/482(VOUTP_SHA2_cnt) -> bus_creator/482
  outpmodule/680(VOUTP_ShiftGearPosn_enum) -> bus_creator/680
  outpmodule/196(VOUTP_RBSD_flg) -> bus_creator/196
  bus_selector4/81 -> outpmodule/342(VDDM_FCM4NoComDTC_raw32)  "<VDDM_FCM4NoComDTC_raw32>"
  outpmodule/98(VOUTP_SASSpeedValidTimeOut_flg) -> bus_creator/98
  outpmodule/606(VOUTP_LRWheelTmpIndi_flg) -> bus_creator/606
  bus_selector2/39 -> outpmodule/42(VAPM_SNSRLayout_enum)  "<VAPM_SNSRLayout_enum>"
  bus_selector9/5 -> outpmodule/464(VSYS_CarModel2_cnt)  "<VSYS_CarModel2_cnt>"
  outpmodule/725(VOUTP_CCMSASpdWar_flg) -> bus_creator/725
  outpmodule/262(VOUTP_C3BMS6RCDTC_raw32) -> bus_creator/262
  bus_selector4/51 -> outpmodule/312(VDDM_MCUF1NoComDTC_raw32)  "<VDDM_MCUF1NoComDTC_raw32>"
  outpmodule/486(VOUTP_SHA6_cnt) -> bus_creator/486
  outpmodule/410(VOUTP_SysNMmSta_enum) -> bus_creator/410
  bus_selector8/2 -> outpmodule/413(VPMM_PowerDownState_enum)  "<VPMM_PowerDownState_enum>"
  bus_selector11/96 -> outpmodule/672(VTPM_ModelVersion_raw)  "<VTPM_ModelVersion_raw>"
  bus_selector4/52 -> outpmodule/313(VDDM_MCUR1NoComDTC_raw32)  "<VDDM_MCUR1NoComDTC_raw32>"
  bus_selector8/12 -> outpmodule/423(VPMM_HVPwrSta_flg)  "<VPMM_HVPwrSta_flg>"
  bus_selector4/59 -> outpmodule/320(VDDM_DiagFLTSDTC_raw32)  "<VDDM_DiagFLTSDTC_raw32>"
  bus_selector4/58 -> outpmodule/319(VDDM_DiagHCrashDTC_raw32)  "<VDDM_DiagHCrashDTC_raw32>"
  bus_selector10/64 -> outpmodule/559(VTHC_FDCTHCPsEVentYSta_enum)  "<VTHC_FDCTHCPsEVentYSta_enum>"
  bus_selector15/7 -> outpmodule/728(VVMC_APSActive_flg)  "<VVMC_APSActive_flg>"
  bus_selector4/53 -> outpmodule/314(VDDM_Shifter1NoComDTC_raw32)  "<VDDM_Shifter1NoComDTC_raw32>"
  outpmodule/458(VOUTP_OTAPwrReqOFFChkSta_enum) -> bus_creator/458
  bus_selector4/54 -> outpmodule/315(VDDM_ESC7NoComDTC_raw32)  "<VDDM_ESC7NoComDTC_raw32>"
  bus_selector2/142 -> outpmodule/145(VAPM_IVIStatus_flg)  "<VAPM_IVIStatus_flg>"
  bus_selector9/1 -> outpmodule/460(VSYS_HWVer1_cnt)  "<VSYS_HWVer1_cnt>"
  outpmodule/52(VOUTP_LRRawWhlSpeedTimeOut_flg) -> bus_creator/52
  outpmodule/619(VOUTP_S2ID_raw32) -> bus_creator/619
  bus_selector4/56 -> outpmodule/317(VDDM_ESC5NoComDTC_raw32)  "<VDDM_ESC5NoComDTC_raw32>"
  bus_selector4/12 -> outpmodule/273(VDDM_C3CCU2LCDTC_raw32)  "<VDDM_C3CCU2LCDTC_raw32>"
  BTQR_outputs/1 -> bus_selector13/1
  outpmodule/455(VOUTP_PwrStaTOSta_enum) -> bus_creator/455
  bus_selector13/2 -> outpmodule/719(VTQR_RrTMTqReq_Nm)  "<VTQR_RrTMTqReq_Nm>"
  BTQD_outputs/1 -> bus_selector12/1
  bus_selector3/20 -> outpmodule/185(VBCM_Dimmer_pct)  "<VBCM_Dimmer_pct>"
  outpmodule/616(VOUTP_LRSensorMode_flg) -> bus_creator/616
  bus_selector13/1 -> outpmodule/718(VTQR_FrTMTqReq_Nm)  "<VTQR_FrTMTqReq_Nm>"
  outpmodule/574(VOUTP_FDCFGSIONCmd_flg) -> bus_creator/574
  bus_selector4/28 -> outpmodule/289(VDDM_BMSRdyDTC_raw32)  "<VDDM_BMSRdyDTC_raw32>"
  outpmodule/692(VOUTP_FrEDUSpd_rpm) -> bus_creator/692
  outpmodule/653(VOUTP_WriteChkRRID_raw) -> bus_creator/653
  bus_selector2/52 -> outpmodule/55(VAPM_LFRawWhlSpeedV_flg)  "<VAPM_LFRawWhlSpeedV_flg>"
  outpmodule/407(VOUTP_RptMsgReq_flg) -> bus_creator/407
  outpmodule/558(VOUTP_FDCTHCCLVentENSta_flg) -> bus_creator/558
  bus_selector15/4 -> outpmodule/725(VVMC_CCMSASpdWar_flg)  "<VVMC_CCMSASpdWar_flg>"
  bus_selector4/62 -> outpmodule/323(VDDM_DiagRRTSDTC_raw32)  "<VDDM_DiagRRTSDTC_raw32>"
  bus_selector2/10 -> outpmodule/13(VAPM_PASDFMR_cm)  "<VAPM_PASDFMR_cm>"
  outpmodule/187(VOUTP_PosLamp_flg) -> bus_creator/187
  bus_selector3/73 -> outpmodule/238(VBCM_AmbLightColor2_enum)  "<VBCM_AmbLightColor2_enum>"
  bus_selector3/71 -> outpmodule/236(VBCM_AmbLightBrightness3_enum)  "<VBCM_AmbLightBrightness3_enum>"
  bus_selector2/134 -> outpmodule/137(VAPM_AVMparkingcancel_enum)  "<VAPM_AVMparkingcancel_enum>"
  outpmodule/588(VOUTP_RRWheelTemp_C) -> bus_creator/588
  bus_selector9/7 -> outpmodule/466(VSYS_ECU1_cnt)  "<VSYS_ECU1_cnt>"
  outpmodule/717(VOUTP_VehActSpd_kph) -> bus_creator/717
  bus_selector9/31 -> outpmodule/490(VSYS_FdcSlpReqRisingEdge_flg)  "<VSYS_FdcSlpReqRisingEdge_flg>"
  bus_selector3/70 -> outpmodule/235(VBCM_AmbLightBrightness2_enum)  "<VBCM_AmbLightBrightness2_enum>"
  outpmodule/51(VOUTP_LRRawWhlSpeed_kph) -> bus_creator/51
  bus_selector11/87 -> outpmodule/663(VTPM_FlashS1ID_raw)  "<VTPM_FlashS1ID_raw>"
  bus_selector3/81 -> outpmodule/246(VBCM_MFSWTri_flg)  "<VBCM_MFSWTri_flg>"
  outpmodule/591(VOUTP_LRSensorFail_flg) -> bus_creator/591
  bus_selector4/113 -> outpmodule/374(VDDM_RRBatwarnDTC_raw32)  "<VDDM_RRBatwarnDTC_raw32>"
  bus_selector3/74 -> outpmodule/239(VBCM_AmbLightColor3_enum)  "<VBCM_AmbLightColor3_enum>"
  outpmodule/625(VOUTP_S4L_enum) -> bus_creator/625
  bus_selector3/69 -> outpmodule/234(VBCM_AmbLightBrightness1_enum)  "<VBCM_AmbLightBrightness1_enum>"
  bus_selector3/68 -> outpmodule/233(VBCM_AmbLightBreath3_flg)  "<VBCM_AmbLightBreath3_flg>"
  bus_selector12/35 -> outpmodule/708(VTQD_RrUdcMin_V)  "<VTQD_RrUdcMin_V>"
  outpmodule/516(VOUTP_EDriveMode_enum) -> bus_creator/516
  bus_selector3/67 -> outpmodule/232(VBCM_AmbLightBreath2_flg)  "<VBCM_AmbLightBreath2_flg>"
  outpmodule/400(VOUTP_AllCANTxReq_flg) -> bus_creator/400
  bus_selector11/9 -> outpmodule/585(VTPM_LFWheelTemp_C)  "<VTPM_LFWheelTemp_C>"
  bus_selector11/8 -> outpmodule/584(VTPM_RRWheelPress_raw8)  "<VTPM_RRWheelPress_raw8>"
  outpmodule/441(VOUTP_LVBattChrgTimeCnt_s) -> bus_creator/441
  bus_selector11/7 -> outpmodule/583(VTPM_LRWheelPress_raw8)  "<VTPM_LRWheelPress_raw8>"
  bus_selector2/13 -> outpmodule/16(VAPM_PASDFCL_cm)  "<VAPM_PASDFCL_cm>"
  outpmodule/478(VOUTP_Change1_cnt) -> bus_creator/478
  outpmodule/533(VOUTP_ACSubMode_enum) -> bus_creator/533
  outpmodule/434(VOUTP_LowSOCWarn_enum) -> bus_creator/434
  bus_selector3/55 -> outpmodule/220(VBCM_User4IPAmbLightBrightness_enum)  "<VBCM_User4IPAmbLightBrightness_enum>"
  bus_selector11/6 -> outpmodule/582(VTPM_RFWheelPress_raw8)  "<VTPM_RFWheelPress_raw8>"
  bus_selector8/7 -> outpmodule/418(VPMM_DCDCVoltSetpoint_V)  "<VPMM_DCDCVoltSetpoint_V>"
  outpmodule/145(VOUTP_IVIStatus_flg) -> bus_creator/145
  bus_selector11/5 -> outpmodule/581(VTPM_LFWheelPress_raw8)  "<VTPM_LFWheelPress_raw8>"
  bus_selector11/4 -> outpmodule/580(VTPM_RRBatWarn_flg)  "<VTPM_RRBatWarn_flg>"
  outpmodule/459(VOUTP_OTAPwrReqStdChkSta_enum) -> bus_creator/459
  outpmodule/122(VOUTP_BrkSwStaTimeOut_flg) -> bus_creator/122
  bus_selector2/23 -> outpmodule/26(VAPM_PASAFMR_enum)  "<VAPM_PASAFMR_enum>"
  bus_selector11/2 -> outpmodule/578(VTPM_RFBatWarn_flg)  "<VTPM_RFBatWarn_flg>"
  BDKC_outputs/1 -> bus_selector6/1
  outpmodule/473(VOUTP_Patch2_cnt) -> bus_creator/473
  bus_selector2/157 -> outpmodule/160(VAPM_APSHWVer_enum)  "<VAPM_APSHWVer_enum>"
  bus_selector11/1 -> outpmodule/577(VTPM_LFBatWarn_flg)  "<VTPM_LFBatWarn_flg>"
  outpmodule/453(VOUTP_HWResetSta_enum) -> bus_creator/453
  bus_selector11/57 -> outpmodule/633(VTPM_S1WheelDebugALTU_pct)  "<VTPM_S1WheelDebugALTU_pct>"
  bus_selector4/10 -> outpmodule/271(VDDM_C3CCU2RCDTC_raw32)  "<VDDM_C3CCU2RCDTC_raw32>"
  bus_selector12/37 -> outpmodule/710(VTQD_ReBrakeLPReq_flg)  "<VTQD_ReBrakeLPReq_flg>"
  bus_selector7/5 -> outpmodule/404(VNMM_ErrorState_enum)  "<VNMM_ErrorState_enum>"
  bus_selector11/83 -> outpmodule/659(VTPM_Flashdatavalid_enum)  "<VTPM_Flashdatavalid_enum>"
  bus_selector11/56 -> outpmodule/632(VTPM_IDin_raw32)  "<VTPM_IDin_raw32>"
  bus_selector11/54 -> outpmodule/630(VTPM_RRP20_raw8)  "<VTPM_RRP20_raw8>"
  bus_selector5/3 -> outpmodule/397(VDHP_EAPS2MIN_pct)  "<VDHP_EAPS2MIN_pct>"
  bus_selector11/55 -> outpmodule/631(VTPM_FAT_flg)  "<VTPM_FAT_flg>"
  bus_selector11/63 -> outpmodule/639(VTPM_ID3messageALTU_raw8)  "<VTPM_ID3messageALTU_raw8>"
  bus_selector11/53 -> outpmodule/629(VTPM_LRP20_raw8)  "<VTPM_LRP20_raw8>"
  outpmodule/534(VOUTP_FDRecyAutoCmd_enum) -> bus_creator/534
  outpmodule/109(VOUTP_LongAccel_Gps) -> bus_creator/109
  outpmodule/457(VOUTP_PwrReq_OTA_enum) -> bus_creator/457
  outpmodule/367(VOUTP_ESC5RCErrDTC_raw32) -> bus_creator/367
  bus_selector11/52 -> outpmodule/628(VTPM_RFP20_raw8)  "<VTPM_RFP20_raw8>"
  outpmodule/685(VOUTP_RrRgnDecrSta_flg) -> bus_creator/685
  outpmodule/186(VOUTP_DimmerEN_flg) -> bus_creator/186
  bus_selector11/51 -> outpmodule/627(VTPM_LFP20_raw8)  "<VTPM_LFP20_raw8>"
  bus_selector12/42 -> outpmodule/715(VTQD_IVIPwrLockSta_enum)  "<VTQD_IVIPwrLockSta_enum>"
  bus_selector11/50 -> outpmodule/626(VTPM_ALFin_flg)  "<VTPM_ALFin_flg>"
  bus_selector2/26 -> outpmodule/29(VAPM_USSStaRMR_flg)  "<VAPM_USSStaRMR_flg>"
  outpmodule/312(VOUTP_MCUF1NoComDTC_raw32) -> bus_creator/312
  bus_selector11/47 -> outpmodule/623(VTPM_S2L_enum)  "<VTPM_S2L_enum>"
  outpmodule/2(VOUTP_LVBattVoltSta_enum) -> bus_creator/2
  bus_selector11/49 -> outpmodule/625(VTPM_S4L_enum)  "<VTPM_S4L_enum>"
  outpmodule/462(VOUTP_HWVer3_cnt) -> bus_creator/462
  bus_selector2/103 -> outpmodule/106(VAPM_YawRateTimeOut_flg)  "<VAPM_YawRateTimeOut_flg>"
  bus_selector11/48 -> outpmodule/624(VTPM_S3L_enum)  "<VTPM_S3L_enum>"
  bus_selector11/44 -> outpmodule/620(VTPM_S3ID_raw32)  "<VTPM_S3ID_raw32>"
  bus_selector2/50 -> outpmodule/53(VAPM_RRRawWhlSpeed_kph)  "<VAPM_RRRawWhlSpeed_kph>"
  bus_selector11/46 -> outpmodule/622(VTPM_S1L_enum)  "<VTPM_S1L_enum>"
  bus_selector4/118 -> outpmodule/379(VDDM_LFWheelTmpHighDTC_raw32)  "<VDDM_LFWheelTmpHighDTC_raw32>"
  bus_selector9/28 -> outpmodule/487(VSYS_SHA7_cnt)  "<VSYS_SHA7_cnt>"
  outpmodule/579(VOUTP_LRBatWarn_flg) -> bus_creator/579
  bus_selector4/122 -> outpmodule/383(VDDM_LFSensorFailDTC_raw32)  "<VDDM_LFSensorFailDTC_raw32>"
  bus_selector11/45 -> outpmodule/621(VTPM_S4ID_raw32)  "<VTPM_S4ID_raw32>"
  bus_selector11/41 -> outpmodule/617(VTPM_RRSensorMode_flg)  "<VTPM_RRSensorMode_flg>"
  bus_selector8/48 -> outpmodule/459(VPMM_OTAPwrReqStdChkSta_enum)  "<VPMM_OTAPwrReqStdChkSta_enum>"
  outpmodule/311(VOUTP_APSCorrErrDTC_raw32) -> bus_creator/311
  bus_selector12/38 -> outpmodule/711(VTQD_CreepON_flg)  "<VTQD_CreepON_flg>"
  outpmodule/721(VOUTP_ReqV2LIVIPopup_enum) -> bus_creator/721
  outpmodule/484(VOUTP_SHA4_cnt) -> bus_creator/484
  bus_selector11/43 -> outpmodule/619(VTPM_S2ID_raw32)  "<VTPM_S2ID_raw32>"
  outpmodule/170(VOUTP_BCMDoorLockSta_flg) -> bus_creator/170
  bus_selector11/42 -> outpmodule/618(VTPM_S1ID_raw32)  "<VTPM_S1ID_raw32>"
  bus_selector8/36 -> outpmodule/447(VPMM_LVSilentChrgReq_flg)  "<VPMM_LVSilentChrgReq_flg>"
  outpmodule/199(VOUTP_RTurnLP_flg) -> bus_creator/199
  bus_selector12/15 -> outpmodule/688(VTQD_FrEDUActTq_Nm)  "<VTQD_FrEDUActTq_Nm>"
  bus_selector11/40 -> outpmodule/616(VTPM_LRSensorMode_flg)  "<VTPM_LRSensorMode_flg>"
  outpmodule/313(VOUTP_MCUR1NoComDTC_raw32) -> bus_creator/313
  bus_selector4/32 -> outpmodule/293(VDDM_MCUDisDTC_raw32)  "<VDDM_MCUDisDTC_raw32>"
  outpmodule/327(VOUTP_FCRUSSDTC_raw32) -> bus_creator/327
  outpmodule/624(VOUTP_S3L_enum) -> bus_creator/624
  bus_selector11/38 -> outpmodule/614(VTPM_LFSensorMode_flg)  "<VTPM_LFSensorMode_flg>"
  outpmodule/58(VOUTP_RFRawWhlSpeedVTimeOut_flg) -> bus_creator/58
  outpmodule/85(VOUTP_RRPulseCount_enum) -> bus_creator/85
  bus_selector2/137 -> outpmodule/140(VAPM_AVMparkingexcuteTimeOut_flg)  "<VAPM_AVMparkingexcuteTimeOut_flg>"
  bus_selector11/39 -> outpmodule/615(VTPM_RFSensorMode_flg)  "<VTPM_RFSensorMode_flg>"
  outpmodule/530(VOUTP_sigCbnSolarRight_W) -> bus_creator/530
  bus_selector11/34 -> outpmodule/610(VTPM_RFWheelPSW_raw8)  "<VTPM_RFWheelPSW_raw8>"
  bus_selector11/3 -> outpmodule/579(VTPM_LRBatWarn_flg)  "<VTPM_LRBatWarn_flg>"
  bus_selector8/39 -> outpmodule/450(VPMM_CtrlFrRC1_flg)  "<VPMM_CtrlFrRC1_flg>"
  outpmodule/126(VOUTP_ESCStandstillTimeOut_flg) -> bus_creator/126
  bus_selector11/35 -> outpmodule/611(VTPM_RRWheelPSW_raw8)  "<VTPM_RRWheelPSW_raw8>"
  bus_selector4/92 -> outpmodule/353(VDDM_ACCMalfuncDetDTC_raw32)  "<VDDM_ACCMalfuncDetDTC_raw32>"
  bus_selector2/18 -> outpmodule/21(VAPM_PASAFCL_enum)  "<VAPM_PASAFCL_enum>"
  bus_selector11/32 -> outpmodule/608(VTPM_LFWheelPSW_raw8)  "<VTPM_LFWheelPSW_raw8>"
  outpmodule/506(VOUTP_CoolgFanActDuty_pct) -> bus_creator/506
  outpmodule/29(VOUTP_USSStaRMR_flg) -> bus_creator/29
  bus_selector2/155 -> outpmodule/158(VAPM_APSRQDisplay_enum)  "<VAPM_APSRQDisplay_enum>"
  bus_selector11/30 -> outpmodule/606(VTPM_LRWheelTmpIndi_flg)  "<VTPM_LRWheelTmpIndi_flg>"
  bus_selector3/17 -> outpmodule/182(VBCM_CTDCtrl_enum)  "<VBCM_CTDCtrl_enum>"
  outpmodule/185(VOUTP_Dimmer_pct) -> bus_creator/185
  outpmodule/14(VOUTP_PASDFML_cm) -> bus_creator/14
  bus_selector2/31 -> outpmodule/34(VAPM_USSStaRCL_flg)  "<VAPM_USSStaRCL_flg>"
  bus_selector11/28 -> outpmodule/604(VTPM_LFWheelTmpIndi_flg)  "<VTPM_LFWheelTmpIndi_flg>"
  outpmodule/401(VOUTP_NMmTxReq_flg) -> bus_creator/401
  outpmodule/70(VOUTP_RRWhlRotDirTimeOut_flg) -> bus_creator/70
  outpmodule/607(VOUTP_RRWheelTmpIndi_flg) -> bus_creator/607
  bus_selector11/26 -> outpmodule/602(VTPM_RRPressIndi_enum)  "<VTPM_RRPressIndi_enum>"
  outpmodule/212(VOUTP_WiperFixMode_flg) -> bus_creator/212
  outpmodule/626(VOUTP_ALFin_flg) -> bus_creator/626
  outpmodule/60(VOUTP_LRRawWhlSpeedVTimeOut_flg) -> bus_creator/60
  bus_selector2/92 -> outpmodule/95(VAPM_SASSpeed_degps)  "<VAPM_SASSpeed_degps>"
  bus_selector9/4 -> outpmodule/463(VSYS_CarModel1_cnt)  "<VSYS_CarModel1_cnt>"
  bus_selector11/25 -> outpmodule/601(VTPM_LRPressIndi_enum)  "<VTPM_LRPressIndi_enum>"
  outpmodule/377(VOUTP_LRPressIndiDTC_raw32) -> bus_creator/377
  outpmodule/479(VOUTP_Change2_cnt) -> bus_creator/479
  outpmodule/294(VOUTP_DCDCDisDTC_raw32) -> bus_creator/294
  bus_selector11/23 -> outpmodule/599(VTPM_LFPressIndi_enum)  "<VTPM_LFPressIndi_enum>"
  outpmodule/346(VOUTP_ZoneSCPNoComDTC_raw32) -> bus_creator/346
  bus_selector2/82 -> outpmodule/85(VAPM_RRPulseCount_enum)  "<VAPM_RRPulseCount_enum>"
  outpmodule/423(VOUTP_HVPwrSta_flg) -> bus_creator/423
  bus_selector11/24 -> outpmodule/600(VTPM_RFPressIndi_enum)  "<VTPM_RFPressIndi_enum>"
  outpmodule/160(VOUTP_APSHWVer_enum) -> bus_creator/160
  bus_selector11/19 -> outpmodule/595(VTPM_RFWheelDebug_flg)  "<VTPM_RFWheelDebug_flg>"
  bus_selector2/135 -> outpmodule/138(VAPM_AVMparkingcancelTimeOut_flg)  "<VAPM_AVMparkingcancelTimeOut_flg>"
  bus_selector12/20 -> outpmodule/693(VTQD_RrEDUSpd_rpm)  "<VTQD_RrEDUSpd_rpm>"
  outpmodule/492(VOUTP_PmicBootReason_enum) -> bus_creator/492
  bus_selector4/87 -> outpmodule/348(VDDM_FCMACCSigErrDetDTC_raw32)  "<VDDM_FCMACCSigErrDetDTC_raw32>"
  bus_selector11/18 -> outpmodule/594(VTPM_LRWheelDebug_flg)  "<VTPM_LRWheelDebug_flg>"
  bus_selector2/38 -> outpmodule/41(VAPM_Chime_enum)  "<VAPM_Chime_enum>"
  outpmodule/623(VOUTP_S2L_enum) -> bus_creator/623
  outpmodule/287(VOUTP_DCDC4PreDTC_raw32) -> bus_creator/287
  outpmodule/688(VOUTP_FrEDUActTq_Nm) -> bus_creator/688
  bus_selector3/28 -> outpmodule/193(VBCM_LDRL_flg)  "<VBCM_LDRL_flg>"
  bus_selector11/21 -> outpmodule/597(VTPM_TPMSResButtAllow_flg)  "<VTPM_TPMSResButtAllow_flg>"
  outpmodule/306(VOUTP_HoodSWDTC_raw32) -> bus_creator/306
  bus_selector12/2 -> outpmodule/675(VTQD_TqSourceFr_enum)  "<VTQD_TqSourceFr_enum>"
  bus_selector11/11 -> outpmodule/587(VTPM_LRWheelTemp_C)  "<VTPM_LRWheelTemp_C>"
  outpmodule/541(VOUTP_CCUSyncSts_flg) -> bus_creator/541
  outpmodule/209(VOUTP_FrWiperH_flg) -> bus_creator/209
  bus_selector3/63 -> outpmodule/228(VBCM_User4AmbLightColor_enum)  "<VBCM_User4AmbLightColor_enum>"
  outpmodule/650(VOUTP_WriteChkLFID_raw) -> bus_creator/650
  bus_selector11/66 -> outpmodule/642(VTPM_SetIDLoc_flg)  "<VTPM_SetIDLoc_flg>"
  bus_selector7/4 -> outpmodule/403(VNMM_CSB_flg)  "<VNMM_CSB_flg>"
  BAPM_outputs/1 -> bus_selector2/1
  bus_selector11/59 -> outpmodule/635(VTPM_S3WheelDebugALTU_pct)  "<VTPM_S3WheelDebugALTU_pct>"
  outpmodule/357(VOUTP_MCUF1RCErrDTC_raw32) -> bus_creator/357
  bus_selector11/85 -> outpmodule/661(VTPM_unlearnSfailvalid_enum)  "<VTPM_unlearnSfailvalid_enum>"
  outpmodule/406(VOUTP_PNI_flg) -> bus_creator/406
  outpmodule/299(VOUTP_LVSupLoDTC_raw32) -> bus_creator/299
  bus_selector11/27 -> outpmodule/603(VTPM_TPMSWarnIndi_enum)  "<VTPM_TPMSWarnIndi_enum>"
  bus_selector7/6 -> outpmodule/405(VNMM_NodeID_enum)  "<VNMM_NodeID_enum>"
  outpmodule/425(VOUTP_FrMCUEnaReq_flg) -> bus_creator/425
  outpmodule/301(VOUTP_DrStSWDTC_raw32) -> bus_creator/301
  bus_selector11/12 -> outpmodule/588(VTPM_RRWheelTemp_C)  "<VTPM_RRWheelTemp_C>"
  bus_selector11/31 -> outpmodule/607(VTPM_RRWheelTmpIndi_flg)  "<VTPM_RRWheelTmpIndi_flg>"
  outpmodule/205(VOUTP_RoomLampL_flg) -> bus_creator/205
  outpmodule/638(VOUTP_ID2messageALTU_raw8) -> bus_creator/638
  bus_selector2/55 -> outpmodule/58(VAPM_RFRawWhlSpeedVTimeOut_flg)  "<VAPM_RFRawWhlSpeedVTimeOut_flg>"
  bus_selector11/84 -> outpmodule/660(VTPM_unlearnSfali_flg)  "<VTPM_unlearnSfali_flg>"
  outpmodule/405(VOUTP_NodeID_enum) -> bus_creator/405
  bus_selector11/14 -> outpmodule/590(VTPM_RFSensorFail_flg)  "<VTPM_RFSensorFail_flg>"
  bus_selector2/37 -> outpmodule/40(VAPM_USSStaFCL_flg)  "<VAPM_USSStaFCL_flg>"
  outpmodule/360(VOUTP_MCUR1CSErrDTC_raw32) -> bus_creator/360
  bus_selector9/10 -> outpmodule/469(VSYS_Major2_cnt)  "<VSYS_Major2_cnt>"
  outpmodule/412(VOUTP_PowerUpState_enum) -> bus_creator/412
  outpmodule/424(VOUTP_SysPowerMode_enum) -> bus_creator/424
  bus_selector4/93 -> outpmodule/354(VDDM_CCMalfuncDetDTC_raw32)  "<VDDM_CCMalfuncDetDTC_raw32>"
  outpmodule/531(VOUTP_sigAmbAirT_C) -> bus_creator/531
  outpmodule/40(VOUTP_USSStaFCL_flg) -> bus_creator/40
  bus_selector11/29 -> outpmodule/605(VTPM_RFWheelTmpIndi_flg)  "<VTPM_RFWheelTmpIndi_flg>"
  outpmodule/421(VOUTP_PowerSta_enum) -> bus_creator/421
  bus_selector11/60 -> outpmodule/636(VTPM_S4WheelDebugALTU_pct)  "<VTPM_S4WheelDebugALTU_pct>"
  bus_selector3/60 -> outpmodule/225(VBCM_User1AmbLightColor_enum)  "<VBCM_User1AmbLightColor_enum>"
  outpmodule/368(VOUTP_ESC5CSErrDTC_raw32) -> bus_creator/368
  bus_selector2/44 -> outpmodule/47(VAPM_LFRawWhlSpeed_kph)  "<VAPM_LFRawWhlSpeed_kph>"
  outpmodule/636(VOUTP_S4WheelDebugALTU_pct) -> bus_creator/636
  outpmodule/417(VOUTP_DCDCEnaReq_flg) -> bus_creator/417
  bus_selector11/36 -> outpmodule/612(VTPM_CWheelTips_enum)  "<VTPM_CWheelTips_enum>"
  outpmodule/598(VOUTP_TPMSCaliButtAllow_flg) -> bus_creator/598
  outpmodule/300(VOUTP_LVSupHiDTC_raw32) -> bus_creator/300
  outpmodule/378(VOUTP_RRPressIndiDTC_raw32) -> bus_creator/378
  outpmodule/302(VOUTP_FLDoorSWDTC_raw32) -> bus_creator/302
  bus_selector10/31 -> outpmodule/526(VTHC_sigSetTempZon2St_C)  "<VTHC_sigSetTempZon2St_C>"
  bus_selector12/9 -> outpmodule/682(VTQD_FrActvDmpDisabReq_flg)  "<VTQD_FrActvDmpDisabReq_flg>"
  bus_selector2/63 -> outpmodule/66(VAPM_RFWhlRotDirTimeOut_flg)  "<VAPM_RFWhlRotDirTimeOut_flg>"
  bus_selector11/20 -> outpmodule/596(VTPM_RRWheelDebug_flg)  "<VTPM_RRWheelDebug_flg>"
  outpmodule/101(VOUTP_SASV_flg) -> bus_creator/101
  outpmodule/730(VOUTP_APSDecReqA_flg) -> bus_creator/730
  outpmodule/709(VOUTP_RrUdcMax_V) -> bus_creator/709
  outpmodule/463(VOUTP_CarModel1_cnt) -> bus_creator/463
  outpmodule/414(VOUTP_PowerUpFault_enum) -> bus_creator/414
  outpmodule/526(VOUTP_sigSetTempZon2St_C) -> bus_creator/526
  outpmodule/391(VOUTP_EPBUnlockTODTC_raw32) -> bus_creator/391
  bus_selector2/107 -> outpmodule/110(VAPM_LongAccelTimeOut_flg)  "<VAPM_LongAccelTimeOut_flg>"
  outpmodule/156(VOUTP_DriverSeatBeltCmdTimeOut_flg) -> bus_creator/156
  outpmodule/390(VOUTP_EPBLockTODTC_raw32) -> bus_creator/390
  bus_selector11/22 -> outpmodule/598(VTPM_TPMSCaliButtAllow_flg)  "<VTPM_TPMSCaliButtAllow_flg>"
  BTPM_outputs/1 -> bus_selector11/1
  bus_selector11/33 -> outpmodule/609(VTPM_LRWheelPSW_raw8)  "<VTPM_LRWheelPSW_raw8>"
  outpmodule/559(VOUTP_FDCTHCPsEVentYSta_enum) -> bus_creator/559
  outpmodule/179(VOUTP_FrChargingDoorCtrl_enum) -> bus_creator/179
  outpmodule/389(VOUTP_5vAPS2PwrErrDTC_raw32) -> bus_creator/389
  outpmodule/349(VOUTP_FrMCUSigErrDetDTC_raw32) -> bus_creator/349
  bus_selector2/149 -> outpmodule/152(VAPM_ABSActiveTimeOut_flg)  "<VAPM_ABSActiveTimeOut_flg>"
  bus_selector11/15 -> outpmodule/591(VTPM_LRSensorFail_flg)  "<VTPM_LRSensorFail_flg>"
  bus_selector11/13 -> outpmodule/589(VTPM_LFSensorFail_flg)  "<VTPM_LFSensorFail_flg>"
  outpmodule/387(VOUTP_C1EPAS2LCDTC_raw32) -> bus_creator/387
  outpmodule/386(VOUTP_RRSensorFailDTC_raw32) -> bus_creator/386
  outpmodule/415(VOUTP_PowerDownFault_enum) -> bus_creator/415
  outpmodule/385(VOUTP_LRSensorFailDTC_raw32) -> bus_creator/385
  bus_selector2/99 -> outpmodule/102(VAPM_SASVTimeOut_flg)  "<VAPM_SASVTimeOut_flg>"
  bus_selector8/6 -> outpmodule/417(VPMM_DCDCEnaReq_flg)  "<VPMM_DCDCEnaReq_flg>"
  bus_selector11/37 -> outpmodule/613(VTPM_AutoLTips_enum)  "<VTPM_AutoLTips_enum>"
  outpmodule/384(VOUTP_RFSensorFailDTC_raw32) -> bus_creator/384
  bus_selector11/65 -> outpmodule/641(VTPM_Chkfin_flg)  "<VTPM_Chkfin_flg>"
  bus_selector2/46 -> outpmodule/49(VAPM_RFRawWhlSpeed_kph)  "<VAPM_RFRawWhlSpeed_kph>"
  outpmodule/404(VOUTP_ErrorState_enum) -> bus_creator/404
  outpmodule/383(VOUTP_LFSensorFailDTC_raw32) -> bus_creator/383
  outpmodule/381(VOUTP_LRWheelTmpHighDTC_raw32) -> bus_creator/381
  outpmodule/380(VOUTP_RFWheelTmpHighDTC_raw32) -> bus_creator/380
  bus_selector2/5 -> outpmodule/8(VAPM_ChrgPlugSta_enum)  "<VAPM_ChrgPlugSta_enum>"
  bus_selector2/120 -> outpmodule/123(VAPM_BrkSwV_flg)  "<VAPM_BrkSwV_flg>"
  bus_selector15/6 -> outpmodule/727(VVMC_APSCtrlAvail_flg)  "<VVMC_APSCtrlAvail_flg>"
  outpmodule/712(VOUTP_EquivAccPedalSWSta_flg) -> bus_creator/712
  outpmodule/454(VOUTP_CtrlDrPwrStbA2_flg) -> bus_creator/454
  bus_selector12/25 -> outpmodule/698(VTQD_RgnAbnorSta_flg)  "<VTQD_RgnAbnorSta_flg>"
  outpmodule/163(VOUTP_APSVRqEPASCtrl_flg) -> bus_creator/163
  outpmodule/513(VOUTP_FDRrAPTCHeatPwrCmd_W) -> bus_creator/513
  bus_selector11/16 -> outpmodule/592(VTPM_RRSensorFail_flg)  "<VTPM_RRSensorFail_flg>"
  bus_selector11/10 -> outpmodule/586(VTPM_RFWheelTemp_C)  "<VTPM_RFWheelTemp_C>"
  bus_selector2/123 -> outpmodule/126(VAPM_ESCStandstillTimeOut_flg)  "<VAPM_ESCStandstillTimeOut_flg>"
  outpmodule/570(VOUTP_FDCFGSAirIntCmd_enum) -> bus_creator/570
  bus_selector11/94 -> outpmodule/670(VTPM_LProgress_enum)  "<VTPM_LProgress_enum>"
  bus_selector2/28 -> outpmodule/31(VAPM_USSStaRLR_flg)  "<VAPM_USSStaRLR_flg>"
  bus_selector9/35 -> outpmodule/494(VSYS_AcoreRebootCmdACK_flg)  "<VSYS_AcoreRebootCmdACK_flg>"
  outpmodule/379(VOUTP_LFWheelTmpHighDTC_raw32) -> bus_creator/379
  outpmodule/206(VOUTP_TrunkRel_flg) -> bus_creator/206
  outpmodule/593(VOUTP_LFWheelDebug_flg) -> bus_creator/593
  outpmodule/382(VOUTP_RRWheelTmpHighDTC_raw32) -> bus_creator/382
  bus_selector9/23 -> outpmodule/482(VSYS_SHA2_cnt)  "<VSYS_SHA2_cnt>"
  outpmodule/584(VOUTP_RRWheelPress_raw8) -> bus_creator/584
  bus_selector11/17 -> outpmodule/593(VTPM_LFWheelDebug_flg)  "<VTPM_LFWheelDebug_flg>"
  outpmodule/3(VOUTP_VehHVPwrAvail4THCM_W) -> bus_creator/3
  bus_selector2/100 -> outpmodule/103(VAPM_GRADE_Deg)  "<VAPM_GRADE_Deg>"
  outpmodule/13(VOUTP_PASDFMR_cm) -> bus_creator/13
  outpmodule/419(VOUTP_HVBatCnctReq_flg) -> bus_creator/419
  outpmodule/408(VOUTP_WakeUp_enum) -> bus_creator/408
  bus_selector2/11 -> outpmodule/14(VAPM_PASDFML_cm)  "<VAPM_PASDFML_cm>"
  bus_selector2/29 -> outpmodule/32(VAPM_USSStaRLL_flg)  "<VAPM_USSStaRLL_flg>"
  outpmodule/330(VOUTP_RMRUSSDTC_raw32) -> bus_creator/330
  bus_selector11/58 -> outpmodule/634(VTPM_S2WheelDebugALTU_pct)  "<VTPM_S2WheelDebugALTU_pct>"
  bus_selector8/47 -> outpmodule/458(VPMM_OTAPwrReqOFFChkSta_enum)  "<VPMM_OTAPwrReqOFFChkSta_enum>"
  outpmodule/388(VOUTP_5vAPS1PwrErrDTC_raw32) -> bus_creator/388
  bus_selector10/58 -> outpmodule/553(VTHC_FDCTHCPsEVentZSta_enum)  "<VTHC_FDCTHCPsEVentZSta_enum>"
  bus_selector4/8 -> outpmodule/269(VDDM_C3CCU1CSDTC_raw32)  "<VDDM_C3CCU1CSDTC_raw32>"
  outpmodule/617(VOUTP_RRSensorMode_flg) -> bus_creator/617
  bus_selector2/35 -> outpmodule/38(VAPM_USSStaFLL_flg)  "<VAPM_USSStaFLL_flg>"
  bus_selector11/62 -> outpmodule/638(VTPM_ID2messageALTU_raw8)  "<VTPM_ID2messageALTU_raw8>"
  bus_selector3/12 -> outpmodule/177(VBCM_RRDoorSW_flg)  "<VBCM_RRDoorSW_flg>"
  outpmodule/174(VOUTP_DrDoorSW_flg) -> bus_creator/174
  bus_selector12/18 -> outpmodule/691(VTQD_RrEDURolRgnTq_Nm)  "<VTQD_RrEDURolRgnTq_Nm>"
  bus_selector11/61 -> outpmodule/637(VTPM_ID1messageALTU_raw8)  "<VTPM_ID1messageALTU_raw8>"
  outpmodule/290(VOUTP_DCDCEnaDTC_raw32) -> bus_creator/290
  outpmodule/468(VOUTP_Major1_cnt) -> bus_creator/468
  bus_selector4/88 -> outpmodule/349(VDDM_FrMCUSigErrDetDTC_raw32)  "<VDDM_FrMCUSigErrDetDTC_raw32>"
